simulink library "outp"  (R2021b)
(part 9 of 10)

  VAPM_PASDRML_cm/1 -> VAPM_PASDRML_cm_Inproc/1  "VAPM_PASDRML_cm"
  VAPM_PASDRML_cm_Inproc/1 -> UnitConverter22/1
  UnitConverter22/1 -> VOUTP_PASDRML_cm/1  "VOUTP_PASDRML_cm"
  VAPM_PASDRCR_cm/1 -> VAPM_PASDRCR_cm_Inproc/1  "VAPM_PASDRCR_cm"
  VAPM_PASDRCR_cm_Inproc/1 -> UnitConverter23/1
  UnitConverter23/1 -> VOUTP_PASDRCR_cm/1  "VOUTP_PASDRCR_cm"
  VAPM_PASDRCL_cm/1 -> VAPM_PASDRCL_cm_Inproc/1  "VAPM_PASDRCL_cm"
  VAPM_PASDRCL_cm_Inproc/1 -> UnitConverter24/1
  UnitConverter24/1 -> VOUTP_PASDRCL_cm/1  "VOUTP_PASDRCL_cm"
  VAPM_PASDFMR_cm/1 -> VAPM_PASDFMR_cm_Inproc/1  "VAPM_PASDFMR_cm"
  VAPM_PASDFMR_cm_Inproc/1 -> UnitConverter25/1
  UnitConverter25/1 -> VOUTP_PASDFMR_cm/1  "VOUTP_PASDFMR_cm"
  VAPM_PASDFML_cm/1 -> VAPM_PASDFML_cm_Inproc/1  "VAPM_PASDFML_cm"
  VAPM_PASDFML_cm_Inproc/1 -> UnitConverter26/1
  UnitConverter26/1 -> VOUTP_PASDFML_cm/1  "VOUTP_PASDFML_cm"
  VAPM_PASDFCR_cm/1 -> VAPM_PASDFCR_cm_Inproc/1  "VAPM_PASDFCR_cm"
  VAPM_PASDFCR_cm_Inproc/1 -> UnitConverter27/1
  UnitConverter27/1 -> VOUTP_PASDFCR_cm/1  "VOUTP_PASDFCR_cm"
  VAPM_PASDFCL_cm/1 -> VAPM_PASDFCL_cm_Inproc/1  "VAPM_PASDFCL_cm"
  VAPM_PASDFCL_cm_Inproc/1 -> UnitConverter28/1
  UnitConverter28/1 -> VOUTP_PASDFCL_cm/1  "VOUTP_PASDFCL_cm"
  VAPM_APSDRLR_cm/1 -> VAPM_APSDRLR_cm_Inproc/1  "VAPM_APSDRLR_cm"
  VAPM_APSDRLR_cm_Inproc/1 -> UnitConverter29/1
  UnitConverter29/1 -> VOUTP_APSDRLR_cm/1  "VOUTP_APSDRLR_cm"
  VAPM_APSDRLL_cm/1 -> VAPM_APSDRLL_cm_Inproc/1  "VAPM_APSDRLL_cm"
  VAPM_APSDRLL_cm_Inproc/1 -> UnitConverter30/1
  UnitConverter30/1 -> VOUTP_APSDRLL_cm/1  "VOUTP_APSDRLL_cm"
  VAPM_APSDFLR_cm/1 -> VAPM_APSDFLR_cm_Inproc/1  "VAPM_APSDFLR_cm"
  VAPM_APSDFLR_cm_Inproc/1 -> UnitConverter31/1
  UnitConverter31/1 -> VOUTP_APSDFLR_cm/1  "VOUTP_APSDFLR_cm"
  VAPM_APSDFLL_cm/1 -> VAPM_APSDFLL_cm_Inproc/1  "VAPM_APSDFLL_cm"
  VAPM_APSDFLL_cm_Inproc/1 -> UnitConverter32/1
  UnitConverter32/1 -> VOUTP_APSDFLL_cm/1  "VOUTP_APSDFLL_cm"
  VAPM_PASAFCL_enum/1 -> VAPM_PASAFCL_enum_Inproc/1  "VAPM_PASAFCL_enum"
  VAPM_PASAFCL_enum_Inproc/1 -> UnitConverter33/1
  UnitConverter33/1 -> VOUTP_PASAFCL_enum/1  "VOUTP_PASAFCL_enum"
  VAPM_PASARMR_enum/1 -> VAPM_PASARMR_enum_Inproc/1  "VAPM_PASARMR_enum"
  VAPM_PASARMR_enum_Inproc/1 -> UnitConverter34/1
  UnitConverter34/1 -> VOUTP_PASARMR_enum/1  "VOUTP_PASARMR_enum"
  VAPM_PASARML_enum/1 -> VAPM_PASARML_enum_Inproc/1  "VAPM_PASARML_enum"
  VAPM_PASARML_enum_Inproc/1 -> UnitConverter35/1
  UnitConverter35/1 -> VOUTP_PASARML_enum/1  "VOUTP_PASARML_enum"
  VAPM_PASARCR_enum/1 -> VAPM_PASARCR_enum_Inproc/1  "VAPM_PASARCR_enum"
  VAPM_PASARCR_enum_Inproc/1 -> UnitConverter36/1
  UnitConverter36/1 -> VOUTP_PASARCR_enum/1  "VOUTP_PASARCR_enum"
  VAPM_PASARCL_enum/1 -> VAPM_PASARCL_enum_Inproc/1  "VAPM_PASARCL_enum"
  VAPM_PASARCL_enum_Inproc/1 -> UnitConverter37/1
  UnitConverter37/1 -> VOUTP_PASARCL_enum/1  "VOUTP_PASARCL_enum"
  VAPM_PASAFMR_enum/1 -> VAPM_PASAFMR_enum_Inproc/1  "VAPM_PASAFMR_enum"
  VAPM_PASAFMR_enum_Inproc/1 -> UnitConverter38/1
  UnitConverter38/1 -> VOUTP_PASAFMR_enum/1  "VOUTP_PASAFMR_enum"
  VAPM_PASAFML_enum/1 -> VAPM_PASAFML_enum_Inproc/1  "VAPM_PASAFML_enum"
  VAPM_PASAFML_enum_Inproc/1 -> UnitConverter39/1
  UnitConverter39/1 -> VOUTP_PASAFML_enum/1  "VOUTP_PASAFML_enum"
  VAPM_PASAFCR_enum/1 -> VAPM_PASAFCR_enum_Inproc/1  "VAPM_PASAFCR_enum"
  VAPM_PASAFCR_enum_Inproc/1 -> UnitConverter40/1
  UnitConverter40/1 -> VOUTP_PASAFCR_enum/1  "VOUTP_PASAFCR_enum"
  VAPM_USSStaRMR_flg/1 -> VAPM_USSStaRMR_flg_Inproc/1  "VAPM_USSStaRMR_flg"
  VAPM_USSStaRMR_flg_Inproc/1 -> UnitConverter41/1
  UnitConverter41/1 -> VOUTP_USSStaRMR_flg/1  "VOUTP_USSStaRMR_flg"
  VAPM_USSStaRML_flg/1 -> VAPM_USSStaRML_flg_Inproc/1  "VAPM_USSStaRML_flg"
  VAPM_USSStaRML_flg_Inproc/1 -> UnitConverter42/1
  UnitConverter42/1 -> VOUTP_USSStaRML_flg/1  "VOUTP_USSStaRML_flg"
  VAPM_USSStaRLR_flg/1 -> VAPM_USSStaRLR_flg_Inproc/1  "VAPM_USSStaRLR_flg"
  VAPM_USSStaRLR_flg_Inproc/1 -> UnitConverter43/1
  UnitConverter43/1 -> VOUTP_USSStaRLR_flg/1  "VOUTP_USSStaRLR_flg"
  VAPM_USSStaRLL_flg/1 -> VAPM_USSStaRLL_flg_Inproc/1  "VAPM_USSStaRLL_flg"
  VAPM_USSStaRLL_flg_Inproc/1 -> UnitConverter44/1
  UnitConverter44/1 -> VOUTP_USSStaRLL_flg/1  "VOUTP_USSStaRLL_flg"
  VAPM_USSStaRCR_flg/1 -> VAPM_USSStaRCR_flg_Inproc/1  "VAPM_USSStaRCR_flg"
  VAPM_USSStaRCR_flg_Inproc/1 -> UnitConverter45/1
  UnitConverter45/1 -> VOUTP_USSStaRCR_flg/1  "VOUTP_USSStaRCR_flg"
  VAPM_USSStaRCL_flg/1 -> VAPM_USSStaRCL_flg_Inproc/1  "VAPM_USSStaRCL_flg"
  VAPM_USSStaRCL_flg_Inproc/1 -> UnitConverter46/1
  UnitConverter46/1 -> VOUTP_USSStaRCL_flg/1  "VOUTP_USSStaRCL_flg"
  VAPM_USSStaFMR_flg/1 -> VAPM_USSStaFMR_flg_Inproc/1  "VAPM_USSStaFMR_flg"
  VAPM_USSStaFMR_flg_Inproc/1 -> UnitConverter47/1
  UnitConverter47/1 -> VOUTP_USSStaFMR_flg/1  "VOUTP_USSStaFMR_flg"
  VAPM_USSStaFML_flg/1 -> VAPM_USSStaFML_flg_Inproc/1  "VAPM_USSStaFML_flg"
  VAPM_USSStaFML_flg_Inproc/1 -> UnitConverter48/1
  UnitConverter48/1 -> VOUTP_USSStaFML_flg/1  "VOUTP_USSStaFML_flg"
  VAPM_USSStaFLR_flg/1 -> VAPM_USSStaFLR_flg_Inproc/1  "VAPM_USSStaFLR_flg"
  VAPM_USSStaFLR_flg_Inproc/1 -> UnitConverter49/1
  UnitConverter49/1 -> VOUTP_USSStaFLR_flg/1  "VOUTP_USSStaFLR_flg"
  VAPM_USSStaFLL_flg/1 -> VAPM_USSStaFLL_flg_Inproc/1  "VAPM_USSStaFLL_flg"
  VAPM_USSStaFLL_flg_Inproc/1 -> UnitConverter50/1
  UnitConverter50/1 -> VOUTP_USSStaFLL_flg/1  "VOUTP_USSStaFLL_flg"
  VAPM_USSStaFCR_flg/1 -> VAPM_USSStaFCR_flg_Inproc/1  "VAPM_USSStaFCR_flg"
  VAPM_USSStaFCR_flg_Inproc/1 -> UnitConverter51/1
  UnitConverter51/1 -> VOUTP_USSStaFCR_flg/1  "VOUTP_USSStaFCR_flg"
  VAPM_USSStaFCL_flg/1 -> VAPM_USSStaFCL_flg_Inproc/1  "VAPM_USSStaFCL_flg"
  VAPM_USSStaFCL_flg_Inproc/1 -> UnitConverter52/1
  UnitConverter52/1 -> VOUTP_USSStaFCL_flg/1  "VOUTP_USSStaFCL_flg"
  VAPM_Chime_enum/1 -> VAPM_Chime_enum_Inproc/1  "VAPM_Chime_enum"
  VAPM_Chime_enum_Inproc/1 -> UnitConverter53/1
  UnitConverter53/1 -> VOUTP_Chime_enum/1  "VOUTP_Chime_enum"
  VAPM_SNSRLayout_enum/1 -> VAPM_SNSRLayout_enum_Inproc/1  "VAPM_SNSRLayout_enum"
  VAPM_SNSRLayout_enum_Inproc/1 -> UnitConverter54/1
  UnitConverter54/1 -> VOUTP_SNSRLayout_enum/1  "VOUTP_SNSRLayout_enum"
  VAPM_StaFSya_flg/1 -> VAPM_StaFSya_flg_Inproc/1  "VAPM_StaFSya_flg"
  VAPM_StaFSya_flg_Inproc/1 -> UnitConverter55/1
  UnitConverter55/1 -> VOUTP_StaFSya_flg/1  "VOUTP_StaFSya_flg"
  VAPM_ModOperation_enum/1 -> VAPM_ModOperation_enum_Inproc/1  "VAPM_ModOperation_enum"
  VAPM_ModOperation_enum_Inproc/1 -> UnitConverter56/1
  UnitConverter56/1 -> VOUTP_ModOperation_enum/1  "VOUTP_ModOperation_enum"
  VAPM_BrkPedalPos_pct/1 -> VAPM_BrkPedalPos_pct_Inproc/1  "VAPM_BrkPedalPos_pct"
  VAPM_BrkPedalPos_pct_Inproc/1 -> UnitConverter57/1
  UnitConverter57/1 -> VOUTP_BrkPedalPos_pct/1  "VOUTP_BrkPedalPos_pct"
  VAPM_BrkPedalPosTimeOut_flg/1 -> VAPM_BrkPedalPosTimeOut_flg_Inproc/1  "VAPM_BrkPedalPosTimeOut_flg"
  VAPM_BrkPedalPosTimeOut_flg_Inproc/1 -> UnitConverter58/1
  UnitConverter58/1 -> VOUTP_BrkPedalPosTimeOut_flg/1  "VOUTP_BrkPedalPosTimeOut_flg"
  VAPM_LFRawWhlSpeed_kph/1 -> VAPM_LFRawWhlSpeed_kph_Inproc/1  "VAPM_LFRawWhlSpeed_kph"
  VAPM_LFRawWhlSpeed_kph_Inproc/1 -> UnitConverter59/1
  UnitConverter59/1 -> VOUTP_LFRawWhlSpeed_kph/1  "VOUTP_LFRawWhlSpeed_kph"
  VAPM_LFRawWhlSpeedTimeOut_flg/1 -> VAPM_LFRawWhlSpeedTimeOut_flg_Inproc/1  "VAPM_LFRawWhlSpeedTimeOut_flg"
  VAPM_LFRawWhlSpeedTimeOut_flg_Inproc/1 -> UnitConverter60/1
  UnitConverter60/1 -> VOUTP_LFRawWhlSpeedTimeOut_flg/1  "VOUTP_LFRawWhlSpeedTimeOut_flg"
  VAPM_RFRawWhlSpeed_kph/1 -> VAPM_RFRawWhlSpeed_kph_Inproc/1  "VAPM_RFRawWhlSpeed_kph"
  VAPM_RFRawWhlSpeed_kph_Inproc/1 -> UnitConverter61/1
  UnitConverter61/1 -> VOUTP_RFRawWhlSpeed_kph/1  "VOUTP_RFRawWhlSpeed_kph"
  VAPM_RFRawWhlSpeedTimeOut_flg/1 -> VAPM_RFRawWhlSpeedTimeOut_flg_Inproc/1  "VAPM_RFRawWhlSpeedTimeOut_flg"
  VAPM_RFRawWhlSpeedTimeOut_flg_Inproc/1 -> UnitConverter62/1
  UnitConverter62/1 -> VOUTP_RFRawWhlSpeedTimeOut_flg/1  "VOUTP_RFRawWhlSpeedTimeOut_flg"
  VAPM_LRRawWhlSpeed_kph/1 -> VAPM_LRRawWhlSpeed_kph_Inproc/1  "VAPM_LRRawWhlSpeed_kph"
  VAPM_LRRawWhlSpeed_kph_Inproc/1 -> UnitConverter63/1
  UnitConverter63/1 -> VOUTP_LRRawWhlSpeed_kph/1  "VOUTP_LRRawWhlSpeed_kph"
  VAPM_LRRawWhlSpeedTimeOut_flg/1 -> VAPM_LRRawWhlSpeedTimeOut_flg_Inproc/1  "VAPM_LRRawWhlSpeedTimeOut_flg"
  VAPM_LRRawWhlSpeedTimeOut_flg_Inproc/1 -> UnitConverter64/1
  UnitConverter64/1 -> VOUTP_LRRawWhlSpeedTimeOut_flg/1  "VOUTP_LRRawWhlSpeedTimeOut_flg"
  VAPM_RRRawWhlSpeed_kph/1 -> VAPM_RRRawWhlSpeed_kph_Inproc/1  "VAPM_RRRawWhlSpeed_kph"
  VAPM_RRRawWhlSpeed_kph_Inproc/1 -> UnitConverter65/1
  UnitConverter65/1 -> VOUTP_RRRawWhlSpeed_kph/1  "VOUTP_RRRawWhlSpeed_kph"
  VAPM_RRRawWhlSpeedTimeOut_flg/1 -> VAPM_RRRawWhlSpeedTimeOut_flg_Inproc/1  "VAPM_RRRawWhlSpeedTimeOut_flg"
  VAPM_RRRawWhlSpeedTimeOut_flg_Inproc/1 -> UnitConverter66/1
  UnitConverter66/1 -> VOUTP_RRRawWhlSpeedTimeOut_flg/1  "VOUTP_RRRawWhlSpeedTimeOut_flg"
  VAPM_LFRawWhlSpeedV_flg/1 -> VAPM_LFRawWhlSpeedV_flg_Inproc/1  "VAPM_LFRawWhlSpeedV_flg"
  VAPM_LFRawWhlSpeedV_flg_Inproc/1 -> UnitConverter67/1
  UnitConverter67/1 -> VOUTP_LFRawWhlSpeedV_flg/1  "VOUTP_LFRawWhlSpeedV_flg"
  VAPM_LFRawWhlSpeedVTimeOut_flg/1 -> VAPM_LFRawWhlSpeedVTimeOut_flg_Inproc/1  "VAPM_LFRawWhlSpeedVTimeOut_flg"
  VAPM_LFRawWhlSpeedVTimeOut_flg_Inproc/1 -> UnitConverter68/1
  UnitConverter68/1 -> VOUTP_LFRawWhlSpeedVTimeOut_flg/1  "VOUTP_LFRawWhlSpeedVTimeOut_flg"
  VAPM_RFRawWhlSpeedV_flg/1 -> VAPM_RFRawWhlSpeedV_flg_Inproc/1  "VAPM_RFRawWhlSpeedV_flg"
  VAPM_RFRawWhlSpeedV_flg_Inproc/1 -> UnitConverter69/1
  UnitConverter69/1 -> VOUTP_RFRawWhlSpeedV_flg/1  "VOUTP_RFRawWhlSpeedV_flg"
  VAPM_RFRawWhlSpeedVTimeOut_flg/1 -> VAPM_RFRawWhlSpeedVTimeOut_flg_Inproc/1  "VAPM_RFRawWhlSpeedVTimeOut_flg"
  VAPM_RFRawWhlSpeedVTimeOut_flg_Inproc/1 -> UnitConverter70/1
  UnitConverter70/1 -> VOUTP_RFRawWhlSpeedVTimeOut_flg/1  "VOUTP_RFRawWhlSpeedVTimeOut_flg"
  VAPM_LRRawWhlSpeedV_flg/1 -> VAPM_LRRawWhlSpeedV_flg_Inproc/1  "VAPM_LRRawWhlSpeedV_flg"
  VAPM_LRRawWhlSpeedV_flg_Inproc/1 -> UnitConverter71/1
  UnitConverter71/1 -> VOUTP_LRRawWhlSpeedV_flg/1  "VOUTP_LRRawWhlSpeedV_flg"
  VAPM_LRRawWhlSpeedVTimeOut_flg/1 -> VAPM_LRRawWhlSpeedVTimeOut_flg_Inproc/1  "VAPM_LRRawWhlSpeedVTimeOut_flg"
  VAPM_LRRawWhlSpeedVTimeOut_flg_Inproc/1 -> UnitConverter72/1
  UnitConverter72/1 -> VOUTP_LRRawWhlSpeedVTimeOut_flg/1  "VOUTP_LRRawWhlSpeedVTimeOut_flg"
  VAPM_RRRawWhlSpeedV_flg/1 -> VAPM_RRRawWhlSpeedV_flg_Inproc/1  "VAPM_RRRawWhlSpeedV_flg"
  VAPM_RRRawWhlSpeedV_flg_Inproc/1 -> UnitConverter73/1
  UnitConverter73/1 -> VOUTP_RRRawWhlSpeedV_flg/1  "VOUTP_RRRawWhlSpeedV_flg"
  VAPM_RRRawWhlSpeedVTimeOut_flg/1 -> VAPM_RRRawWhlSpeedVTimeOut_flg_Inproc/1  "VAPM_RRRawWhlSpeedVTimeOut_flg"
  VAPM_RRRawWhlSpeedVTimeOut_flg_Inproc/1 -> UnitConverter74/1
  UnitConverter74/1 -> VOUTP_RRRawWhlSpeedVTimeOut_flg/1  "VOUTP_RRRawWhlSpeedVTimeOut_flg"
  VAPM_LFWhlRotDir_enum/1 -> VAPM_LFWhlRotDir_enum_Inproc/1  "VAPM_LFWhlRotDir_enum"
  VAPM_LFWhlRotDir_enum_Inproc/1 -> UnitConverter75/1
  UnitConverter75/1 -> VOUTP_LFWhlRotDir_enum/1  "VOUTP_LFWhlRotDir_enum"
  VAPM_LFWhlRotDirTimeOut_flg/1 -> VAPM_LFWhlRotDirTimeOut_flg_Inproc/1  "VAPM_LFWhlRotDirTimeOut_flg"
  VAPM_LFWhlRotDirTimeOut_flg_Inproc/1 -> UnitConverter76/1
  UnitConverter76/1 -> VOUTP_LFWhlRotDirTimeOut_flg/1  "VOUTP_LFWhlRotDirTimeOut_flg"
  VAPM_RFWhlRotDir_enum/1 -> VAPM_RFWhlRotDir_enum_Inproc/1  "VAPM_RFWhlRotDir_enum"
  VAPM_RFWhlRotDir_enum_Inproc/1 -> UnitConverter77/1
  UnitConverter77/1 -> VOUTP_RFWhlRotDir_enum/1  "VOUTP_RFWhlRotDir_enum"
  VAPM_RFWhlRotDirTimeOut_flg/1 -> VAPM_RFWhlRotDirTimeOut_flg_Inproc/1  "VAPM_RFWhlRotDirTimeOut_flg"
  VAPM_RFWhlRotDirTimeOut_flg_Inproc/1 -> UnitConverter78/1
  UnitConverter78/1 -> VOUTP_RFWhlRotDirTimeOut_flg/1  "VOUTP_RFWhlRotDirTimeOut_flg"
  VAPM_LRWhlRotDir_enum/1 -> VAPM_LRWhlRotDir_enum_Inproc/1  "VAPM_LRWhlRotDir_enum"
  VAPM_LRWhlRotDir_enum_Inproc/1 -> UnitConverter79/1
  UnitConverter79/1 -> VOUTP_LRWhlRotDir_enum/1  "VOUTP_LRWhlRotDir_enum"
  VAPM_LRWhlRotDirTimeOut_flg/1 -> VAPM_LRWhlRotDirTimeOut_flg_Inproc/1  "VAPM_LRWhlRotDirTimeOut_flg"
  VAPM_LRWhlRotDirTimeOut_flg_Inproc/1 -> UnitConverter80/1
  UnitConverter80/1 -> VOUTP_LRWhlRotDirTimeOut_flg/1  "VOUTP_LRWhlRotDirTimeOut_flg"
  VAPM_RRWhlRotDir_enum/1 -> VAPM_RRWhlRotDir_enum_Inproc/1  "VAPM_RRWhlRotDir_enum"
  VAPM_RRWhlRotDir_enum_Inproc/1 -> UnitConverter81/1
  UnitConverter81/1 -> VOUTP_RRWhlRotDir_enum/1  "VOUTP_RRWhlRotDir_enum"
  VAPM_RRWhlRotDirTimeOut_flg/1 -> VAPM_RRWhlRotDirTimeOut_flg_Inproc/1  "VAPM_RRWhlRotDirTimeOut_flg"
  VAPM_RRWhlRotDirTimeOut_flg_Inproc/1 -> UnitConverter82/1
  UnitConverter82/1 -> VOUTP_RRWhlRotDirTimeOut_flg/1  "VOUTP_RRWhlRotDirTimeOut_flg"
  VAPM_LFPulseCountV_flg/1 -> VAPM_LFPulseCountV_flg_Inproc/1  "VAPM_LFPulseCountV_flg"
  VAPM_LFPulseCountV_flg_Inproc/1 -> UnitConverter83/1
  UnitConverter83/1 -> VOUTP_LFPulseCountV_flg/1  "VOUTP_LFPulseCountV_flg"
  VAPM_LFPulseCountVTimeOut_flg/1 -> VAPM_LFPulseCountVTimeOut_flg_Inproc/1  "VAPM_LFPulseCountVTimeOut_flg"
  VAPM_LFPulseCountVTimeOut_flg_Inproc/1 -> UnitConverter84/1
  UnitConverter84/1 -> VOUTP_LFPulseCountVTimeOut_flg/1  "VOUTP_LFPulseCountVTimeOut_flg"
  VAPM_RFPulseCountV_flg/1 -> VAPM_RFPulseCountV_flg_Inproc/1  "VAPM_RFPulseCountV_flg"
  VAPM_RFPulseCountV_flg_Inproc/1 -> UnitConverter85/1
  UnitConverter85/1 -> VOUTP_RFPulseCountV_flg/1  "VOUTP_RFPulseCountV_flg"
  VAPM_RFPulseCountVTimeOut_flg/1 -> VAPM_RFPulseCountVTimeOut_flg_Inproc/1  "VAPM_RFPulseCountVTimeOut_flg"
  VAPM_RFPulseCountVTimeOut_flg_Inproc/1 -> UnitConverter86/1
  UnitConverter86/1 -> VOUTP_RFPulseCountVTimeOut_flg/1  "VOUTP_RFPulseCountVTimeOut_flg"
  VAPM_LRPulseCountV_flg/1 -> VAPM_LRPulseCountV_flg_Inproc/1  "VAPM_LRPulseCountV_flg"
  VAPM_LRPulseCountV_flg_Inproc/1 -> UnitConverter87/1
  UnitConverter87/1 -> VOUTP_LRPulseCountV_flg/1  "VOUTP_LRPulseCountV_flg"
  VAPM_LRPulseCountVTimeOut_flg/1 -> VAPM_LRPulseCountVTimeOut_flg_Inproc/1  "VAPM_LRPulseCountVTimeOut_flg"
  VAPM_LRPulseCountVTimeOut_flg_Inproc/1 -> UnitConverter88/1
  UnitConverter88/1 -> VOUTP_LRPulseCountVTimeOut_flg/1  "VOUTP_LRPulseCountVTimeOut_flg"
  VAPM_RRPulseCountV_flg/1 -> VAPM_RRPulseCountV_flg_Inproc/1  "VAPM_RRPulseCountV_flg"
  VAPM_RRPulseCountV_flg_Inproc/1 -> UnitConverter89/1
  UnitConverter89/1 -> VOUTP_RRPulseCountV_flg/1  "VOUTP_RRPulseCountV_flg"
  VAPM_RRPulseCountVTimeOut_flg/1 -> VAPM_RRPulseCountVTimeOut_flg_Inproc/1  "VAPM_RRPulseCountVTimeOut_flg"
  VAPM_RRPulseCountVTimeOut_flg_Inproc/1 -> UnitConverter90/1
  UnitConverter90/1 -> VOUTP_RRPulseCountVTimeOut_flg/1  "VOUTP_RRPulseCountVTimeOut_flg"
  VAPM_LFPulseCount_enum/1 -> VAPM_LFPulseCount_enum_Inproc/1  "VAPM_LFPulseCount_enum"
  VAPM_LFPulseCount_enum_Inproc/1 -> UnitConverter91/1
  UnitConverter91/1 -> VOUTP_LFPulseCount_enum/1  "VOUTP_LFPulseCount_enum"
  VAPM_LFPulseCountTimeOut_flg/1 -> VAPM_LFPulseCountTimeOut_flg_Inproc/1  "VAPM_LFPulseCountTimeOut_flg"
  VAPM_LFPulseCountTimeOut_flg_Inproc/1 -> UnitConverter92/1
  UnitConverter92/1 -> VOUTP_LFPulseCountTimeOut_flg/1  "VOUTP_LFPulseCountTimeOut_flg"
  VAPM_RFPulseCount_enum/1 -> VAPM_RFPulseCount_enum_Inproc/1  "VAPM_RFPulseCount_enum"
  VAPM_RFPulseCount_enum_Inproc/1 -> UnitConverter93/1
  UnitConverter93/1 -> VOUTP_RFPulseCount_enum/1  "VOUTP_RFPulseCount_enum"
  VAPM_RFPulseCountTimeOut_flg/1 -> VAPM_RFPulseCountTimeOut_flg_Inproc/1  "VAPM_RFPulseCountTimeOut_flg"
  VAPM_RFPulseCountTimeOut_flg_Inproc/1 -> UnitConverter94/1
  UnitConverter94/1 -> VOUTP_RFPulseCountTimeOut_flg/1  "VOUTP_RFPulseCountTimeOut_flg"
  VAPM_LRPulseCount_enum/1 -> VAPM_LRPulseCount_enum_Inproc/1  "VAPM_LRPulseCount_enum"
  VAPM_LRPulseCount_enum_Inproc/1 -> UnitConverter95/1
  UnitConverter95/1 -> VOUTP_LRPulseCount_enum/1  "VOUTP_LRPulseCount_enum"
  VAPM_LRPulseCountTimeOut_flg/1 -> VAPM_LRPulseCountTimeOut_flg_Inproc/1  "VAPM_LRPulseCountTimeOut_flg"
  VAPM_LRPulseCountTimeOut_flg_Inproc/1 -> UnitConverter96/1
  UnitConverter96/1 -> VOUTP_LRPulseCountTimeOut_flg/1  "VOUTP_LRPulseCountTimeOut_flg"
  VAPM_RRPulseCount_enum/1 -> VAPM_RRPulseCount_enum_Inproc/1  "VAPM_RRPulseCount_enum"
  VAPM_RRPulseCount_enum_Inproc/1 -> UnitConverter97/1
  UnitConverter97/1 -> VOUTP_RRPulseCount_enum/1  "VOUTP_RRPulseCount_enum"
  VAPM_RRPulseCountTimeOut_flg/1 -> VAPM_RRPulseCountTimeOut_flg_Inproc/1  "VAPM_RRPulseCountTimeOut_flg"
  VAPM_RRPulseCountTimeOut_flg_Inproc/1 -> UnitConverter98/1
  UnitConverter98/1 -> VOUTP_RRPulseCountTimeOut_flg/1  "VOUTP_RRPulseCountTimeOut_flg"
  VAPM_ShifterHandleCmd_enum/1 -> VAPM_ShifterHandleCmd_enum_Inproc/1  "VAPM_ShifterHandleCmd_enum"
  VAPM_ShifterHandleCmd_enum_Inproc/1 -> UnitConverter99/1
  UnitConverter99/1 -> VOUTP_ShifterHandleCmd_enum/1  "VOUTP_ShifterHandleCmd_enum"
  VAPM_ShifterHandleCmdTimeOut_flg/1 -> VAPM_ShifterHandleCmdTimeOut_flg_Inproc/1  "VAPM_ShifterHandleCmdTimeOut_flg"
  VAPM_ShifterHandleCmdTimeOut_flg_Inproc/1 -> UnitConverter100/1
  UnitConverter100/1 -> VOUTP_ShifterHandleCmdTimeOut_flg/1  "VOUTP_ShifterHandleCmdTimeOut_flg"
  VAPM_DriIntend_enum/1 -> VAPM_DriIntend_enum_Inproc/1  "VAPM_DriIntend_enum"
  VAPM_DriIntend_enum_Inproc/1 -> UnitConverter101/1
  UnitConverter101/1 -> VOUTP_DriIntend_enum/1  "VOUTP_DriIntend_enum"
  VAPM_DriIntendTimeOut_flg/1 -> VAPM_DriIntendTimeOut_flg_Inproc/1  "VAPM_DriIntendTimeOut_flg"
  VAPM_DriIntendTimeOut_flg_Inproc/1 -> UnitConverter102/1
  UnitConverter102/1 -> VOUTP_DriIntendTimeOut_flg/1  "VOUTP_DriIntendTimeOut_flg"
  VAPM_EPSAOIControl_enum/1 -> VAPM_EPSAOIControl_enum_Inproc/1  "VAPM_EPSAOIControl_enum"
  VAPM_EPSAOIControl_enum_Inproc/1 -> UnitConverter103/1
  UnitConverter103/1 -> VOUTP_EPSAOIControl_enum/1  "VOUTP_EPSAOIControl_enum"
  VAPM_EPSAOIControlTimeOut_flg/1 -> VAPM_EPSAOIControlTimeOut_flg_Inproc/1  "VAPM_EPSAOIControlTimeOut_flg"
  VAPM_EPSAOIControlTimeOut_flg_Inproc/1 -> UnitConverter104/1
  UnitConverter104/1 -> VOUTP_EPSAOIControlTimeOut_flg/1  "VOUTP_EPSAOIControlTimeOut_flg"
  VAPM_SASAngle_Deg/1 -> VAPM_SASAngle_Deg_Inproc/1  "VAPM_SASAngle_Deg"
  VAPM_SASAngle_Deg_Inproc/1 -> UnitConverter105/1
  UnitConverter105/1 -> VOUTP_SASAngle_Deg/1  "VOUTP_SASAngle_Deg"
  VAPM_SASAngleTimeOut_flg/1 -> VAPM_SASAngleTimeOut_flg_Inproc/1  "VAPM_SASAngleTimeOut_flg"
  VAPM_SASAngleTimeOut_flg_Inproc/1 -> UnitConverter106/1
  UnitConverter106/1 -> VOUTP_SASAngleTimeOut_flg/1  "VOUTP_SASAngleTimeOut_flg"
  VAPM_SASSpeed_degps/1 -> VAPM_SASSpeed_degps_Inproc/1  "VAPM_SASSpeed_degps"
  VAPM_SASSpeed_degps_Inproc/1 -> UnitConverter107/1
  UnitConverter107/1 -> VOUTP_SASSpeed_degps/1  "VOUTP_SASSpeed_degps"
  VAPM_SASSpeedTimeOut_flg/1 -> VAPM_SASSpeedTimeOut_flg_Inproc/1  "VAPM_SASSpeedTimeOut_flg"
  VAPM_SASSpeedTimeOut_flg_Inproc/1 -> UnitConverter108/1
  UnitConverter108/1 -> VOUTP_SASSpeedTimeOut_flg/1  "VOUTP_SASSpeedTimeOut_flg"
  VAPM_SASSpeedValid_flg/1 -> VAPM_SASSpeedValid_flg_Inproc/1  "VAPM_SASSpeedValid_flg"
  VAPM_SASSpeedValid_flg_Inproc/1 -> UnitConverter109/1
  UnitConverter109/1 -> VOUTP_SASSpeedValid_flg/1  "VOUTP_SASSpeedValid_flg"
  VAPM_SASSpeedValidTimeOut_flg/1 -> VAPM_SASSpeedValidTimeOut_flg_Inproc/1  "VAPM_SASSpeedValidTimeOut_flg"
  VAPM_SASSpeedValidTimeOut_flg_Inproc/1 -> UnitConverter110/1
  UnitConverter110/1 -> VOUTP_SASSpeedValidTimeOut_flg/1  "VOUTP_SASSpeedValidTimeOut_flg"
  VAPM_SASCAL_flg/1 -> VAPM_SASCAL_flg_Inproc/1  "VAPM_SASCAL_flg"
  VAPM_SASCAL_flg_Inproc/1 -> UnitConverter111/1
  UnitConverter111/1 -> VOUTP_SASCAL_flg/1  "VOUTP_SASCAL_flg"
  VAPM_SASCALTimeOut_flg/1 -> VAPM_SASCALTimeOut_flg_Inproc/1  "VAPM_SASCALTimeOut_flg"
  VAPM_SASCALTimeOut_flg_Inproc/1 -> UnitConverter112/1
  UnitConverter112/1 -> VOUTP_SASCALTimeOut_flg/1  "VOUTP_SASCALTimeOut_flg"
  VAPM_SASV_flg/1 -> VAPM_SASV_flg_Inproc/1  "VAPM_SASV_flg"
  VAPM_SASV_flg_Inproc/1 -> UnitConverter113/1
  UnitConverter113/1 -> VOUTP_SASV_flg/1  "VOUTP_SASV_flg"
  VAPM_SASVTimeOut_flg/1 -> VAPM_SASVTimeOut_flg_Inproc/1  "VAPM_SASVTimeOut_flg"
  VAPM_SASVTimeOut_flg_Inproc/1 -> UnitConverter114/1
  UnitConverter114/1 -> VOUTP_SASVTimeOut_flg/1  "VOUTP_SASVTimeOut_flg"
  VAPM_GRADE_Deg/1 -> VAPM_GRADE_Deg_Inproc/1  "VAPM_GRADE_Deg"
  VAPM_GRADE_Deg_Inproc/1 -> UnitConverter115/1
  UnitConverter115/1 -> VOUTP_GRADE_Deg/1  "VOUTP_GRADE_Deg"
  VAPM_GRADETimeOut_flg/1 -> VAPM_GRADETimeOut_flg_Inproc/1  "VAPM_GRADETimeOut_flg"
  VAPM_GRADETimeOut_flg_Inproc/1 -> UnitConverter116/1
  UnitConverter116/1 -> VOUTP_GRADETimeOut_flg/1  "VOUTP_GRADETimeOut_flg"
  VAPM_YawRate_degps/1 -> VAPM_YawRate_degps_Inproc/1  "VAPM_YawRate_degps"
  VAPM_YawRate_degps_Inproc/1 -> UnitConverter117/1
  UnitConverter117/1 -> VOUTP_YawRate_degps/1  "VOUTP_YawRate_degps"
  VAPM_YawRateTimeOut_flg/1 -> VAPM_YawRateTimeOut_flg_Inproc/1  "VAPM_YawRateTimeOut_flg"
  VAPM_YawRateTimeOut_flg_Inproc/1 -> UnitConverter118/1
  UnitConverter118/1 -> VOUTP_YawRateTimeOut_flg/1  "VOUTP_YawRateTimeOut_flg"
  VAPM_LatAccel_Gps/1 -> VAPM_LatAccel_Gps_Inproc/1  "VAPM_LatAccel_Gps"
  VAPM_LatAccel_Gps_Inproc/1 -> UnitConverter119/1
  UnitConverter119/1 -> VOUTP_LatAccel_Gps/1  "VOUTP_LatAccel_Gps"
  VAPM_LatAccelTimeOut_flg/1 -> VAPM_LatAccelTimeOut_flg_Inproc/1  "VAPM_LatAccelTimeOut_flg"
  VAPM_LatAccelTimeOut_flg_Inproc/1 -> UnitConverter120/1
  UnitConverter120/1 -> VOUTP_LatAccelTimeOut_flg/1  "VOUTP_LatAccelTimeOut_flg"
  VAPM_LongAccel_Gps/1 -> VAPM_LongAccel_Gps_Inproc/1  "VAPM_LongAccel_Gps"
  VAPM_LongAccel_Gps_Inproc/1 -> UnitConverter121/1
  UnitConverter121/1 -> VOUTP_LongAccel_Gps/1  "VOUTP_LongAccel_Gps"
  VAPM_LongAccelTimeOut_flg/1 -> VAPM_LongAccelTimeOut_flg_Inproc/1  "VAPM_LongAccelTimeOut_flg"
  VAPM_LongAccelTimeOut_flg_Inproc/1 -> UnitConverter122/1
  UnitConverter122/1 -> VOUTP_LongAccelTimeOut_flg/1  "VOUTP_LongAccelTimeOut_flg"
  VAPM_MCPressure_bar/1 -> VAPM_MCPressure_bar_Inproc/1  "VAPM_MCPressure_bar"
  VAPM_MCPressure_bar_Inproc/1 -> UnitConverter123/1
  UnitConverter123/1 -> VOUTP_MCPressure_bar/1  "VOUTP_MCPressure_bar"
  VAPM_MCPressureTimeOut_flg/1 -> VAPM_MCPressureTimeOut_flg_Inproc/1  "VAPM_MCPressureTimeOut_flg"
  VAPM_MCPressureTimeOut_flg_Inproc/1 -> UnitConverter124/1
  UnitConverter124/1 -> VOUTP_MCPressureTimeOut_flg/1  "VOUTP_MCPressureTimeOut_flg"
  VAPM_YawRateV_flg/1 -> VAPM_YawRateV_flg_Inproc/1  "VAPM_YawRateV_flg"
  VAPM_YawRateV_flg_Inproc/1 -> UnitConverter125/1
  UnitConverter125/1 -> VOUTP_YawRateV_flg/1  "VOUTP_YawRateV_flg"
  VAPM_YawRateVTimeOut_flg/1 -> VAPM_YawRateVTimeOut_flg_Inproc/1  "VAPM_YawRateVTimeOut_flg"
  VAPM_YawRateVTimeOut_flg_Inproc/1 -> UnitConverter126/1
  UnitConverter126/1 -> VOUTP_YawRateVTimeOut_flg/1  "VOUTP_YawRateVTimeOut_flg"
  VAPM_LatAccelV_flg/1 -> VAPM_LatAccelV_flg_Inproc/1  "VAPM_LatAccelV_flg"
  VAPM_LatAccelV_flg_Inproc/1 -> UnitConverter127/1
  UnitConverter127/1 -> VOUTP_LatAccelV_flg/1  "VOUTP_LatAccelV_flg"
  VAPM_LatAccelVTimeOut_flg/1 -> VAPM_LatAccelVTimeOut_flg_Inproc/1  "VAPM_LatAccelVTimeOut_flg"
  VAPM_LatAccelVTimeOut_flg_Inproc/1 -> UnitConverter128/1
  UnitConverter128/1 -> VOUTP_LatAccelVTimeOut_flg/1  "VOUTP_LatAccelVTimeOut_flg"
  VAPM_LongAccelV_flg/1 -> VAPM_LongAccelV_flg_Inproc/1  "VAPM_LongAccelV_flg"
  VAPM_LongAccelV_flg_Inproc/1 -> UnitConverter129/1
  UnitConverter129/1 -> VOUTP_LongAccelV_flg/1  "VOUTP_LongAccelV_flg"
  VAPM_LongAccelVTimeOut_flg/1 -> VAPM_LongAccelVTimeOut_flg_Inproc/1  "VAPM_LongAccelVTimeOut_flg"
  VAPM_LongAccelVTimeOut_flg_Inproc/1 -> UnitConverter130/1
  UnitConverter130/1 -> VOUTP_LongAccelVTimeOut_flg/1  "VOUTP_LongAccelVTimeOut_flg"
  VAPM_MCPressureV_bar/1 -> VAPM_MCPressureV_bar_Inproc/1  "VAPM_MCPressureV_bar"
  VAPM_MCPressureV_bar_Inproc/1 -> UnitConverter131/1
  UnitConverter131/1 -> VOUTP_MCPressureV_bar/1  "VOUTP_MCPressureV_bar"
  VAPM_MCPressureVTimeOut_flg/1 -> VAPM_MCPressureVTimeOut_flg_Inproc/1  "VAPM_MCPressureVTimeOut_flg"
  VAPM_MCPressureVTimeOut_flg_Inproc/1 -> UnitConverter132/1
  UnitConverter132/1 -> VOUTP_MCPressureVTimeOut_flg/1  "VOUTP_MCPressureVTimeOut_flg"
  VAPM_BrkSwSta_flg/1 -> VAPM_BrkSwSta_flg_Inproc/1  "VAPM_BrkSwSta_flg"
  VAPM_BrkSwSta_flg_Inproc/1 -> UnitConverter133/1
  UnitConverter133/1 -> VOUTP_BrkSwSta_flg/1  "VOUTP_BrkSwSta_flg"
  VAPM_BrkSwStaTimeOut_flg/1 -> VAPM_BrkSwStaTimeOut_flg_Inproc/1  "VAPM_BrkSwStaTimeOut_flg"
  VAPM_BrkSwStaTimeOut_flg_Inproc/1 -> UnitConverter134/1
  UnitConverter134/1 -> VOUTP_BrkSwStaTimeOut_flg/1  "VOUTP_BrkSwStaTimeOut_flg"
  VAPM_BrkSwV_flg/1 -> VAPM_BrkSwV_flg_Inproc/1  "VAPM_BrkSwV_flg"
  VAPM_BrkSwV_flg_Inproc/1 -> UnitConverter135/1
  UnitConverter135/1 -> VOUTP_BrkSwV_flg/1  "VOUTP_BrkSwV_flg"
  VAPM_BrkSwVTimeOut_flg/1 -> VAPM_BrkSwVTimeOut_flg_Inproc/1  "VAPM_BrkSwVTimeOut_flg"
  VAPM_BrkSwVTimeOut_flg_Inproc/1 -> UnitConverter136/1
  UnitConverter136/1 -> VOUTP_BrkSwVTimeOut_flg/1  "VOUTP_BrkSwVTimeOut_flg"
  VAPM_ESCStandstill_flg/1 -> VAPM_ESCStandstill_flg_Inproc/1  "VAPM_ESCStandstill_flg"
  VAPM_ESCStandstill_flg_Inproc/1 -> UnitConverter137/1
  UnitConverter137/1 -> VOUTP_ESCStandstill_flg/1  "VOUTP_ESCStandstill_flg"
  VAPM_ESCStandstillTimeOut_flg/1 -> VAPM_ESCStandstillTimeOut_flg_Inproc/1  "VAPM_ESCStandstillTimeOut_flg"
  VAPM_ESCStandstillTimeOut_flg_Inproc/1 -> UnitConverter138/1
  UnitConverter138/1 -> VOUTP_ESCStandstillTimeOut_flg/1  "VOUTP_ESCStandstillTimeOut_flg"
  VAPM_ESCAPSSta_enum/1 -> VAPM_ESCAPSSta_enum_Inproc/1  "VAPM_ESCAPSSta_enum"
  VAPM_ESCAPSSta_enum_Inproc/1 -> UnitConverter139/1
  UnitConverter139/1 -> VOUTP_ESCAPSSta_enum/1  "VOUTP_ESCAPSSta_enum"
  VAPM_ESCAPSStaTimeOut_flg/1 -> VAPM_ESCAPSStaTimeOut_flg_Inproc/1  "VAPM_ESCAPSStaTimeOut_flg"
  VAPM_ESCAPSStaTimeOut_flg_Inproc/1 -> UnitConverter140/1
  UnitConverter140/1 -> VOUTP_ESCAPSStaTimeOut_flg/1  "VOUTP_ESCAPSStaTimeOut_flg"
  VAPM_EPBExtReleaseAvail_flg/1 -> VAPM_EPBExtReleaseAvail_flg_Inproc/1  "VAPM_EPBExtReleaseAvail_flg"
  VAPM_EPBExtReleaseAvail_flg_Inproc/1 -> UnitConverter141/1
  UnitConverter141/1 -> VOUTP_EPBExtReleaseAvail_flg/1  "VOUTP_EPBExtReleaseAvail_flg"
  VAPM_EPBExtReleaseAvailTimeOut_flg/1 -> VAPM_EPBExtReleaseAvailTimeOut_flg_Inproc/1  "VAPM_EPBExtReleaseAvailTimeOut_flg"
  VAPM_EPBExtReleaseAvailTimeOut_flg_Inproc/1 -> UnitConverter142/1
  UnitConverter142/1 -> VOUTP_EPBExtReleaseAvailTimeOut_flg/1  "VOUTP_EPBExtReleaseAvailTimeOut_flg"
  VAPM_EPBExtApplyAvail_flg/1 -> VAPM_EPBExtApplyAvail_flg_Inproc/1  "VAPM_EPBExtApplyAvail_flg"
  VAPM_EPBExtApplyAvail_flg_Inproc/1 -> UnitConverter143/1
  UnitConverter143/1 -> VOUTP_EPBExtApplyAvail_flg/1  "VOUTP_EPBExtApplyAvail_flg"
  VAPM_EPBExtApplyAvailTimeOut_flg/1 -> VAPM_EPBExtApplyAvailTimeOut_flg_Inproc/1  "VAPM_EPBExtApplyAvailTimeOut_flg"
  VAPM_EPBExtApplyAvailTimeOut_flg_Inproc/1 -> UnitConverter144/1
  UnitConverter144/1 -> VOUTP_EPBExtApplyAvailTimeOut_flg/1  "VOUTP_EPBExtApplyAvailTimeOut_flg"
  VAPM_EPBErrSta_enum/1 -> VAPM_EPBErrSta_enum_Inproc/1  "VAPM_EPBErrSta_enum"
  VAPM_EPBErrSta_enum_Inproc/1 -> UnitConverter145/1
  UnitConverter145/1 -> VOUTP_EPBErrSta_enum/1  "VOUTP_EPBErrSta_enum"
  VAPM_EPBErrStaTimeOut_flg/1 -> VAPM_EPBErrStaTimeOut_flg_Inproc/1  "VAPM_EPBErrStaTimeOut_flg"
  VAPM_EPBErrStaTimeOut_flg_Inproc/1 -> UnitConverter146/1
  UnitConverter146/1 -> VOUTP_EPBErrStaTimeOut_flg/1  "VOUTP_EPBErrStaTimeOut_flg"
  VAPM_EPBSta_enum/1 -> VAPM_EPBSta_enum_Inproc/1  "VAPM_EPBSta_enum"
  VAPM_EPBSta_enum_Inproc/1 -> UnitConverter147/1
  UnitConverter147/1 -> VOUTP_EPBSta_enum/1  "VOUTP_EPBSta_enum"
  VAPM_EPBStaTimeOut_flg/1 -> VAPM_EPBStaTimeOut_flg_Inproc/1  "VAPM_EPBStaTimeOut_flg"
  VAPM_EPBStaTimeOut_flg_Inproc/1 -> UnitConverter148/1
  UnitConverter148/1 -> VOUTP_EPBStaTimeOut_flg/1  "VOUTP_EPBStaTimeOut_flg"
  VAPM_AVMparkingcancel_enum/1 -> VAPM_AVMparkingcancel_enum_Inproc/1  "VAPM_AVMparkingcancel_enum"
  VAPM_AVMparkingcancel_enum_Inproc/1 -> UnitConverter149/1
  UnitConverter149/1 -> VOUTP_AVMparkingcancel_enum/1  "VOUTP_AVMparkingcancel_enum"
  VAPM_AVMparkingcancelTimeOut_flg/1 -> VAPM_AVMparkingcancelTimeOut_flg_Inproc/1  "VAPM_AVMparkingcancelTimeOut_flg"
  VAPM_AVMparkingcancelTimeOut_flg_Inproc/1 -> UnitConverter150/1
  UnitConverter150/1 -> VOUTP_AVMparkingcancelTimeOut_flg/1  "VOUTP_AVMparkingcancelTimeOut_flg"
  VAPM_AVMparkingexcute_enum/1 -> VAPM_AVMparkingexcute_enum_Inproc/1  "VAPM_AVMparkingexcute_enum"
  VAPM_AVMparkingexcute_enum_Inproc/1 -> UnitConverter151/1
  UnitConverter151/1 -> VOUTP_AVMparkingexcute_enum/1  "VOUTP_AVMparkingexcute_enum"
  VAPM_AVMparkingexcuteTimeOut_flg/1 -> VAPM_AVMparkingexcuteTimeOut_flg_Inproc/1  "VAPM_AVMparkingexcuteTimeOut_flg"
  VAPM_AVMparkingexcuteTimeOut_flg_Inproc/1 -> UnitConverter152/1
  UnitConverter152/1 -> VOUTP_AVMparkingexcuteTimeOut_flg/1  "VOUTP_AVMparkingexcuteTimeOut_flg"
  VAPM_AVMParkingmode_enum/1 -> VAPM_AVMParkingmode_enum_Inproc/1  "VAPM_AVMParkingmode_enum"
  VAPM_AVMParkingmode_enum_Inproc/1 -> UnitConverter153/1
  UnitConverter153/1 -> VOUTP_AVMParkingmode_enum/1  "VOUTP_AVMParkingmode_enum"
  VAPM_AVMParkingmodeTimeOut_flg/1 -> VAPM_AVMParkingmodeTimeOut_flg_Inproc/1  "VAPM_AVMParkingmodeTimeOut_flg"
  VAPM_AVMParkingmodeTimeOut_flg_Inproc/1 -> UnitConverter154/1
  UnitConverter154/1 -> VOUTP_AVMParkingmodeTimeOut_flg/1  "VOUTP_AVMParkingmodeTimeOut_flg"
  VAPM_AVMErrSTA_flg/1 -> VAPM_AVMErrSTA_flg_Inproc/1  "VAPM_AVMErrSTA_flg"
  VAPM_AVMErrSTA_flg_Inproc/1 -> UnitConverter155/1
  UnitConverter155/1 -> VOUTP_AVMErrSTA_flg/1  "VOUTP_AVMErrSTA_flg"
  VAPM_AVMErrSTATimeOut_flg/1 -> VAPM_AVMErrSTATimeOut_flg_Inproc/1  "VAPM_AVMErrSTATimeOut_flg"
  VAPM_AVMErrSTATimeOut_flg_Inproc/1 -> UnitConverter156/1
  UnitConverter156/1 -> VOUTP_AVMErrSTATimeOut_flg/1  "VOUTP_AVMErrSTATimeOut_flg"
  VAPM_IVIStatus_flg/1 -> VAPM_IVIStatus_flg_Inproc/1  "VAPM_IVIStatus_flg"
  VAPM_IVIStatus_flg_Inproc/1 -> UnitConverter157/1
  UnitConverter157/1 -> VOUTP_IVIStatus_flg/1  "VOUTP_IVIStatus_flg"
  VAPM_IVIStatusTimeOut_flg/1 -> VAPM_IVIStatusTimeOut_flg_Inproc/1  "VAPM_IVIStatusTimeOut_flg"
  VAPM_IVIStatusTimeOut_flg_Inproc/1 -> UnitConverter158/1
  UnitConverter158/1 -> VOUTP_IVIStatusTimeOut_flg/1  "VOUTP_IVIStatusTimeOut_flg"
  VAPM_CAASSw_enum/1 -> VAPM_CAASSw_enum_Inproc/1  "VAPM_CAASSw_enum"
  VAPM_CAASSw_enum_Inproc/1 -> UnitConverter159/1
  UnitConverter159/1 -> VOUTP_CAASSw_enum/1  "VOUTP_CAASSw_enum"
  VAPM_CAASSwTimeOut_flg/1 -> VAPM_CAASSwTimeOut_flg_Inproc/1  "VAPM_CAASSwTimeOut_flg"
  VAPM_CAASSwTimeOut_flg_Inproc/1 -> UnitConverter160/1
  UnitConverter160/1 -> VOUTP_CAASSwTimeOut_flg/1  "VOUTP_CAASSwTimeOut_flg"
  VAPM_IVIScreen_enum/1 -> VAPM_IVIScreen_enum_Inproc/1  "VAPM_IVIScreen_enum"
  VAPM_IVIScreen_enum_Inproc/1 -> UnitConverter161/1
  UnitConverter161/1 -> VOUTP_IVIScreen_enum/1  "VOUTP_IVIScreen_enum"
  VAPM_IVIScreenTimeOut_flg/1 -> VAPM_IVIScreenTimeOut_flg_Inproc/1  "VAPM_IVIScreenTimeOut_flg"
  VAPM_IVIScreenTimeOut_flg_Inproc/1 -> UnitConverter162/1
  UnitConverter162/1 -> VOUTP_IVIScreenTimeOut_flg/1  "VOUTP_IVIScreenTimeOut_flg"
  VAPM_ABSActive_flg/1 -> VAPM_ABSActive_flg_Inproc/1  "VAPM_ABSActive_flg"
  VAPM_ABSActive_flg_Inproc/1 -> UnitConverter163/1
  UnitConverter163/1 -> VOUTP_ABSActive_flg/1  "VOUTP_ABSActive_flg"
  VAPM_ABSActiveTimeOut_flg/1 -> VAPM_ABSActiveTimeOut_flg_Inproc/1  "VAPM_ABSActiveTimeOut_flg"
  VAPM_ABSActiveTimeOut_flg_Inproc/1 -> UnitConverter164/1
  UnitConverter164/1 -> VOUTP_ABSActiveTimeOut_flg/1  "VOUTP_ABSActiveTimeOut_flg"
  VAPM_TCSActive_flg/1 -> VAPM_TCSActive_flg_Inproc/1  "VAPM_TCSActive_flg"
  VAPM_TCSActive_flg_Inproc/1 -> UnitConverter165/1
  UnitConverter165/1 -> VOUTP_TCSActive_flg/1  "VOUTP_TCSActive_flg"
  VAPM_TCSActiveTimeOut_flg/1 -> VAPM_TCSActiveTimeOut_flg_Inproc/1  "VAPM_TCSActiveTimeOut_flg"
  VAPM_TCSActiveTimeOut_flg_Inproc/1 -> UnitConverter166/1
  UnitConverter166/1 -> VOUTP_TCSActiveTimeOut_flg/1  "VOUTP_TCSActiveTimeOut_flg"
  VAPM_DriverSeatBeltCmd_flg/1 -> VAPM_DriverSeatBeltCmd_flg_Inproc/1  "VAPM_DriverSeatBeltCmd_flg"
  VAPM_DriverSeatBeltCmd_flg_Inproc/1 -> UnitConverter167/1
  UnitConverter167/1 -> VOUTP_DriverSeatBeltCmd_flg/1  "VOUTP_DriverSeatBeltCmd_flg"
  VAPM_DriverSeatBeltCmdTimeOut_flg/1 -> VAPM_DriverSeatBeltCmdTimeOut_flg_Inproc/1  "VAPM_DriverSeatBeltCmdTimeOut_flg"
  VAPM_DriverSeatBeltCmdTimeOut_flg_Inproc/1 -> UnitConverter168/1
  UnitConverter168/1 -> VOUTP_DriverSeatBeltCmdTimeOut_flg/1  "VOUTP_DriverSeatBeltCmdTimeOut_flg"
  VAPM_APSProgressPCT_pct/1 -> VAPM_APSProgressPCT_pct_Inproc/1  "VAPM_APSProgressPCT_pct"
  VAPM_APSProgressPCT_pct_Inproc/1 -> UnitConverter169/1
  UnitConverter169/1 -> VOUTP_APSProgressPCT_pct/1  "VOUTP_APSProgressPCT_pct"
  VAPM_APSRQDisplay_enum/1 -> VAPM_APSRQDisplay_enum_Inproc/1  "VAPM_APSRQDisplay_enum"
  VAPM_APSRQDisplay_enum_Inproc/1 -> UnitConverter170/1
  UnitConverter170/1 -> VOUTP_APSRQDisplay_enum/1  "VOUTP_APSRQDisplay_enum"
  VAPM_APSSWVer_enum/1 -> VAPM_APSSWVer_enum_Inproc/1  "VAPM_APSSWVer_enum"
  VAPM_APSSWVer_enum_Inproc/1 -> UnitConverter171/1
  UnitConverter171/1 -> VOUTP_APSSWVer_enum/1  "VOUTP_APSSWVer_enum"
  VAPM_APSHWVer_enum/1 -> VAPM_APSHWVer_enum_Inproc/1  "VAPM_APSHWVer_enum"
  VAPM_APSHWVer_enum_Inproc/1 -> UnitConverter172/1
  UnitConverter172/1 -> VOUTP_APSHWVer_enum/1  "VOUTP_APSHWVer_enum"
  VAPM_APSExitCondition_enum/1 -> VAPM_APSExitCondition_enum_Inproc/1  "VAPM_APSExitCondition_enum"
  VAPM_APSExitCondition_enum_Inproc/1 -> UnitConverter173/1
  UnitConverter173/1 -> VOUTP_APSExitCondition_enum/1  "VOUTP_APSExitCondition_enum"
  VAPM_APSAngleTarget_Deg/1 -> VAPM_APSAngleTarget_Deg_Inproc/1  "VAPM_APSAngleTarget_Deg"
  VAPM_APSAngleTarget_Deg_Inproc/1 -> UnitConverter174/1
  UnitConverter174/1 -> VOUTP_APSAngleTarget_Deg/1  "VOUTP_APSAngleTarget_Deg"
  VAPM_APSVRqEPASCtrl_flg/1 -> VAPM_APSVRqEPASCtrl_flg_Inproc/1  "VAPM_APSVRqEPASCtrl_flg"
  VAPM_APSVRqEPASCtrl_flg_Inproc/1 -> UnitConverter175/1
  UnitConverter175/1 -> VOUTP_APSVRqEPASCtrl_flg/1  "VOUTP_APSVRqEPASCtrl_flg"
  VAPM_APSRqEPASCtrl_flg/1 -> VAPM_APSRqEPASCtrl_flg_Inproc/1  "VAPM_APSRqEPASCtrl_flg"
  VAPM_APSRqEPASCtrl_flg_Inproc/1 -> UnitConverter176/1
  UnitConverter176/1 -> VOUTP_APSRqEPASCtrl_flg/1  "VOUTP_APSRqEPASCtrl_flg"
  VAPM_CAASSta_enum/1 -> VAPM_CAASSta_enum_Inproc/1  "VAPM_CAASSta_enum"
  VAPM_CAASSta_enum_Inproc/1 -> UnitConverter177/1
  UnitConverter177/1 -> VOUTP_CAASSta_enum/1  "VOUTP_CAASSta_enum"
  VAPM_DKCPDkeyAreaRAPSSta_enum/1 -> VAPM_DKCPDkeyAreaRAPSSta_enum_Inproc/1  "VAPM_DKCPDkeyAreaRAPSSta_enum"
  VAPM_DKCPDkeyAreaRAPSSta_enum_Inproc/1 -> UnitConverter178/1
  UnitConverter178/1 -> VOUTP_DKCPDkeyAreaRAPSSta_enum/1  "VOUTP_DKCPDkeyAreaRAPSSta_enum"
  VAPM_DKCParkingModeCmd_enum/1 -> VAPM_DKCParkingModeCmd_enum_Inproc/1  "VAPM_DKCParkingModeCmd_enum"
  VAPM_DKCParkingModeCmd_enum_Inproc/1 -> UnitConverter179/1
  UnitConverter179/1 -> VOUTP_DKCParkingModeCmd_enum/1  "VOUTP_DKCParkingModeCmd_enum"
  VAPM_PUIDLowPower_flg/1 -> VAPM_PUIDLowPower_flg_Inproc/1  "VAPM_PUIDLowPower_flg"
  VAPM_PUIDLowPower_flg_Inproc/1 -> UnitConverter180/1
  UnitConverter180/1 -> VOUTP_PUIDLowPower_flg/1  "VOUTP_PUIDLowPower_flg"
  VAPM_CAASVMCReqA_flg/1 -> VAPM_CAASVMCReqA_flg_Inproc/1  "VAPM_CAASVMCReqA_flg"
  VAPM_CAASVMCReqA_flg_Inproc/1 -> UnitConverter181/1
  UnitConverter181/1 -> VOUTP_CAASVMCReqA_flg/1  "VOUTP_CAASVMCReqA_flg"
  VAPM_APSShiftPosnReq_enum/1 -> VAPM_APSShiftPosnReq_enum_Inproc/1  "VAPM_APSShiftPosnReq_enum"
  VAPM_APSShiftPosnReq_enum_Inproc/1 -> UnitConverter182/1
  UnitConverter182/1 -> VOUTP_APSShiftPosnReq_enum/1  "VOUTP_APSShiftPosnReq_enum"
  VAPM_APSSpeedCMD_kph/1 -> VAPM_APSSpeedCMD_kph_Inproc/1  "VAPM_APSSpeedCMD_kph"
  VAPM_APSSpeedCMD_kph_Inproc/1 -> UnitConverter183/1
  UnitConverter183/1 -> VOUTP_APSSpeedCMD_kph/1  "VOUTP_APSSpeedCMD_kph"
  VAPM_APSVMCReqA_flg/1 -> VAPM_APSVMCReqA_flg_Inproc/1  "VAPM_APSVMCReqA_flg"
  VAPM_APSVMCReqA_flg_Inproc/1 -> UnitConverter184/1
  UnitConverter184/1 -> VOUTP_APSVMCReqA_flg/1  "VOUTP_APSVMCReqA_flg"
  VAPM_RAPSBCMLamp_enum/1 -> VAPM_RAPSBCMLamp_enum_Inproc/1  "VAPM_RAPSBCMLamp_enum"
  VAPM_RAPSBCMLamp_enum_Inproc/1 -> UnitConverter185/1
  UnitConverter185/1 -> VOUTP_RAPSBCMLamp_enum/1  "VOUTP_RAPSBCMLamp_enum"
  VAPM_RAPSBCMLockReq_flg/1 -> VAPM_RAPSBCMLockReq_flg_Inproc/1  "VAPM_RAPSBCMLockReq_flg"
  VAPM_RAPSBCMLockReq_flg_Inproc/1 -> UnitConverter186/1
  UnitConverter186/1 -> VOUTP_RAPSBCMLockReq_flg/1  "VOUTP_RAPSBCMLockReq_flg"
  VAPM_APSPwrReq_enum/1 -> VAPM_APSPwrReq_enum_Inproc/1  "VAPM_APSPwrReq_enum"
  VAPM_APSPwrReq_enum_Inproc/1 -> UnitConverter187/1
  UnitConverter187/1 -> VOUTP_APSPwrReq_enum/1  "VOUTP_APSPwrReq_enum"
  VAPM_RAPSErrWarnSta_enum/1 -> VAPM_RAPSErrWarnSta_enum_Inproc/1  "VAPM_RAPSErrWarnSta_enum"
  VAPM_RAPSErrWarnSta_enum_Inproc/1 -> UnitConverter188/1
  UnitConverter188/1 -> VOUTP_RAPSErrWarnSta_enum/1  "VOUTP_RAPSErrWarnSta_enum"
  VAPM_RAPSErrLv1_flg/1 -> VAPM_RAPSErrLv1_flg_Inproc/1  "VAPM_RAPSErrLv1_flg"
  VAPM_RAPSErrLv1_flg_Inproc/1 -> UnitConverter189/1
  UnitConverter189/1 -> VOUTP_RAPSErrLv1_flg/1  "VOUTP_RAPSErrLv1_flg"
  VAPM_IVIUserTakeOverAPSSta_flg/1 -> VAPM_IVIUserTakeOverAPSSta_flg_Inproc/1  "VAPM_IVIUserTakeOverAPSSta_flg"
  VAPM_IVIUserTakeOverAPSSta_flg_Inproc/1 -> UnitConverter190/1
  UnitConverter190/1 -> VOUTP_IVIUserTakeOverAPSSta_flg/1  "VOUTP_IVIUserTakeOverAPSSta_flg"
  VBCM_FDCBCMLBeamCmd_flg/1 -> VBCM_FDCBCMLBeamCmd_flg_Inproc/1  "VBCM_FDCBCMLBeamCmd_flg"
  VBCM_FDCBCMLBeamCmd_flg_Inproc/1 -> UnitConverter191/1
  UnitConverter191/1 -> VOUTP_FDCBCMLBeamCmd_flg/1  "VOUTP_FDCBCMLBeamCmd_flg"
  VBCM_FDCBCMPLampCmd_flg/1 -> VBCM_FDCBCMPLampCmd_flg_Inproc/1  "VBCM_FDCBCMPLampCmd_flg"
  VBCM_FDCBCMPLampCmd_flg_Inproc/1 -> UnitConverter192/1
  UnitConverter192/1 -> VOUTP_FDCBCMPLampCmd_flg/1  "VOUTP_FDCBCMPLampCmd_flg"
  VBCM_FDCBCMHBeamCmd_flg/1 -> VBCM_FDCBCMHBeamCmd_flg_Inproc/1  "VBCM_FDCBCMHBeamCmd_flg"
  VBCM_FDCBCMHBeamCmd_flg_Inproc/1 -> UnitConverter193/1
  UnitConverter193/1 -> VOUTP_FDCBCMHBeamCmd_flg/1  "VOUTP_FDCBCMHBeamCmd_flg"
  VBCM_FDCBCMSMKLCmd_flg/1 -> VBCM_FDCBCMSMKLCmd_flg_Inproc/1  "VBCM_FDCBCMSMKLCmd_flg"
  VBCM_FDCBCMSMKLCmd_flg_Inproc/1 -> UnitConverter194/1
  UnitConverter194/1 -> VOUTP_FDCBCMSMKLCmd_flg/1  "VOUTP_FDCBCMSMKLCmd_flg"
  VBCM_FDCBCMSMKRCmd_flg/1 -> VBCM_FDCBCMSMKRCmd_flg_Inproc/1  "VBCM_FDCBCMSMKRCmd_flg"
  VBCM_FDCBCMSMKRCmd_flg_Inproc/1 -> UnitConverter195/1
  UnitConverter195/1 -> VOUTP_FDCBCMSMKRCmd_flg/1  "VOUTP_FDCBCMSMKRCmd_flg"
  VBCM_FDCBCMDVRSignalLCmd_flg/1 -> VBCM_FDCBCMDVRSignalLCmd_flg_Inproc/1  "VBCM_FDCBCMDVRSignalLCmd_flg"
  VBCM_FDCBCMDVRSignalLCmd_flg_Inproc/1 -> UnitConverter196/1
  UnitConverter196/1 -> VOUTP_FDCBCMDVRSignalLCmd_flg/1  "VOUTP_FDCBCMDVRSignalLCmd_flg"
  VBCM_FDCBCMDVRSignalRCmd_flg/1 -> VBCM_FDCBCMDVRSignalRCmd_flg_Inproc/1  "VBCM_FDCBCMDVRSignalRCmd_flg"
  VBCM_FDCBCMDVRSignalRCmd_flg_Inproc/1 -> UnitConverter197/1
  UnitConverter197/1 -> VOUTP_FDCBCMDVRSignalRCmd_flg/1  "VOUTP_FDCBCMDVRSignalRCmd_flg"
  VBCM_FDCBCMBSDBuzzerCmd_flg/1 -> VBCM_FDCBCMBSDBuzzerCmd_flg_Inproc/1  "VBCM_FDCBCMBSDBuzzerCmd_flg"
  VBCM_FDCBCMBSDBuzzerCmd_flg_Inproc/1 -> UnitConverter198/1
  UnitConverter198/1 -> VOUTP_FDCBCMBSDBuzzerCmd_flg/1  "VOUTP_FDCBCMBSDBuzzerCmd_flg"
  VBCM_FDCBCMSLTLpCmd_flg/1 -> VBCM_FDCBCMSLTLpCmd_flg_Inproc/1  "VBCM_FDCBCMSLTLpCmd_flg"
  VBCM_FDCBCMSLTLpCmd_flg_Inproc/1 -> UnitConverter199/1
  UnitConverter199/1 -> VOUTP_FDCBCMSLTLpCmd_flg/1  "VOUTP_FDCBCMSLTLpCmd_flg"
  VBCM_FDCBCMSRTLpCmd_flg/1 -> VBCM_FDCBCMSRTLpCmd_flg_Inproc/1  "VBCM_FDCBCMSRTLpCmd_flg"
  VBCM_FDCBCMSRTLpCmd_flg_Inproc/1 -> UnitConverter200/1
  UnitConverter200/1 -> VOUTP_FDCBCMSRTLpCmd_flg/1  "VOUTP_FDCBCMSRTLpCmd_flg"
  VBCM_FDCBCMLTurnLpCmd_flg/1 -> VBCM_FDCBCMLTurnLpCmd_flg_Inproc/1  "VBCM_FDCBCMLTurnLpCmd_flg"
  VBCM_FDCBCMLTurnLpCmd_flg_Inproc/1 -> UnitConverter201/1
  UnitConverter201/1 -> VOUTP_FDCBCMLTurnLpCmd_flg/1  "VOUTP_FDCBCMLTurnLpCmd_flg"
  VBCM_FDCBCMRTurnLpCmd_flg/1 -> VBCM_FDCBCMRTurnLpCmd_flg_Inproc/1  "VBCM_FDCBCMRTurnLpCmd_flg"
  VBCM_FDCBCMRTurnLpCmd_flg_Inproc/1 -> UnitConverter202/1
  UnitConverter202/1 -> VOUTP_FDCBCMRTurnLpCmd_flg/1  "VOUTP_FDCBCMRTurnLpCmd_flg"
  VBCM_FDCBCMStopINDCmd_flg/1 -> VBCM_FDCBCMStopINDCmd_flg_Inproc/1  "VBCM_FDCBCMStopINDCmd_flg"
  VBCM_FDCBCMStopINDCmd_flg_Inproc/1 -> UnitConverter203/1
  UnitConverter203/1 -> VOUTP_FDCBCMStopINDCmd_flg/1  "VOUTP_FDCBCMStopINDCmd_flg"
  VBCM_FDCBCMSTOPBALLCmd_flg/1 -> VBCM_FDCBCMSTOPBALLCmd_flg_Inproc/1  "VBCM_FDCBCMSTOPBALLCmd_flg"
  VBCM_FDCBCMSTOPBALLCmd_flg_Inproc/1 -> UnitConverter204/1
  UnitConverter204/1 -> VOUTP_FDCBCMSTOPBALLCmd_flg/1  "VOUTP_FDCBCMSTOPBALLCmd_flg"
  VBCM_FDCBCMInnerCallBellCmd_flg/1 -> VBCM_FDCBCMInnerCallBellCmd_flg_Inproc/1  "VBCM_FDCBCMInnerCallBellCmd_flg"
  VBCM_FDCBCMInnerCallBellCmd_flg_Inproc/1 -> UnitConverter205/1
  UnitConverter205/1 -> VOUTP_FDCBCMInnerCallBellCmd_flg/1  "VOUTP_FDCBCMInnerCallBellCmd_flg"
  VBCM_FDCBCMCallBellCmd_flg/1 -> VBCM_FDCBCMCallBellCmd_flg_Inproc/1  "VBCM_FDCBCMCallBellCmd_flg"
  VBCM_FDCBCMCallBellCmd_flg_Inproc/1 -> UnitConverter206/1
  UnitConverter206/1 -> VOUTP_FDCBCMCallBellCmd_flg/1  "VOUTP_FDCBCMCallBellCmd_flg"
  VBCM_FDCBCMWiperHCmd_flg/1 -> VBCM_FDCBCMWiperHCmd_flg_Inproc/1  "VBCM_FDCBCMWiperHCmd_flg"
  VBCM_FDCBCMWiperHCmd_flg_Inproc/1 -> UnitConverter207/1
  UnitConverter207/1 -> VOUTP_FDCBCMWiperHCmd_flg/1  "VOUTP_FDCBCMWiperHCmd_flg"
  VBCM_FDCBCMWasherCmd_flg/1 -> VBCM_FDCBCMWasherCmd_flg_Inproc/1  "VBCM_FDCBCMWasherCmd_flg"
  VBCM_FDCBCMWasherCmd_flg_Inproc/1 -> UnitConverter208/1
  UnitConverter208/1 -> VOUTP_FDCBCMWasherCmd_flg/1  "VOUTP_FDCBCMWasherCmd_flg"
  VBCM_FDCBCMWiperLCmd_flg/1 -> VBCM_FDCBCMWiperLCmd_flg_Inproc/1  "VBCM_FDCBCMWiperLCmd_flg"
  VBCM_FDCBCMWiperLCmd_flg_Inproc/1 -> UnitConverter209/1
  UnitConverter209/1 -> VOUTP_FDCBCMWiperLCmd_flg/1  "VOUTP_FDCBCMWiperLCmd_flg"
  VBCM_FDCBCMLDRLCmd_flg/1 -> VBCM_FDCBCMLDRLCmd_flg_Inproc/1  "VBCM_FDCBCMLDRLCmd_flg"
  VBCM_FDCBCMLDRLCmd_flg_Inproc/1 -> UnitConverter210/1
  UnitConverter210/1 -> VOUTP_FDCBCMLDRLCmd_flg/1  "VOUTP_FDCBCMLDRLCmd_flg"
  VBCM_FDCBCMRDRLCmd_flg/1 -> VBCM_FDCBCMRDRLCmd_flg_Inproc/1  "VBCM_FDCBCMRDRLCmd_flg"
  VBCM_FDCBCMRDRLCmd_flg_Inproc/1 -> UnitConverter211/1
  UnitConverter211/1 -> VOUTP_FDCBCMRDRLCmd_flg/1  "VOUTP_FDCBCMRDRLCmd_flg"
  VBCM_FDCBCMRFLampCmd_flg/1 -> VBCM_FDCBCMRFLampCmd_flg_Inproc/1  "VBCM_FDCBCMRFLampCmd_flg"
  VBCM_FDCBCMRFLampCmd_flg_Inproc/1 -> UnitConverter212/1
  UnitConverter212/1 -> VOUTP_FDCBCMRFLampCmd_flg/1  "VOUTP_FDCBCMRFLampCmd_flg"
  VBCM_TurnLpPatternSta_enum/1 -> VBCM_TurnLpPatternSta_enum_Inproc/1  "VBCM_TurnLpPatternSta_enum"
  VBCM_TurnLpPatternSta_enum_Inproc/1 -> UnitConverter213/1
  UnitConverter213/1 -> VOUTP_TurnLpPatternSta_enum/1  "VOUTP_TurnLpPatternSta_enum"
  VBCM_FDCBCMFDoorSta_flg/1 -> VBCM_FDCBCMFDoorSta_flg_Inproc/1  "VBCM_FDCBCMFDoorSta_flg"
  VBCM_FDCBCMFDoorSta_flg_Inproc/1 -> UnitConverter214/1
  UnitConverter214/1 -> VOUTP_FDCBCMFDoorSta_flg/1  "VOUTP_FDCBCMFDoorSta_flg"
  VBCM_FDCBCMMDoorSta_flg/1 -> VBCM_FDCBCMMDoorSta_flg_Inproc/1  "VBCM_FDCBCMMDoorSta_flg"
  VBCM_FDCBCMMDoorSta_flg_Inproc/1 -> UnitConverter215/1
  UnitConverter215/1 -> VOUTP_FDCBCMMDoorSta_flg/1  "VOUTP_FDCBCMMDoorSta_flg"
  VBCM_FDCBCMRDoorSta_flg/1 -> VBCM_FDCBCMRDoorSta_flg_Inproc/1  "VBCM_FDCBCMRDoorSta_flg"
  VBCM_FDCBCMRDoorSta_flg_Inproc/1 -> UnitConverter216/1
  UnitConverter216/1 -> VOUTP_FDCBCMRDoorSta_flg/1  "VOUTP_FDCBCMRDoorSta_flg"
  VBCM_FDCBCMRoomLpAmbCmd_flg/1 -> VBCM_FDCBCMRoomLpAmbCmd_flg_Inproc/1  "VBCM_FDCBCMRoomLpAmbCmd_flg"
  VBCM_FDCBCMRoomLpAmbCmd_flg_Inproc/1 -> UnitConverter217/1
  UnitConverter217/1 -> VOUTP_FDCBCMRoomLpAmbCmd_flg/1  "VOUTP_FDCBCMRoomLpAmbCmd_flg"
  VBCM_FDCBCMLBSDRCmd_flg/1 -> VBCM_FDCBCMLBSDRCmd_flg_Inproc/1  "VBCM_FDCBCMLBSDRCmd_flg"
  VBCM_FDCBCMLBSDRCmd_flg_Inproc/1 -> UnitConverter218/1
  UnitConverter218/1 -> VOUTP_FDCBCMLBSDRCmd_flg/1  "VOUTP_FDCBCMLBSDRCmd_flg"
  VBCM_FDCBCMLBSDYCmd_flg/1 -> VBCM_FDCBCMLBSDYCmd_flg_Inproc/1  "VBCM_FDCBCMLBSDYCmd_flg"
  VBCM_FDCBCMLBSDYCmd_flg_Inproc/1 -> UnitConverter219/1
  UnitConverter219/1 -> VOUTP_FDCBCMLBSDYCmd_flg/1  "VOUTP_FDCBCMLBSDYCmd_flg"
  VBCM_FDCBCMRBSDRCmd_flg/1 -> VBCM_FDCBCMRBSDRCmd_flg_Inproc/1  "VBCM_FDCBCMRBSDRCmd_flg"
  VBCM_FDCBCMRBSDRCmd_flg_Inproc/1 -> UnitConverter220/1
  UnitConverter220/1 -> VOUTP_FDCBCMRBSDRCmd_flg/1  "VOUTP_FDCBCMRBSDRCmd_flg"
  VBCM_FDCBCMRBSDYCmd_flg/1 -> VBCM_FDCBCMRBSDYCmd_flg_Inproc/1  "VBCM_FDCBCMRBSDYCmd_flg"
  VBCM_FDCBCMRBSDYCmd_flg_Inproc/1 -> UnitConverter221/1
  UnitConverter221/1 -> VOUTP_FDCBCMRBSDYCmd_flg/1  "VOUTP_FDCBCMRBSDYCmd_flg"
  VBCM_FDCBCMEmExitSWSta_flg/1 -> VBCM_FDCBCMEmExitSWSta_flg_Inproc/1  "VBCM_FDCBCMEmExitSWSta_flg"
  VBCM_FDCBCMEmExitSWSta_flg_Inproc/1 -> UnitConverter222/1
  UnitConverter222/1 -> VOUTP_FDCBCMEmExitSWSta_flg/1  "VOUTP_FDCBCMEmExitSWSta_flg"
  VBCM_InnerBuzzerModeSta_enum/1 -> VBCM_InnerBuzzerModeSta_enum_Inproc/1  "VBCM_InnerBuzzerModeSta_enum"
  VBCM_InnerBuzzerModeSta_enum_Inproc/1 -> UnitConverter223/1
  UnitConverter223/1 -> VOUTP_InnerBuzzerModeSta_enum/1  "VOUTP_InnerBuzzerModeSta_enum"
  VBCM_FDCBCMInnerBuzzerCmd_flg/1 -> VBCM_FDCBCMInnerBuzzerCmd_flg_Inproc/1  "VBCM_FDCBCMInnerBuzzerCmd_flg"
  VBCM_FDCBCMInnerBuzzerCmd_flg_Inproc/1 -> UnitConverter224/1
  UnitConverter224/1 -> VOUTP_FDCBCMInnerBuzzerCmd_flg/1  "VOUTP_FDCBCMInnerBuzzerCmd_flg"
  VBCM_FDCBCMRoomLpAmbSetSta_flg/1 -> VBCM_FDCBCMRoomLpAmbSetSta_flg_Inproc/1  "VBCM_FDCBCMRoomLpAmbSetSta_flg"
  VBCM_FDCBCMRoomLpAmbSetSta_flg_Inproc/1 -> UnitConverter225/1
  UnitConverter225/1 -> VOUTP_FDCBCMRoomLpAmbSetSta_flg/1  "VOUTP_FDCBCMRoomLpAmbSetSta_flg"
  VBCM_FDCBCMRoomLpSetSta_flg/1 -> VBCM_FDCBCMRoomLpSetSta_flg_Inproc/1  "VBCM_FDCBCMRoomLpSetSta_flg"
  VBCM_FDCBCMRoomLpSetSta_flg_Inproc/1 -> UnitConverter226/1
  UnitConverter226/1 -> VOUTP_FDCBCMRoomLpSetSta_flg/1  "VOUTP_FDCBCMRoomLpSetSta_flg"
  VBCM_FDCBCMFRoomLpSetSta_pct/1 -> VBCM_FDCBCMFRoomLpSetSta_pct_Inproc/1  "VBCM_FDCBCMFRoomLpSetSta_pct"
  VBCM_FDCBCMFRoomLpSetSta_pct_Inproc/1 -> UnitConverter227/1
  UnitConverter227/1 -> VOUTP_FDCBCMFRoomLpSetSta_pct/1  "VOUTP_FDCBCMFRoomLpSetSta_pct"
  VBCM_FDCBCMFRoomLpCmd_pct/1 -> VBCM_FDCBCMFRoomLpCmd_pct_Inproc/1  "VBCM_FDCBCMFRoomLpCmd_pct"
  VBCM_FDCBCMFRoomLpCmd_pct_Inproc/1 -> UnitConverter228/1
  UnitConverter228/1 -> VOUTP_FDCBCMFRoomLpCmd_pct/1  "VOUTP_FDCBCMFRoomLpCmd_pct"
  VBCM_FDCBCMMRoomLpSetSta_pct/1 -> VBCM_FDCBCMMRoomLpSetSta_pct_Inproc/1  "VBCM_FDCBCMMRoomLpSetSta_pct"
  VBCM_FDCBCMMRoomLpSetSta_pct_Inproc/1 -> UnitConverter229/1
  UnitConverter229/1 -> VOUTP_FDCBCMMRoomLpSetSta_pct/1  "VOUTP_FDCBCMMRoomLpSetSta_pct"
  VBCM_FDCBCMMRoomLpCmd_pct/1 -> VBCM_FDCBCMMRoomLpCmd_pct_Inproc/1  "VBCM_FDCBCMMRoomLpCmd_pct"
  VBCM_FDCBCMMRoomLpCmd_pct_Inproc/1 -> UnitConverter230/1
  UnitConverter230/1 -> VOUTP_FDCBCMMRoomLpCmd_pct/1  "VOUTP_FDCBCMMRoomLpCmd_pct"
  VBCM_FDCBCMRRoomLpSetSta_pct/1 -> VBCM_FDCBCMRRoomLpSetSta_pct_Inproc/1  "VBCM_FDCBCMRRoomLpSetSta_pct"
  VBCM_FDCBCMRRoomLpSetSta_pct_Inproc/1 -> UnitConverter231/1
  UnitConverter231/1 -> VOUTP_FDCBCMRRoomLpSetSta_pct/1  "VOUTP_FDCBCMRRoomLpSetSta_pct"
  VBCM_FDCBCMRRoomLpCmd_pct/1 -> VBCM_FDCBCMRRoomLpCmd_pct_Inproc/1  "VBCM_FDCBCMRRoomLpCmd_pct"
  VBCM_FDCBCMRRoomLpCmd_pct_Inproc/1 -> UnitConverter232/1
  UnitConverter232/1 -> VOUTP_FDCBCMRRoomLpCmd_pct/1  "VOUTP_FDCBCMRRoomLpCmd_pct"
  VBCM_FDCBCMHelpINDCmd_flg/1 -> VBCM_FDCBCMHelpINDCmd_flg_Inproc/1  "VBCM_FDCBCMHelpINDCmd_flg"
  VBCM_FDCBCMHelpINDCmd_flg_Inproc/1 -> UnitConverter233/1
  UnitConverter233/1 -> VOUTP_FDCBCMHelpINDCmd_flg/1  "VOUTP_FDCBCMHelpINDCmd_flg"
  VBCM_FDCBCMOSDrOpenSWSta_enum/1 -> VBCM_FDCBCMOSDrOpenSWSta_enum_Inproc/1  "VBCM_FDCBCMOSDrOpenSWSta_enum"
  VBCM_FDCBCMOSDrOpenSWSta_enum_Inproc/1 -> UnitConverter234/1
  UnitConverter234/1 -> VOUTP_FDCBCMOSDrOpenSWSta_enum/1  "VOUTP_FDCBCMOSDrOpenSWSta_enum"
  VBCM_FDCBCMEmSVCmd_flg/1 -> VBCM_FDCBCMEmSVCmd_flg_Inproc/1  "VBCM_FDCBCMEmSVCmd_flg"
  VBCM_FDCBCMEmSVCmd_flg_Inproc/1 -> UnitConverter235/1
  UnitConverter235/1 -> VOUTP_FDCBCMEmSVCmd_flg/1  "VOUTP_FDCBCMEmSVCmd_flg"
  VBCM_FDCBCMFDOpenSVCmd_flg/1 -> VBCM_FDCBCMFDOpenSVCmd_flg_Inproc/1  "VBCM_FDCBCMFDOpenSVCmd_flg"
  VBCM_FDCBCMFDOpenSVCmd_flg_Inproc/1 -> UnitConverter236/1
  UnitConverter236/1 -> VOUTP_FDCBCMFDOpenSVCmd_flg/1  "VOUTP_FDCBCMFDOpenSVCmd_flg"
  VBCM_FDCBCMFDCloseSVCmd_flg/1 -> VBCM_FDCBCMFDCloseSVCmd_flg_Inproc/1  "VBCM_FDCBCMFDCloseSVCmd_flg"
  VBCM_FDCBCMFDCloseSVCmd_flg_Inproc/1 -> UnitConverter237/1
  UnitConverter237/1 -> VOUTP_FDCBCMFDCloseSVCmd_flg/1  "VOUTP_FDCBCMFDCloseSVCmd_flg"
  VBCM_FDCBCMMDOpenSVCmd_flg/1 -> VBCM_FDCBCMMDOpenSVCmd_flg_Inproc/1  "VBCM_FDCBCMMDOpenSVCmd_flg"
  VBCM_FDCBCMMDOpenSVCmd_flg_Inproc/1 -> UnitConverter238/1
  UnitConverter238/1 -> VOUTP_FDCBCMMDOpenSVCmd_flg/1  "VOUTP_FDCBCMMDOpenSVCmd_flg"
  VBCM_FDCBCMMDCloseSVCmd_flg/1 -> VBCM_FDCBCMMDCloseSVCmd_flg_Inproc/1  "VBCM_FDCBCMMDCloseSVCmd_flg"
  VBCM_FDCBCMMDCloseSVCmd_flg_Inproc/1 -> UnitConverter239/1
  UnitConverter239/1 -> VOUTP_FDCBCMMDCloseSVCmd_flg/1  "VOUTP_FDCBCMMDCloseSVCmd_flg"
  VBCM_FDCBCMLTurnSWSta_flg/1 -> VBCM_FDCBCMLTurnSWSta_flg_Inproc/1  "VBCM_FDCBCMLTurnSWSta_flg"
  VBCM_FDCBCMLTurnSWSta_flg_Inproc/1 -> UnitConverter240/1
  UnitConverter240/1 -> VOUTP_FDCBCMLTurnSWSta_flg/1  "VOUTP_FDCBCMLTurnSWSta_flg"
  VBCM_FDCBCMRTurnSWSta_flg/1 -> VBCM_FDCBCMRTurnSWSta_flg_Inproc/1  "VBCM_FDCBCMRTurnSWSta_flg"
  VBCM_FDCBCMRTurnSWSta_flg_Inproc/1 -> UnitConverter241/1
  UnitConverter241/1 -> VOUTP_FDCBCMRTurnSWSta_flg/1  "VOUTP_FDCBCMRTurnSWSta_flg"
  VBCM_FDCBCMRGearSta_flg/1 -> VBCM_FDCBCMRGearSta_flg_Inproc/1  "VBCM_FDCBCMRGearSta_flg"
  VBCM_FDCBCMRGearSta_flg_Inproc/1 -> UnitConverter242/1
  UnitConverter242/1 -> VOUTP_FDCBCMRGearSta_flg/1  "VOUTP_FDCBCMRGearSta_flg"
  VBCM_FDCBCMBrakeCmd_flg/1 -> VBCM_FDCBCMBrakeCmd_flg_Inproc/1  "VBCM_FDCBCMBrakeCmd_flg"
  VBCM_FDCBCMBrakeCmd_flg_Inproc/1 -> UnitConverter243/1
  UnitConverter243/1 -> VOUTP_FDCBCMBrakeCmd_flg/1  "VOUTP_FDCBCMBrakeCmd_flg"
  VBCM_FDCBCMTurnBuzzerENSta_flg/1 -> VBCM_FDCBCMTurnBuzzerENSta_flg_Inproc/1  "VBCM_FDCBCMTurnBuzzerENSta_flg"
  VBCM_FDCBCMTurnBuzzerENSta_flg_Inproc/1 -> UnitConverter244/1
  UnitConverter244/1 -> VOUTP_FDCBCMTurnBuzzerENSta_flg/1  "VOUTP_FDCBCMTurnBuzzerENSta_flg"
  VBCM_WakeUp_flg/1 -> VBCM_WakeUp_flg_Inproc/1  "VBCM_WakeUp_flg"
  VBCM_WakeUp_flg_Inproc/1 -> UnitConverter245/1
  UnitConverter245/1 -> VOUTP_WakeUp_flg/1  "VOUTP_WakeUp_flg"
  VBCM_KeepWakeUp_flg/1 -> VBCM_KeepWakeUp_flg_Inproc/1  "VBCM_KeepWakeUp_flg"
  VBCM_KeepWakeUp_flg_Inproc/1 -> UnitConverter246/1
  UnitConverter246/1 -> VOUTP_KeepWakeUp_flg/1  "VOUTP_KeepWakeUp_flg"
  VDDM_C3BMS6RCDTC_raw32/1 -> VDDM_C3BMS6RCDTC_raw32_Inproc/1  "VDDM_C3BMS6RCDTC_raw32"
  VDDM_C3BMS6RCDTC_raw32_Inproc/1 -> UnitConverter247/1
  UnitConverter247/1 -> VOUTP_C3BMS6RCDTC_raw32/1  "VOUTP_C3BMS6RCDTC_raw32"
  VDDM_C3BMS6CSDTC_raw32/1 -> VDDM_C3BMS6CSDTC_raw32_Inproc/1  "VDDM_C3BMS6CSDTC_raw32"
  VDDM_C3BMS6CSDTC_raw32_Inproc/1 -> UnitConverter248/1
  UnitConverter248/1 -> VOUTP_C3BMS6CSDTC_raw32/1  "VOUTP_C3BMS6CSDTC_raw32"
  VDDM_C3BMS6LCDTC_raw32/1 -> VDDM_C3BMS6LCDTC_raw32_Inproc/1  "VDDM_C3BMS6LCDTC_raw32"
  VDDM_C3BMS6LCDTC_raw32_Inproc/1 -> UnitConverter249/1
  UnitConverter249/1 -> VOUTP_C3BMS6LCDTC_raw32/1  "VOUTP_C3BMS6LCDTC_raw32"
  VDDM_C3BMS1RCDTC_raw32/1 -> VDDM_C3BMS1RCDTC_raw32_Inproc/1  "VDDM_C3BMS1RCDTC_raw32"
  VDDM_C3BMS1RCDTC_raw32_Inproc/1 -> UnitConverter250/1
  UnitConverter250/1 -> VOUTP_C3BMS1RCDTC_raw32/1  "VOUTP_C3BMS1RCDTC_raw32"
  VDDM_C3BMS1CSDTC_raw32/1 -> VDDM_C3BMS1CSDTC_raw32_Inproc/1  "VDDM_C3BMS1CSDTC_raw32"
  VDDM_C3BMS1CSDTC_raw32_Inproc/1 -> UnitConverter251/1
  UnitConverter251/1 -> VOUTP_C3BMS1CSDTC_raw32/1  "VOUTP_C3BMS1CSDTC_raw32"
  VDDM_C3BMS1LCDTC_raw32/1 -> VDDM_C3BMS1LCDTC_raw32_Inproc/1  "VDDM_C3BMS1LCDTC_raw32"
  VDDM_C3BMS1LCDTC_raw32_Inproc/1 -> UnitConverter252/1
  UnitConverter252/1 -> VOUTP_C3BMS1LCDTC_raw32/1  "VOUTP_C3BMS1LCDTC_raw32"
  VDDM_C3CCU1RCDTC_raw32/1 -> VDDM_C3CCU1RCDTC_raw32_Inproc/1  "VDDM_C3CCU1RCDTC_raw32"
  VDDM_C3CCU1RCDTC_raw32_Inproc/1 -> UnitConverter253/1
  UnitConverter253/1 -> VOUTP_C3CCU1RCDTC_raw32/1  "VOUTP_C3CCU1RCDTC_raw32"
  VDDM_C3CCU1CSDTC_raw32/1 -> VDDM_C3CCU1CSDTC_raw32_Inproc/1  "VDDM_C3CCU1CSDTC_raw32"
  VDDM_C3CCU1CSDTC_raw32_Inproc/1 -> UnitConverter254/1
  UnitConverter254/1 -> VOUTP_C3CCU1CSDTC_raw32/1  "VOUTP_C3CCU1CSDTC_raw32"
  VDDM_C3CCU1LCDTC_raw32/1 -> VDDM_C3CCU1LCDTC_raw32_Inproc/1  "VDDM_C3CCU1LCDTC_raw32"
  VDDM_C3CCU1LCDTC_raw32_Inproc/1 -> UnitConverter255/1
  UnitConverter255/1 -> VOUTP_C3CCU1LCDTC_raw32/1  "VOUTP_C3CCU1LCDTC_raw32"
  VDDM_C3CCU2RCDTC_raw32/1 -> VDDM_C3CCU2RCDTC_raw32_Inproc/1  "VDDM_C3CCU2RCDTC_raw32"
  VDDM_C3CCU2RCDTC_raw32_Inproc/1 -> UnitConverter256/1
  UnitConverter256/1 -> VOUTP_C3CCU2RCDTC_raw32/1  "VOUTP_C3CCU2RCDTC_raw32"
  VDDM_C3CCU2CSDTC_raw32/1 -> VDDM_C3CCU2CSDTC_raw32_Inproc/1  "VDDM_C3CCU2CSDTC_raw32"
  VDDM_C3CCU2CSDTC_raw32_Inproc/1 -> UnitConverter257/1
  UnitConverter257/1 -> VOUTP_C3CCU2CSDTC_raw32/1  "VOUTP_C3CCU2CSDTC_raw32"
  VDDM_C3CCU2LCDTC_raw32/1 -> VDDM_C3CCU2LCDTC_raw32_Inproc/1  "VDDM_C3CCU2LCDTC_raw32"
  VDDM_C3CCU2LCDTC_raw32_Inproc/1 -> UnitConverter258/1
  UnitConverter258/1 -> VOUTP_C3CCU2LCDTC_raw32/1  "VOUTP_C3CCU2LCDTC_raw32"
  VDDM_C1ABM1RCDTC_raw32/1 -> VDDM_C1ABM1RCDTC_raw32_Inproc/1  "VDDM_C1ABM1RCDTC_raw32"
  VDDM_C1ABM1RCDTC_raw32_Inproc/1 -> UnitConverter259/1
  UnitConverter259/1 -> VOUTP_C1ABM1RCDTC_raw32/1  "VOUTP_C1ABM1RCDTC_raw32"
  VDDM_C1ABM1CSDTC_raw32/1 -> VDDM_C1ABM1CSDTC_raw32_Inproc/1  "VDDM_C1ABM1CSDTC_raw32"
  VDDM_C1ABM1CSDTC_raw32_Inproc/1 -> UnitConverter260/1
  UnitConverter260/1 -> VOUTP_C1ABM1CSDTC_raw32/1  "VOUTP_C1ABM1CSDTC_raw32"
  VDDM_C1ABM1LCDTC_raw32/1 -> VDDM_C1ABM1LCDTC_raw32_Inproc/1  "VDDM_C1ABM1LCDTC_raw32"
  VDDM_C1ABM1LCDTC_raw32_Inproc/1 -> UnitConverter261/1
  UnitConverter261/1 -> VOUTP_C1ABM1LCDTC_raw32/1  "VOUTP_C1ABM1LCDTC_raw32"
  VDDM_Lv1ErrDTC_raw32/1 -> VDDM_Lv1ErrDTC_raw32_Inproc/1  "VDDM_Lv1ErrDTC_raw32"
  VDDM_Lv1ErrDTC_raw32_Inproc/1 -> UnitConverter262/1
  UnitConverter262/1 -> VOUTP_Lv1ErrDTC_raw32/1  "VOUTP_Lv1ErrDTC_raw32"
  VDDM_Lv2ErrDTC_raw32/1 -> VDDM_Lv2ErrDTC_raw32_Inproc/1  "VDDM_Lv2ErrDTC_raw32"
  VDDM_Lv2ErrDTC_raw32_Inproc/1 -> UnitConverter263/1
  UnitConverter263/1 -> VOUTP_Lv2ErrDTC_raw32/1  "VOUTP_Lv2ErrDTC_raw32"
  VDDM_Lv3ErrDTC_raw32/1 -> VDDM_Lv3ErrDTC_raw32_Inproc/1  "VDDM_Lv3ErrDTC_raw32"
  VDDM_Lv3ErrDTC_raw32_Inproc/1 -> UnitConverter264/1
  UnitConverter264/1 -> VOUTP_Lv3ErrDTC_raw32/1  "VOUTP_Lv3ErrDTC_raw32"
  VDDM_Lv4ErrDTC_raw32/1 -> VDDM_Lv4ErrDTC_raw32_Inproc/1  "VDDM_Lv4ErrDTC_raw32"
  VDDM_Lv4ErrDTC_raw32_Inproc/1 -> UnitConverter265/1
  UnitConverter265/1 -> VOUTP_Lv4ErrDTC_raw32/1  "VOUTP_Lv4ErrDTC_raw32"
  VDDM_BrkSWErrDTC_raw32/1 -> VDDM_BrkSWErrDTC_raw32_Inproc/1  "VDDM_BrkSWErrDTC_raw32"
  VDDM_BrkSWErrDTC_raw32_Inproc/1 -> UnitConverter266/1
  UnitConverter266/1 -> VOUTP_BrkSWErrDTC_raw32/1  "VOUTP_BrkSWErrDTC_raw32"
  VDDM_BrkSWNoBacDTC_raw32/1 -> VDDM_BrkSWNoBacDTC_raw32_Inproc/1  "VDDM_BrkSWNoBacDTC_raw32"
  VDDM_BrkSWNoBacDTC_raw32_Inproc/1 -> UnitConverter267/1
  UnitConverter267/1 -> VOUTP_BrkSWNoBacDTC_raw32/1  "VOUTP_BrkSWNoBacDTC_raw32"
  VDDM_KeyAuthDTC_raw32/1 -> VDDM_KeyAuthDTC_raw32_Inproc/1  "VDDM_KeyAuthDTC_raw32"
  VDDM_KeyAuthDTC_raw32_Inproc/1 -> UnitConverter268/1
  UnitConverter268/1 -> VOUTP_KeyAuthDTC_raw32/1  "VOUTP_KeyAuthDTC_raw32"
  VDDM_ONtoRdyDTC_raw32/1 -> VDDM_ONtoRdyDTC_raw32_Inproc/1  "VDDM_ONtoRdyDTC_raw32"
  VDDM_ONtoRdyDTC_raw32_Inproc/1 -> UnitConverter269/1
  UnitConverter269/1 -> VOUTP_ONtoRdyDTC_raw32/1  "VOUTP_ONtoRdyDTC_raw32"
  VDDM_HVB4PreDTC_raw32/1 -> VDDM_HVB4PreDTC_raw32_Inproc/1  "VDDM_HVB4PreDTC_raw32"
  VDDM_HVB4PreDTC_raw32_Inproc/1 -> UnitConverter270/1
  UnitConverter270/1 -> VOUTP_HVB4PreDTC_raw32/1  "VOUTP_HVB4PreDTC_raw32"
  VDDM_MCU4PreDTC_raw32/1 -> VDDM_MCU4PreDTC_raw32_Inproc/1  "VDDM_MCU4PreDTC_raw32"
  VDDM_MCU4PreDTC_raw32_Inproc/1 -> UnitConverter271/1
  UnitConverter271/1 -> VOUTP_MCU4PreDTC_raw32/1  "VOUTP_MCU4PreDTC_raw32"
  VDDM_DCDC4PreDTC_raw32/1 -> VDDM_DCDC4PreDTC_raw32_Inproc/1  "VDDM_DCDC4PreDTC_raw32"
  VDDM_DCDC4PreDTC_raw32_Inproc/1 -> UnitConverter272/1
  UnitConverter272/1 -> VOUTP_DCDC4PreDTC_raw32/1  "VOUTP_DCDC4PreDTC_raw32"
  VDDM_HVRlyCloDTC_raw32/1 -> VDDM_HVRlyCloDTC_raw32_Inproc/1  "VDDM_HVRlyCloDTC_raw32"
  VDDM_HVRlyCloDTC_raw32_Inproc/1 -> UnitConverter273/1
  UnitConverter273/1 -> VOUTP_HVRlyCloDTC_raw32/1  "VOUTP_HVRlyCloDTC_raw32"
  VDDM_BMSRdyDTC_raw32/1 -> VDDM_BMSRdyDTC_raw32_Inproc/1  "VDDM_BMSRdyDTC_raw32"
  VDDM_BMSRdyDTC_raw32_Inproc/1 -> UnitConverter274/1
  UnitConverter274/1 -> VOUTP_BMSRdyDTC_raw32/1  "VOUTP_BMSRdyDTC_raw32"
  VDDM_DCDCEnaDTC_raw32/1 -> VDDM_DCDCEnaDTC_raw32_Inproc/1  "VDDM_DCDCEnaDTC_raw32"
  VDDM_DCDCEnaDTC_raw32_Inproc/1 -> UnitConverter275/1
  UnitConverter275/1 -> VOUTP_DCDCEnaDTC_raw32/1  "VOUTP_DCDCEnaDTC_raw32"
  VDDM_HiLvSaChkDTC_raw32/1 -> VDDM_HiLvSaChkDTC_raw32_Inproc/1  "VDDM_HiLvSaChkDTC_raw32"
  VDDM_HiLvSaChkDTC_raw32_Inproc/1 -> UnitConverter276/1
  UnitConverter276/1 -> VOUTP_HiLvSaChkDTC_raw32/1  "VOUTP_HiLvSaChkDTC_raw32"
  VDDM_MidLvSaChkDTC_raw32/1 -> VDDM_MidLvSaChkDTC_raw32_Inproc/1  "VDDM_MidLvSaChkDTC_raw32"
  VDDM_MidLvSaChkDTC_raw32_Inproc/1 -> UnitConverter277/1
  UnitConverter277/1 -> VOUTP_MidLvSaChkDTC_raw32/1  "VOUTP_MidLvSaChkDTC_raw32"
  VDDM_MCUDisDTC_raw32/1 -> VDDM_MCUDisDTC_raw32_Inproc/1  "VDDM_MCUDisDTC_raw32"
  VDDM_MCUDisDTC_raw32_Inproc/1 -> UnitConverter278/1
  UnitConverter278/1 -> VOUTP_MCUDisDTC_raw32/1  "VOUTP_MCUDisDTC_raw32"
  VDDM_DCDCDisDTC_raw32/1 -> VDDM_DCDCDisDTC_raw32_Inproc/1  "VDDM_DCDCDisDTC_raw32"
  VDDM_DCDCDisDTC_raw32_Inproc/1 -> UnitConverter279/1
  UnitConverter279/1 -> VOUTP_DCDCDisDTC_raw32/1  "VOUTP_DCDCDisDTC_raw32"
  VDDM_HVRlyOpDTC_raw32/1 -> VDDM_HVRlyOpDTC_raw32_Inproc/1  "VDDM_HVRlyOpDTC_raw32"
  VDDM_HVRlyOpDTC_raw32_Inproc/1 -> UnitConverter280/1
  UnitConverter280/1 -> VOUTP_HVRlyOpDTC_raw32/1  "VOUTP_HVRlyOpDTC_raw32"
  VDDM_MCUActDTC_raw32/1 -> VDDM_MCUActDTC_raw32_Inproc/1  "VDDM_MCUActDTC_raw32"
  VDDM_MCUActDTC_raw32_Inproc/1 -> UnitConverter281/1
  UnitConverter281/1 -> VOUTP_MCUActDTC_raw32/1  "VOUTP_MCUActDTC_raw32"
  VDDM_OBC4PreDTC_raw32/1 -> VDDM_OBC4PreDTC_raw32_Inproc/1  "VDDM_OBC4PreDTC_raw32"
  VDDM_OBC4PreDTC_raw32_Inproc/1 -> UnitConverter282/1
  UnitConverter282/1 -> VOUTP_OBC4PreDTC_raw32/1  "VOUTP_OBC4PreDTC_raw32"
  VDDM_IniLVLoDTC_raw32/1 -> VDDM_IniLVLoDTC_raw32_Inproc/1  "VDDM_IniLVLoDTC_raw32"
  VDDM_IniLVLoDTC_raw32_Inproc/1 -> UnitConverter283/1
  UnitConverter283/1 -> VOUTP_IniLVLoDTC_raw32/1  "VOUTP_IniLVLoDTC_raw32"
  VDDM_LVSupLoDTC_raw32/1 -> VDDM_LVSupLoDTC_raw32_Inproc/1  "VDDM_LVSupLoDTC_raw32"
  VDDM_LVSupLoDTC_raw32_Inproc/1 -> UnitConverter284/1
  UnitConverter284/1 -> VOUTP_LVSupLoDTC_raw32/1  "VOUTP_LVSupLoDTC_raw32"
  VDDM_LVSupHiDTC_raw32/1 -> VDDM_LVSupHiDTC_raw32_Inproc/1  "VDDM_LVSupHiDTC_raw32"
  VDDM_LVSupHiDTC_raw32_Inproc/1 -> UnitConverter285/1
  UnitConverter285/1 -> VOUTP_LVSupHiDTC_raw32/1  "VOUTP_LVSupHiDTC_raw32"
  VDDM_DrStSWDTC_raw32/1 -> VDDM_DrStSWDTC_raw32_Inproc/1  "VDDM_DrStSWDTC_raw32"
  VDDM_DrStSWDTC_raw32_Inproc/1 -> UnitConverter286/1
  UnitConverter286/1 -> VOUTP_DrStSWDTC_raw32/1  "VOUTP_DrStSWDTC_raw32"
  VDDM_FLDoorSWDTC_raw32/1 -> VDDM_FLDoorSWDTC_raw32_Inproc/1  "VDDM_FLDoorSWDTC_raw32"
  VDDM_FLDoorSWDTC_raw32_Inproc/1 -> UnitConverter287/1
  UnitConverter287/1 -> VOUTP_FLDoorSWDTC_raw32/1  "VOUTP_FLDoorSWDTC_raw32"
  VDDM_RLDoorSWDTC_raw32/1 -> VDDM_RLDoorSWDTC_raw32_Inproc/1  "VDDM_RLDoorSWDTC_raw32"
  VDDM_RLDoorSWDTC_raw32_Inproc/1 -> UnitConverter288/1
  UnitConverter288/1 -> VOUTP_RLDoorSWDTC_raw32/1  "VOUTP_RLDoorSWDTC_raw32"
  VDDM_FRDoorSWDTC_raw32/1 -> VDDM_FRDoorSWDTC_raw32_Inproc/1  "VDDM_FRDoorSWDTC_raw32"
  VDDM_FRDoorSWDTC_raw32_Inproc/1 -> UnitConverter289/1
  UnitConverter289/1 -> VOUTP_FRDoorSWDTC_raw32/1  "VOUTP_FRDoorSWDTC_raw32"
  VDDM_RRDoorSWDTC_raw32/1 -> VDDM_RRDoorSWDTC_raw32_Inproc/1  "VDDM_RRDoorSWDTC_raw32"
  VDDM_RRDoorSWDTC_raw32_Inproc/1 -> UnitConverter290/1
  UnitConverter290/1 -> VOUTP_RRDoorSWDTC_raw32/1  "VOUTP_RRDoorSWDTC_raw32"
  VDDM_HoodSWDTC_raw32/1 -> VDDM_HoodSWDTC_raw32_Inproc/1  "VDDM_HoodSWDTC_raw32"
  VDDM_HoodSWDTC_raw32_Inproc/1 -> UnitConverter291/1
  UnitConverter291/1 -> VOUTP_HoodSWDTC_raw32/1  "VOUTP_HoodSWDTC_raw32"
  VDDM_TailgaSWDTC_raw32/1 -> VDDM_TailgaSWDTC_raw32_Inproc/1  "VDDM_TailgaSWDTC_raw32"
  VDDM_TailgaSWDTC_raw32_Inproc/1 -> UnitConverter292/1
  UnitConverter292/1 -> VOUTP_TailgaSWDTC_raw32/1  "VOUTP_TailgaSWDTC_raw32"
  VDDM_EDriveSysErrVCUErr_flg/1 -> VDDM_EDriveSysErrVCUErr_flg_Inproc/1  "VDDM_EDriveSysErrVCUErr_flg"
  VDDM_EDriveSysErrVCUErr_flg_Inproc/1 -> UnitConverter293/1
  UnitConverter293/1 -> VOUTP_EDriveSysErrVCUErr_flg/1  "VOUTP_EDriveSysErrVCUErr_flg"
  VDDM_VehMalfunLevel_enum/1 -> VDDM_VehMalfunLevel_enum_Inproc/1  "VDDM_VehMalfunLevel_enum"
  VDDM_VehMalfunLevel_enum_Inproc/1 -> UnitConverter294/1
  UnitConverter294/1 -> VOUTP_VehMalfunLevel_enum/1  "VOUTP_VehMalfunLevel_enum"
  VDDM_APS1SigOoRDTC_raw32/1 -> VDDM_APS1SigOoRDTC_raw32_Inproc/1  "VDDM_APS1SigOoRDTC_raw32"
  VDDM_APS1SigOoRDTC_raw32_Inproc/1 -> UnitConverter295/1
  UnitConverter295/1 -> VOUTP_APS1SigOoRDTC_raw32/1  "VOUTP_APS1SigOoRDTC_raw32"
  VDDM_APS2SigOoRDTC_raw32/1 -> VDDM_APS2SigOoRDTC_raw32_Inproc/1  "VDDM_APS2SigOoRDTC_raw32"
  VDDM_APS2SigOoRDTC_raw32_Inproc/1 -> UnitConverter296/1
  UnitConverter296/1 -> VOUTP_APS2SigOoRDTC_raw32/1  "VOUTP_APS2SigOoRDTC_raw32"
  VDDM_APSCorrErrDTC_raw32/1 -> VDDM_APSCorrErrDTC_raw32_Inproc/1  "VDDM_APSCorrErrDTC_raw32"
  VDDM_APSCorrErrDTC_raw32_Inproc/1 -> UnitConverter297/1
  UnitConverter297/1 -> VOUTP_APSCorrErrDTC_raw32/1  "VOUTP_APSCorrErrDTC_raw32"
  VDDM_MCUF1NoComDTC_raw32/1 -> VDDM_MCUF1NoComDTC_raw32_Inproc/1  "VDDM_MCUF1NoComDTC_raw32"
  VDDM_MCUF1NoComDTC_raw32_Inproc/1 -> UnitConverter298/1
  UnitConverter298/1 -> VOUTP_MCUF1NoComDTC_raw32/1  "VOUTP_MCUF1NoComDTC_raw32"
  VDDM_MCUR1NoComDTC_raw32/1 -> VDDM_MCUR1NoComDTC_raw32_Inproc/1  "VDDM_MCUR1NoComDTC_raw32"
  VDDM_MCUR1NoComDTC_raw32_Inproc/1 -> UnitConverter299/1
  UnitConverter299/1 -> VOUTP_MCUR1NoComDTC_raw32/1  "VOUTP_MCUR1NoComDTC_raw32"
  VDDM_Shifter1NoComDTC_raw32/1 -> VDDM_Shifter1NoComDTC_raw32_Inproc/1  "VDDM_Shifter1NoComDTC_raw32"
  VDDM_Shifter1NoComDTC_raw32_Inproc/1 -> UnitConverter300/1
  UnitConverter300/1 -> VOUTP_Shifter1NoComDTC_raw32/1  "VOUTP_Shifter1NoComDTC_raw32"
  VDDM_ESC7NoComDTC_raw32/1 -> VDDM_ESC7NoComDTC_raw32_Inproc/1  "VDDM_ESC7NoComDTC_raw32"
  VDDM_ESC7NoComDTC_raw32_Inproc/1 -> UnitConverter301/1
  UnitConverter301/1 -> VOUTP_ESC7NoComDTC_raw32/1  "VOUTP_ESC7NoComDTC_raw32"
  VDDM_ESC1NoComDTC_raw32/1 -> VDDM_ESC1NoComDTC_raw32_Inproc/1  "VDDM_ESC1NoComDTC_raw32"
  VDDM_ESC1NoComDTC_raw32_Inproc/1 -> UnitConverter302/1
  UnitConverter302/1 -> VOUTP_ESC1NoComDTC_raw32/1  "VOUTP_ESC1NoComDTC_raw32"
  VDDM_ESC5NoComDTC_raw32/1 -> VDDM_ESC5NoComDTC_raw32_Inproc/1  "VDDM_ESC5NoComDTC_raw32"
  VDDM_ESC5NoComDTC_raw32_Inproc/1 -> UnitConverter303/1
  UnitConverter303/1 -> VOUTP_ESC5NoComDTC_raw32/1  "VOUTP_ESC5NoComDTC_raw32"
  VDDM_EnterNewOperCyc_flg/1 -> VDDM_EnterNewOperCyc_flg_Inproc/1  "VDDM_EnterNewOperCyc_flg"
  VDDM_EnterNewOperCyc_flg_Inproc/1 -> UnitConverter304/1
  UnitConverter304/1 -> VOUTP_EnterNewOperCyc_flg/1  "VOUTP_EnterNewOperCyc_flg"
  VDDM_DiagHCrashDTC_raw32/1 -> VDDM_DiagHCrashDTC_raw32_Inproc/1  "VDDM_DiagHCrashDTC_raw32"
  VDDM_DiagHCrashDTC_raw32_Inproc/1 -> UnitConverter305/1
  UnitConverter305/1 -> VOUTP_DiagHCrashDTC_raw32/1  "VOUTP_DiagHCrashDTC_raw32"
  VDDM_DiagFLTSDTC_raw32/1 -> VDDM_DiagFLTSDTC_raw32_Inproc/1  "VDDM_DiagFLTSDTC_raw32"
  VDDM_DiagFLTSDTC_raw32_Inproc/1 -> UnitConverter306/1
  UnitConverter306/1 -> VOUTP_DiagFLTSDTC_raw32/1  "VOUTP_DiagFLTSDTC_raw32"
  VDDM_DiagFRTSDTC_raw32/1 -> VDDM_DiagFRTSDTC_raw32_Inproc/1  "VDDM_DiagFRTSDTC_raw32"
  VDDM_DiagFRTSDTC_raw32_Inproc/1 -> UnitConverter307/1
  UnitConverter307/1 -> VOUTP_DiagFRTSDTC_raw32/1  "VOUTP_DiagFRTSDTC_raw32"
  VDDM_DiagRLTSDTC_raw32/1 -> VDDM_DiagRLTSDTC_raw32_Inproc/1  "VDDM_DiagRLTSDTC_raw32"
  VDDM_DiagRLTSDTC_raw32_Inproc/1 -> UnitConverter308/1
  UnitConverter308/1 -> VOUTP_DiagRLTSDTC_raw32/1  "VOUTP_DiagRLTSDTC_raw32"
  VDDM_DiagRRTSDTC_raw32/1 -> VDDM_DiagRRTSDTC_raw32_Inproc/1  "VDDM_DiagRRTSDTC_raw32"
  VDDM_DiagRRTSDTC_raw32_Inproc/1 -> UnitConverter309/1
  UnitConverter309/1 -> VOUTP_DiagRRTSDTC_raw32/1  "VOUTP_DiagRRTSDTC_raw32"
  VDDM_FCLUSSDTC_raw32/1 -> VDDM_FCLUSSDTC_raw32_Inproc/1  "VDDM_FCLUSSDTC_raw32"
  VDDM_FCLUSSDTC_raw32_Inproc/1 -> UnitConverter310/1
  UnitConverter310/1 -> VOUTP_FCLUSSDTC_raw32/1  "VOUTP_FCLUSSDTC_raw32"
  VDDM_FMLUSSDTC_raw32/1 -> VDDM_FMLUSSDTC_raw32_Inproc/1  "VDDM_FMLUSSDTC_raw32"
  VDDM_FMLUSSDTC_raw32_Inproc/1 -> UnitConverter311/1
  UnitConverter311/1 -> VOUTP_FMLUSSDTC_raw32/1  "VOUTP_FMLUSSDTC_raw32"
  VDDM_FMRUSSDTC_raw32/1 -> VDDM_FMRUSSDTC_raw32_Inproc/1  "VDDM_FMRUSSDTC_raw32"
  VDDM_FMRUSSDTC_raw32_Inproc/1 -> UnitConverter312/1
  UnitConverter312/1 -> VOUTP_FMRUSSDTC_raw32/1  "VOUTP_FMRUSSDTC_raw32"
  VDDM_FCRUSSDTC_raw32/1 -> VDDM_FCRUSSDTC_raw32_Inproc/1  "VDDM_FCRUSSDTC_raw32"
  VDDM_FCRUSSDTC_raw32_Inproc/1 -> UnitConverter313/1
  UnitConverter313/1 -> VOUTP_FCRUSSDTC_raw32/1  "VOUTP_FCRUSSDTC_raw32"
  VDDM_RCLUSSDTC_raw32/1 -> VDDM_RCLUSSDTC_raw32_Inproc/1  "VDDM_RCLUSSDTC_raw32"
  VDDM_RCLUSSDTC_raw32_Inproc/1 -> UnitConverter314/1
  UnitConverter314/1 -> VOUTP_RCLUSSDTC_raw32/1  "VOUTP_RCLUSSDTC_raw32"
  VDDM_RMLUSSDTC_raw32/1 -> VDDM_RMLUSSDTC_raw32_Inproc/1  "VDDM_RMLUSSDTC_raw32"
  VDDM_RMLUSSDTC_raw32_Inproc/1 -> UnitConverter315/1
  UnitConverter315/1 -> VOUTP_RMLUSSDTC_raw32/1  "VOUTP_RMLUSSDTC_raw32"
  VDDM_RMRUSSDTC_raw32/1 -> VDDM_RMRUSSDTC_raw32_Inproc/1  "VDDM_RMRUSSDTC_raw32"
  VDDM_RMRUSSDTC_raw32_Inproc/1 -> UnitConverter316/1
  UnitConverter316/1 -> VOUTP_RMRUSSDTC_raw32/1  "VOUTP_RMRUSSDTC_raw32"
  VDDM_RCRUSSDTC_raw32/1 -> VDDM_RCRUSSDTC_raw32_Inproc/1  "VDDM_RCRUSSDTC_raw32"
  VDDM_RCRUSSDTC_raw32_Inproc/1 -> UnitConverter317/1
  UnitConverter317/1 -> VOUTP_RCRUSSDTC_raw32/1  "VOUTP_RCRUSSDTC_raw32"
  VDDM_FLLUSSDTC_raw32/1 -> VDDM_FLLUSSDTC_raw32_Inproc/1  "VDDM_FLLUSSDTC_raw32"
  VDDM_FLLUSSDTC_raw32_Inproc/1 -> UnitConverter318/1
  UnitConverter318/1 -> VOUTP_FLLUSSDTC_raw32/1  "VOUTP_FLLUSSDTC_raw32"
  VDDM_FLRUSSDTC_raw32/1 -> VDDM_FLRUSSDTC_raw32_Inproc/1  "VDDM_FLRUSSDTC_raw32"
  VDDM_FLRUSSDTC_raw32_Inproc/1 -> UnitConverter319/1
  UnitConverter319/1 -> VOUTP_FLRUSSDTC_raw32/1  "VOUTP_FLRUSSDTC_raw32"
  VDDM_RLLUSSDTC_raw32/1 -> VDDM_RLLUSSDTC_raw32_Inproc/1  "VDDM_RLLUSSDTC_raw32"
  VDDM_RLLUSSDTC_raw32_Inproc/1 -> UnitConverter320/1
  UnitConverter320/1 -> VOUTP_RLLUSSDTC_raw32/1  "VOUTP_RLLUSSDTC_raw32"
  VDDM_RLRUSSDTC_raw32/1 -> VDDM_RLRUSSDTC_raw32_Inproc/1  "VDDM_RLRUSSDTC_raw32"
  VDDM_RLRUSSDTC_raw32_Inproc/1 -> UnitConverter321/1
  UnitConverter321/1 -> VOUTP_RLRUSSDTC_raw32/1  "VOUTP_RLRUSSDTC_raw32"
  VDDM_FCM2NoComDTC_raw32/1 -> VDDM_FCM2NoComDTC_raw32_Inproc/1  "VDDM_FCM2NoComDTC_raw32"
  VDDM_FCM2NoComDTC_raw32_Inproc/1 -> UnitConverter322/1
  UnitConverter322/1 -> VOUTP_FCM2NoComDTC_raw32/1  "VOUTP_FCM2NoComDTC_raw32"
  VDDM_FCM2RCErrDTC_raw32/1 -> VDDM_FCM2RCErrDTC_raw32_Inproc/1  "VDDM_FCM2RCErrDTC_raw32"
  VDDM_FCM2RCErrDTC_raw32_Inproc/1 -> UnitConverter323/1
  UnitConverter323/1 -> VOUTP_FCM2RCErrDTC_raw32/1  "VOUTP_FCM2RCErrDTC_raw32"
  VDDM_FCM2CSErrDTC_raw32/1 -> VDDM_FCM2CSErrDTC_raw32_Inproc/1  "VDDM_FCM2CSErrDTC_raw32"
  VDDM_FCM2CSErrDTC_raw32_Inproc/1 -> UnitConverter324/1
  UnitConverter324/1 -> VOUTP_FCM2CSErrDTC_raw32/1  "VOUTP_FCM2CSErrDTC_raw32"
  VDDM_FCM3NoComDTC_raw32/1 -> VDDM_FCM3NoComDTC_raw32_Inproc/1  "VDDM_FCM3NoComDTC_raw32"
  VDDM_FCM3NoComDTC_raw32_Inproc/1 -> UnitConverter325/1
  UnitConverter325/1 -> VOUTP_FCM3NoComDTC_raw32/1  "VOUTP_FCM3NoComDTC_raw32"
  VDDM_FCM3RCErrDTC_raw32/1 -> VDDM_FCM3RCErrDTC_raw32_Inproc/1  "VDDM_FCM3RCErrDTC_raw32"
  VDDM_FCM3RCErrDTC_raw32_Inproc/1 -> UnitConverter326/1
  UnitConverter326/1 -> VOUTP_FCM3RCErrDTC_raw32/1  "VOUTP_FCM3RCErrDTC_raw32"
  VDDM_FCM3CSErrDTC_raw32/1 -> VDDM_FCM3CSErrDTC_raw32_Inproc/1  "VDDM_FCM3CSErrDTC_raw32"
  VDDM_FCM3CSErrDTC_raw32_Inproc/1 -> UnitConverter327/1
  UnitConverter327/1 -> VOUTP_FCM3CSErrDTC_raw32/1  "VOUTP_FCM3CSErrDTC_raw32"
  VDDM_FCM4NoComDTC_raw32/1 -> VDDM_FCM4NoComDTC_raw32_Inproc/1  "VDDM_FCM4NoComDTC_raw32"
  VDDM_FCM4NoComDTC_raw32_Inproc/1 -> UnitConverter328/1
  UnitConverter328/1 -> VOUTP_FCM4NoComDTC_raw32/1  "VOUTP_FCM4NoComDTC_raw32"
  VDDM_FCM4CSErrDTC_raw32/1 -> VDDM_FCM4CSErrDTC_raw32_Inproc/1  "VDDM_FCM4CSErrDTC_raw32"
  VDDM_FCM4CSErrDTC_raw32_Inproc/1 -> UnitConverter329/1
  UnitConverter329/1 -> VOUTP_FCM4CSErrDTC_raw32/1  "VOUTP_FCM4CSErrDTC_raw32"
  VDDM_FCM5NoComDTC_raw32/1 -> VDDM_FCM5NoComDTC_raw32_Inproc/1  "VDDM_FCM5NoComDTC_raw32"
  VDDM_FCM5NoComDTC_raw32_Inproc/1 -> UnitConverter330/1
  UnitConverter330/1 -> VOUTP_FCM5NoComDTC_raw32/1  "VOUTP_FCM5NoComDTC_raw32"
  VDDM_FCM5CSErrDTC_raw32/1 -> VDDM_FCM5CSErrDTC_raw32_Inproc/1  "VDDM_FCM5CSErrDTC_raw32"
  VDDM_FCM5CSErrDTC_raw32_Inproc/1 -> UnitConverter331/1
  UnitConverter331/1 -> VOUTP_FCM5CSErrDTC_raw32/1  "VOUTP_FCM5CSErrDTC_raw32"
  VDDM_ZoneSCPNoComDTC_raw32/1 -> VDDM_ZoneSCPNoComDTC_raw32_Inproc/1  "VDDM_ZoneSCPNoComDTC_raw32"
  VDDM_ZoneSCPNoComDTC_raw32_Inproc/1 -> UnitConverter332/1
  UnitConverter332/1 -> VOUTP_ZoneSCPNoComDTC_raw32/1  "VOUTP_ZoneSCPNoComDTC_raw32"
  VDDM_BMSSigErrDetDTC_raw32/1 -> VDDM_BMSSigErrDetDTC_raw32_Inproc/1  "VDDM_BMSSigErrDetDTC_raw32"
  VDDM_BMSSigErrDetDTC_raw32_Inproc/1 -> UnitConverter333/1
  UnitConverter333/1 -> VOUTP_BMSSigErrDetDTC_raw32/1  "VOUTP_BMSSigErrDetDTC_raw32"
  VDDM_FCMACCSigErrDetDTC_raw32/1 -> VDDM_FCMACCSigErrDetDTC_raw32_Inproc/1  "VDDM_FCMACCSigErrDetDTC_raw32"
  VDDM_FCMACCSigErrDetDTC_raw32_Inproc/1 -> UnitConverter334/1
  UnitConverter334/1 -> VOUTP_FCMACCSigErrDetDTC_raw32/1  "VOUTP_FCMACCSigErrDetDTC_raw32"
  VDDM_FrMCUSigErrDetDTC_raw32/1 -> VDDM_FrMCUSigErrDetDTC_raw32_Inproc/1  "VDDM_FrMCUSigErrDetDTC_raw32"
  VDDM_FrMCUSigErrDetDTC_raw32_Inproc/1 -> UnitConverter335/1
  UnitConverter335/1 -> VOUTP_FrMCUSigErrDetDTC_raw32/1  "VOUTP_FrMCUSigErrDetDTC_raw32"
  VDDM_RrMCUSigErrDetDTC_raw32/1 -> VDDM_RrMCUSigErrDetDTC_raw32_Inproc/1  "VDDM_RrMCUSigErrDetDTC_raw32"
  VDDM_RrMCUSigErrDetDTC_raw32_Inproc/1 -> UnitConverter336/1
  UnitConverter336/1 -> VOUTP_RrMCUSigErrDetDTC_raw32/1  "VOUTP_RrMCUSigErrDetDTC_raw32"
  VDDM_CCUSigErrDetDTC_raw32/1 -> VDDM_CCUSigErrDetDTC_raw32_Inproc/1  "VDDM_CCUSigErrDetDTC_raw32"
  VDDM_CCUSigErrDetDTC_raw32_Inproc/1 -> UnitConverter337/1
  UnitConverter337/1 -> VOUTP_CCUSigErrDetDTC_raw32/1  "VOUTP_CCUSigErrDetDTC_raw32"
  VDDM_ACCAccelCmdErrDetDTC_raw32/1 -> VDDM_ACCAccelCmdErrDetDTC_raw32_Inproc/1  "VDDM_ACCAccelCmdErrDetDTC_raw32"
  VDDM_ACCAccelCmdErrDetDTC_raw32_Inproc/1 -> UnitConverter338/1
  UnitConverter338/1 -> VOUTP_ACCAccelCmdErrDetDTC_raw32/1  "VOUTP_ACCAccelCmdErrDetDTC_raw32"
  VDDM_ACCMalfuncDetDTC_raw32/1 -> VDDM_ACCMalfuncDetDTC_raw32_Inproc/1  "VDDM_ACCMalfuncDetDTC_raw32"
  VDDM_ACCMalfuncDetDTC_raw32_Inproc/1 -> UnitConverter339/1
  UnitConverter339/1 -> VOUTP_ACCMalfuncDetDTC_raw32/1  "VOUTP_ACCMalfuncDetDTC_raw32"
  VDDM_CCMalfuncDetDTC_raw32/1 -> VDDM_CCMalfuncDetDTC_raw32_Inproc/1  "VDDM_CCMalfuncDetDTC_raw32"
  VDDM_CCMalfuncDetDTC_raw32_Inproc/1 -> UnitConverter340/1
  UnitConverter340/1 -> VOUTP_CCMalfuncDetDTC_raw32/1  "VOUTP_CCMalfuncDetDTC_raw32"
  VDDM_MSAMalfuncDetDTC_raw32/1 -> VDDM_MSAMalfuncDetDTC_raw32_Inproc/1  "VDDM_MSAMalfuncDetDTC_raw32"
  VDDM_MSAMalfuncDetDTC_raw32_Inproc/1 -> UnitConverter341/1
  UnitConverter341/1 -> VOUTP_MSAMalfuncDetDTC_raw32/1  "VOUTP_MSAMalfuncDetDTC_raw32"
  VDDM_ISAMalfuncDetDTC_raw32/1 -> VDDM_ISAMalfuncDetDTC_raw32_Inproc/1  "VDDM_ISAMalfuncDetDTC_raw32"
  VDDM_ISAMalfuncDetDTC_raw32_Inproc/1 -> UnitConverter342/1
  UnitConverter342/1 -> VOUTP_ISAMalfuncDetDTC_raw32/1  "VOUTP_ISAMalfuncDetDTC_raw32"
  VDDM_MCUF1RCErrDTC_raw32/1 -> VDDM_MCUF1RCErrDTC_raw32_Inproc/1  "VDDM_MCUF1RCErrDTC_raw32"
  VDDM_MCUF1RCErrDTC_raw32_Inproc/1 -> UnitConverter343/1
  UnitConverter343/1 -> VOUTP_MCUF1RCErrDTC_raw32/1  "VOUTP_MCUF1RCErrDTC_raw32"
  VDDM_MCUR1RCErrDTC_raw32/1 -> VDDM_MCUR1RCErrDTC_raw32_Inproc/1  "VDDM_MCUR1RCErrDTC_raw32"
  VDDM_MCUR1RCErrDTC_raw32_Inproc/1 -> UnitConverter344/1
  UnitConverter344/1 -> VOUTP_MCUR1RCErrDTC_raw32/1  "VOUTP_MCUR1RCErrDTC_raw32"
  VDDM_MCUF1CSErrDTC_raw32/1 -> VDDM_MCUF1CSErrDTC_raw32_Inproc/1  "VDDM_MCUF1CSErrDTC_raw32"
  VDDM_MCUF1CSErrDTC_raw32_Inproc/1 -> UnitConverter345/1
  UnitConverter345/1 -> VOUTP_MCUF1CSErrDTC_raw32/1  "VOUTP_MCUF1CSErrDTC_raw32"
  VDDM_MCUR1CSErrDTC_raw32/1 -> VDDM_MCUR1CSErrDTC_raw32_Inproc/1  "VDDM_MCUR1CSErrDTC_raw32"
  VDDM_MCUR1CSErrDTC_raw32_Inproc/1 -> UnitConverter346/1
  UnitConverter346/1 -> VOUTP_MCUR1CSErrDTC_raw32/1  "VOUTP_MCUR1CSErrDTC_raw32"
  VDDM_Shifter1RCErrDTC_raw32/1 -> VDDM_Shifter1RCErrDTC_raw32_Inproc/1  "VDDM_Shifter1RCErrDTC_raw32"
  VDDM_Shifter1RCErrDTC_raw32_Inproc/1 -> UnitConverter347/1
  UnitConverter347/1 -> VOUTP_Shifter1RCErrDTC_raw32/1  "VOUTP_Shifter1RCErrDTC_raw32"
  VDDM_Shifter1CSErrDTC_raw32/1 -> VDDM_Shifter1CSErrDTC_raw32_Inproc/1  "VDDM_Shifter1CSErrDTC_raw32"
  VDDM_Shifter1CSErrDTC_raw32_Inproc/1 -> UnitConverter348/1
  UnitConverter348/1 -> VOUTP_Shifter1CSErrDTC_raw32/1  "VOUTP_Shifter1CSErrDTC_raw32"
  VDDM_ESC7RCErrDTC_raw32/1 -> VDDM_ESC7RCErrDTC_raw32_Inproc/1  "VDDM_ESC7RCErrDTC_raw32"
  VDDM_ESC7RCErrDTC_raw32_Inproc/1 -> UnitConverter349/1
  UnitConverter349/1 -> VOUTP_ESC7RCErrDTC_raw32/1  "VOUTP_ESC7RCErrDTC_raw32"
  VDDM_ESC7CSErrDTC_raw32/1 -> VDDM_ESC7CSErrDTC_raw32_Inproc/1  "VDDM_ESC7CSErrDTC_raw32"
  VDDM_ESC7CSErrDTC_raw32_Inproc/1 -> UnitConverter350/1
  UnitConverter350/1 -> VOUTP_ESC7CSErrDTC_raw32/1  "VOUTP_ESC7CSErrDTC_raw32"
  VDDM_ESC1RCErrDTC_raw32/1 -> VDDM_ESC1RCErrDTC_raw32_Inproc/1  "VDDM_ESC1RCErrDTC_raw32"
  VDDM_ESC1RCErrDTC_raw32_Inproc/1 -> UnitConverter351/1
  UnitConverter351/1 -> VOUTP_ESC1RCErrDTC_raw32/1  "VOUTP_ESC1RCErrDTC_raw32"
  VDDM_ESC1CSErrDTC_raw32/1 -> VDDM_ESC1CSErrDTC_raw32_Inproc/1  "VDDM_ESC1CSErrDTC_raw32"
  VDDM_ESC1CSErrDTC_raw32_Inproc/1 -> UnitConverter352/1
  UnitConverter352/1 -> VOUTP_ESC1CSErrDTC_raw32/1  "VOUTP_ESC1CSErrDTC_raw32"
  VDDM_ESC5RCErrDTC_raw32/1 -> VDDM_ESC5RCErrDTC_raw32_Inproc/1  "VDDM_ESC5RCErrDTC_raw32"
  VDDM_ESC5RCErrDTC_raw32_Inproc/1 -> UnitConverter353/1
  UnitConverter353/1 -> VOUTP_ESC5RCErrDTC_raw32/1  "VOUTP_ESC5RCErrDTC_raw32"
  VDDM_ESC5CSErrDTC_raw32/1 -> VDDM_ESC5CSErrDTC_raw32_Inproc/1  "VDDM_ESC5CSErrDTC_raw32"
  VDDM_ESC5CSErrDTC_raw32_Inproc/1 -> UnitConverter354/1
  UnitConverter354/1 -> VOUTP_ESC5CSErrDTC_raw32/1  "VOUTP_ESC5CSErrDTC_raw32"
  VDDM_FrMCUTqErrDTC_raw32/1 -> VDDM_FrMCUTqErrDTC_raw32_Inproc/1  "VDDM_FrMCUTqErrDTC_raw32"
  VDDM_FrMCUTqErrDTC_raw32_Inproc/1 -> UnitConverter355/1
  UnitConverter355/1 -> VOUTP_FrMCUTqErrDTC_raw32/1  "VOUTP_FrMCUTqErrDTC_raw32"
  VDDM_RrMCUTqErrDTC_raw32/1 -> VDDM_RrMCUTqErrDTC_raw32_Inproc/1  "VDDM_RrMCUTqErrDTC_raw32"
  VDDM_RrMCUTqErrDTC_raw32_Inproc/1 -> UnitConverter356/1
  UnitConverter356/1 -> VOUTP_RrMCUTqErrDTC_raw32/1  "VOUTP_RrMCUTqErrDTC_raw32"
  VDDM_LFBatwarnDTC_raw32/1 -> VDDM_LFBatwarnDTC_raw32_Inproc/1  "VDDM_LFBatwarnDTC_raw32"
  VDDM_LFBatwarnDTC_raw32_Inproc/1 -> UnitConverter357/1
  UnitConverter357/1 -> VOUTP_LFBatwarnDTC_raw32/1  "VOUTP_LFBatwarnDTC_raw32"
  VDDM_RFBatwarnDTC_raw32/1 -> VDDM_RFBatwarnDTC_raw32_Inproc/1  "VDDM_RFBatwarnDTC_raw32"
  VDDM_RFBatwarnDTC_raw32_Inproc/1 -> UnitConverter358/1
  UnitConverter358/1 -> VOUTP_RFBatwarnDTC_raw32/1  "VOUTP_RFBatwarnDTC_raw32"
  VDDM_LRBatwarnDTC_raw32/1 -> VDDM_LRBatwarnDTC_raw32_Inproc/1  "VDDM_LRBatwarnDTC_raw32"
  VDDM_LRBatwarnDTC_raw32_Inproc/1 -> UnitConverter359/1
  UnitConverter359/1 -> VOUTP_LRBatwarnDTC_raw32/1  "VOUTP_LRBatwarnDTC_raw32"
  VDDM_RRBatwarnDTC_raw32/1 -> VDDM_RRBatwarnDTC_raw32_Inproc/1  "VDDM_RRBatwarnDTC_raw32"
  VDDM_RRBatwarnDTC_raw32_Inproc/1 -> UnitConverter360/1
  UnitConverter360/1 -> VOUTP_RRBatwarnDTC_raw32/1  "VOUTP_RRBatwarnDTC_raw32"
  VDDM_LFPressIndiDTC_raw32/1 -> VDDM_LFPressIndiDTC_raw32_Inproc/1  "VDDM_LFPressIndiDTC_raw32"
  VDDM_LFPressIndiDTC_raw32_Inproc/1 -> UnitConverter361/1
  UnitConverter361/1 -> VOUTP_LFPressIndiDTC_raw32/1  "VOUTP_LFPressIndiDTC_raw32"
  VDDM_RFPressIndiDTC_raw32/1 -> VDDM_RFPressIndiDTC_raw32_Inproc/1  "VDDM_RFPressIndiDTC_raw32"
  VDDM_RFPressIndiDTC_raw32_Inproc/1 -> UnitConverter362/1
  UnitConverter362/1 -> VOUTP_RFPressIndiDTC_raw32/1  "VOUTP_RFPressIndiDTC_raw32"
  VDDM_LRPressIndiDTC_raw32/1 -> VDDM_LRPressIndiDTC_raw32_Inproc/1  "VDDM_LRPressIndiDTC_raw32"
  VDDM_LRPressIndiDTC_raw32_Inproc/1 -> UnitConverter363/1
  UnitConverter363/1 -> VOUTP_LRPressIndiDTC_raw32/1  "VOUTP_LRPressIndiDTC_raw32"
  VDDM_RRPressIndiDTC_raw32/1 -> VDDM_RRPressIndiDTC_raw32_Inproc/1  "VDDM_RRPressIndiDTC_raw32"
  VDDM_RRPressIndiDTC_raw32_Inproc/1 -> UnitConverter364/1
  UnitConverter364/1 -> VOUTP_RRPressIndiDTC_raw32/1  "VOUTP_RRPressIndiDTC_raw32"
  VDDM_LFWheelTmpHighDTC_raw32/1 -> VDDM_LFWheelTmpHighDTC_raw32_Inproc/1  "VDDM_LFWheelTmpHighDTC_raw32"
  VDDM_LFWheelTmpHighDTC_raw32_Inproc/1 -> UnitConverter365/1
  UnitConverter365/1 -> VOUTP_LFWheelTmpHighDTC_raw32/1  "VOUTP_LFWheelTmpHighDTC_raw32"
  VDDM_RFWheelTmpHighDTC_raw32/1 -> VDDM_RFWheelTmpHighDTC_raw32_Inproc/1  "VDDM_RFWheelTmpHighDTC_raw32"
  VDDM_RFWheelTmpHighDTC_raw32_Inproc/1 -> UnitConverter366/1
  UnitConverter366/1 -> VOUTP_RFWheelTmpHighDTC_raw32/1  "VOUTP_RFWheelTmpHighDTC_raw32"
  VDDM_LRWheelTmpHighDTC_raw32/1 -> VDDM_LRWheelTmpHighDTC_raw32_Inproc/1  "VDDM_LRWheelTmpHighDTC_raw32"
  VDDM_LRWheelTmpHighDTC_raw32_Inproc/1 -> UnitConverter367/1
  UnitConverter367/1 -> VOUTP_LRWheelTmpHighDTC_raw32/1  "VOUTP_LRWheelTmpHighDTC_raw32"
  VDDM_RRWheelTmpHighDTC_raw32/1 -> VDDM_RRWheelTmpHighDTC_raw32_Inproc/1  "VDDM_RRWheelTmpHighDTC_raw32"
  VDDM_RRWheelTmpHighDTC_raw32_Inproc/1 -> UnitConverter368/1
  UnitConverter368/1 -> VOUTP_RRWheelTmpHighDTC_raw32/1  "VOUTP_RRWheelTmpHighDTC_raw32"
  VDDM_LFSensorFailDTC_raw32/1 -> VDDM_LFSensorFailDTC_raw32_Inproc/1  "VDDM_LFSensorFailDTC_raw32"
  VDDM_LFSensorFailDTC_raw32_Inproc/1 -> UnitConverter369/1
  UnitConverter369/1 -> VOUTP_LFSensorFailDTC_raw32/1  "VOUTP_LFSensorFailDTC_raw32"
  VDDM_RFSensorFailDTC_raw32/1 -> VDDM_RFSensorFailDTC_raw32_Inproc/1  "VDDM_RFSensorFailDTC_raw32"
  VDDM_RFSensorFailDTC_raw32_Inproc/1 -> UnitConverter370/1
  UnitConverter370/1 -> VOUTP_RFSensorFailDTC_raw32/1  "VOUTP_RFSensorFailDTC_raw32"
  VDDM_LRSensorFailDTC_raw32/1 -> VDDM_LRSensorFailDTC_raw32_Inproc/1  "VDDM_LRSensorFailDTC_raw32"
  VDDM_LRSensorFailDTC_raw32_Inproc/1 -> UnitConverter371/1
  UnitConverter371/1 -> VOUTP_LRSensorFailDTC_raw32/1  "VOUTP_LRSensorFailDTC_raw32"
  VDDM_RRSensorFailDTC_raw32/1 -> VDDM_RRSensorFailDTC_raw32_Inproc/1  "VDDM_RRSensorFailDTC_raw32"
  VDDM_RRSensorFailDTC_raw32_Inproc/1 -> UnitConverter372/1
  UnitConverter372/1 -> VOUTP_RRSensorFailDTC_raw32/1  "VOUTP_RRSensorFailDTC_raw32"
  VDDM_C1EPAS2LCDTC_raw32/1 -> VDDM_C1EPAS2LCDTC_raw32_Inproc/1  "VDDM_C1EPAS2LCDTC_raw32"
  VDDM_C1EPAS2LCDTC_raw32_Inproc/1 -> UnitConverter373/1
  UnitConverter373/1 -> VOUTP_C1EPAS2LCDTC_raw32/1  "VOUTP_C1EPAS2LCDTC_raw32"
  VDDM_5vAPS1PwrErrDTC_raw32/1 -> VDDM_5vAPS1PwrErrDTC_raw32_Inproc/1  "VDDM_5vAPS1PwrErrDTC_raw32"
  VDDM_5vAPS1PwrErrDTC_raw32_Inproc/1 -> UnitConverter374/1
  UnitConverter374/1 -> VOUTP_5vAPS1PwrErrDTC_raw32/1  "VOUTP_5vAPS1PwrErrDTC_raw32"
  VDDM_5vAPS2PwrErrDTC_raw32/1 -> VDDM_5vAPS2PwrErrDTC_raw32_Inproc/1  "VDDM_5vAPS2PwrErrDTC_raw32"
  VDDM_5vAPS2PwrErrDTC_raw32_Inproc/1 -> UnitConverter375/1
  UnitConverter375/1 -> VOUTP_5vAPS2PwrErrDTC_raw32/1  "VOUTP_5vAPS2PwrErrDTC_raw32"
  VDDM_EPBLockTODTC_raw32/1 -> VDDM_EPBLockTODTC_raw32_Inproc/1  "VDDM_EPBLockTODTC_raw32"
  VDDM_EPBLockTODTC_raw32_Inproc/1 -> UnitConverter376/1
  UnitConverter376/1 -> VOUTP_EPBLockTODTC_raw32/1  "VOUTP_EPBLockTODTC_raw32"
  VDDM_EPBUnlockTODTC_raw32/1 -> VDDM_EPBUnlockTODTC_raw32_Inproc/1  "VDDM_EPBUnlockTODTC_raw32"
  VDDM_EPBUnlockTODTC_raw32_Inproc/1 -> UnitConverter377/1
  UnitConverter377/1 -> VOUTP_EPBUnlockTODTC_raw32/1  "VOUTP_EPBUnlockTODTC_raw32"
  VDDM_LimpHomeActTmp_flg/1 -> VDDM_LimpHomeActTmp_flg_Inproc/1  "VDDM_LimpHomeActTmp_flg"
  VDDM_LimpHomeActTmp_flg_Inproc/1 -> UnitConverter378/1
  UnitConverter378/1 -> VOUTP_LimpHomeActTmp_flg/1  "VOUTP_LimpHomeActTmp_flg"
  VDDM_DTCDetect_enum/1 -> VDDM_DTCDetect_enum_Inproc/1  "VDDM_DTCDetect_enum"
  VDDM_DTCDetect_enum_Inproc/1 -> UnitConverter379/1
  UnitConverter379/1 -> VOUTP_DTCDetect_enum/1  "VOUTP_DTCDetect_enum"
  VDDM_EngagePFail_flg/1 -> VDDM_EngagePFail_flg_Inproc/1  "VDDM_EngagePFail_flg"
  VDDM_EngagePFail_flg_Inproc/1 -> UnitConverter380/1
  UnitConverter380/1 -> VOUTP_EngagePFail_flg/1  "VOUTP_EngagePFail_flg"
  VDDM_DisengagePFail_flg/1 -> VDDM_DisengagePFail_flg_Inproc/1  "VDDM_DisengagePFail_flg"
  VDDM_DisengagePFail_flg_Inproc/1 -> UnitConverter381/1
  UnitConverter381/1 -> VOUTP_DisengagePFail_flg/1  "VOUTP_DisengagePFail_flg"
  VDDM_VCURAPSErrLv2_flg/1 -> VDDM_VCURAPSErrLv2_flg_Inproc/1  "VDDM_VCURAPSErrLv2_flg"
  VDDM_VCURAPSErrLv2_flg_Inproc/1 -> UnitConverter382/1
  UnitConverter382/1 -> VOUTP_VCURAPSErrLv2_flg/1  "VOUTP_VCURAPSErrLv2_flg"
  VDDM_VCURAPSErrLv3_flg/1 -> VDDM_VCURAPSErrLv3_flg_Inproc/1  "VDDM_VCURAPSErrLv3_flg"
  VDDM_VCURAPSErrLv3_flg_Inproc/1 -> UnitConverter383/1
  UnitConverter383/1 -> VOUTP_VCURAPSErrLv3_flg/1  "VOUTP_VCURAPSErrLv3_flg"
  VDDM_EDriveSysErrShifterErr_flg/1 -> VDDM_EDriveSysErrShifterErr_flg_Inproc/1  "VDDM_EDriveSysErrShifterErr_flg"
  VDDM_EDriveSysErrShifterErr_flg_Inproc/1 -> UnitConverter384/1
  UnitConverter384/1 -> VOUTP_EDriveSysErrShifterErr_flg/1  "VOUTP_EDriveSysErrShifterErr_flg"
  VDDM_LVSysErrPwrOutErr_flg/1 -> VDDM_LVSysErrPwrOutErr_flg_Inproc/1  "VDDM_LVSysErrPwrOutErr_flg"
  VDDM_LVSysErrPwrOutErr_flg_Inproc/1 -> UnitConverter385/1
  UnitConverter385/1 -> VOUTP_LVSysErrPwrOutErr_flg/1  "VOUTP_LVSysErrPwrOutErr_flg"
  VDDM_HVRlyOpFail_flg/1 -> VDDM_HVRlyOpFail_flg_Inproc/1  "VDDM_HVRlyOpFail_flg"
  VDDM_HVRlyOpFail_flg_Inproc/1 -> UnitConverter386/1
  UnitConverter386/1 -> VOUTP_HVRlyOpFail_flg/1  "VOUTP_HVRlyOpFail_flg"
  VDDM_MCUActDisFail_flg/1 -> VDDM_MCUActDisFail_flg_Inproc/1  "VDDM_MCUActDisFail_flg"
  VDDM_MCUActDisFail_flg_Inproc/1 -> UnitConverter387/1
  UnitConverter387/1 -> VOUTP_MCUActDisFail_flg/1  "VOUTP_MCUActDisFail_flg"
  VDDM_VCUBrkSWSta_enum/1 -> VDDM_VCUBrkSWSta_enum_Inproc/1  "VDDM_VCUBrkSWSta_enum"
  VDDM_VCUBrkSWSta_enum_Inproc/1 -> UnitConverter388/1
  UnitConverter388/1 -> VOUTP_VCUBrkSWSta_enum/1  "VOUTP_VCUBrkSWSta_enum"
  VDDM_VCUFLDoorSta_flg/1 -> VDDM_VCUFLDoorSta_flg_Inproc/1  "VDDM_VCUFLDoorSta_flg"
  VDDM_VCUFLDoorSta_flg_Inproc/1 -> UnitConverter389/1
  UnitConverter389/1 -> VOUTP_VCUFLDoorSta_flg/1  "VOUTP_VCUFLDoorSta_flg"
  VDDM_VCUFRDoorSta_flg/1 -> VDDM_VCUFRDoorSta_flg_Inproc/1  "VDDM_VCUFRDoorSta_flg"
  VDDM_VCUFRDoorSta_flg_Inproc/1 -> UnitConverter390/1
  UnitConverter390/1 -> VOUTP_VCUFRDoorSta_flg/1  "VOUTP_VCUFRDoorSta_flg"
  VDDM_VCURLDoorSta_flg/1 -> VDDM_VCURLDoorSta_flg_Inproc/1  "VDDM_VCURLDoorSta_flg"
  VDDM_VCURLDoorSta_flg_Inproc/1 -> UnitConverter391/1
  UnitConverter391/1 -> VOUTP_VCURLDoorSta_flg/1  "VOUTP_VCURLDoorSta_flg"
  VDDM_VCURRDoorSta_flg/1 -> VDDM_VCURRDoorSta_flg_Inproc/1  "VDDM_VCURRDoorSta_flg"
  VDDM_VCURRDoorSta_flg_Inproc/1 -> UnitConverter392/1
  UnitConverter392/1 -> VOUTP_VCURRDoorSta_flg/1  "VOUTP_VCURRDoorSta_flg"
  VDDM_SysAllowReadySta_flg/1 -> VDDM_SysAllowReadySta_flg_Inproc/1  "VDDM_SysAllowReadySta_flg"
  VDDM_SysAllowReadySta_flg_Inproc/1 -> UnitConverter393/1
  UnitConverter393/1 -> VOUTP_SysAllowReadySta_flg/1  "VOUTP_SysAllowReadySta_flg"
  VDDM_VCUHoodSWSta_flg/1 -> VDDM_VCUHoodSWSta_flg_Inproc/1  "VDDM_VCUHoodSWSta_flg"
  VDDM_VCUHoodSWSta_flg_Inproc/1 -> UnitConverter394/1
  UnitConverter394/1 -> VOUTP_VCUHoodSWSta_flg/1  "VOUTP_VCUHoodSWSta_flg"
  VDDM_VCUTailgateSWSta_flg/1 -> VDDM_VCUTailgateSWSta_flg_Inproc/1  "VDDM_VCUTailgateSWSta_flg"
  VDDM_VCUTailgateSWSta_flg_Inproc/1 -> UnitConverter395/1
  UnitConverter395/1 -> VOUTP_VCUTailgateSWSta_flg/1  "VOUTP_VCUTailgateSWSta_flg"
  VDHP_ActAPSPosn_pct/1 -> VDHP_ActAPSPosn_pct_Inproc/1  "VDHP_ActAPSPosn_pct"
  VDHP_ActAPSPosn_pct_Inproc/1 -> UnitConverter396/1
  UnitConverter396/1 -> VOUTP_ActAPSPosn_pct/1  "VOUTP_ActAPSPosn_pct"
  VDHP_EAPS1MIN_pct/1 -> VDHP_EAPS1MIN_pct_Inproc/1  "VDHP_EAPS1MIN_pct"
  VDHP_EAPS1MIN_pct_Inproc/1 -> UnitConverter397/1
  UnitConverter397/1 -> VOUTP_EAPS1MIN_pct/1  "VOUTP_EAPS1MIN_pct"
  VDHP_EAPS2MIN_pct/1 -> VDHP_EAPS2MIN_pct_Inproc/1  "VDHP_EAPS2MIN_pct"
  VDHP_EAPS2MIN_pct_Inproc/1 -> UnitConverter398/1
  UnitConverter398/1 -> VOUTP_EAPS2MIN_pct/1  "VOUTP_EAPS2MIN_pct"
  VDHP_ResetPedalZeroPosStart_flg/1 -> VDHP_ResetPedalZeroPosStart_flg_Inproc/1  "VDHP_ResetPedalZeroPosStart_flg"
  VDHP_ResetPedalZeroPosStart_flg_Inproc/1 -> UnitConverter399/1
  UnitConverter399/1 -> VOUTP_ResetPedalZeroPosStart_flg/1  "VOUTP_ResetPedalZeroPosStart_flg"
  VDHP_EAPS1NRM_pct/1 -> VDHP_EAPS1NRM_pct_Inproc/1  "VDHP_EAPS1NRM_pct"
  VDHP_EAPS1NRM_pct_Inproc/1 -> UnitConverter400/1
  UnitConverter400/1 -> VOUTP_EAPS1NRM_pct/1  "VOUTP_EAPS1NRM_pct"
  VDHP_EAPS2NRM_pct/1 -> VDHP_EAPS2NRM_pct_Inproc/1  "VDHP_EAPS2NRM_pct"
  VDHP_EAPS2NRM_pct_Inproc/1 -> UnitConverter401/1
  UnitConverter401/1 -> VOUTP_EAPS2NRM_pct/1  "VOUTP_EAPS2NRM_pct"
  VDID_VSS_kph/1 -> VDID_VSS_kph_Inproc/1  "VDID_VSS_kph"
  VDID_VSS_kph_Inproc/1 -> UnitConverter402/1
  UnitConverter402/1 -> VOUTP_VSS_kph/1  "VOUTP_VSS_kph"
  VDID_RUNTM_s/1 -> VDID_RUNTM_s_Inproc/1  "VDID_RUNTM_s"
  VDID_RUNTM_s_Inproc/1 -> UnitConverter403/1
  UnitConverter403/1 -> VOUTP_RUNTM_s/1  "VOUTP_RUNTM_s"
  VDID_MILDIST_km/1 -> VDID_MILDIST_km_Inproc/1  "VDID_MILDIST_km"
  VDID_MILDIST_km_Inproc/1 -> UnitConverter404/1
  UnitConverter404/1 -> VOUTP_MILDIST_km/1  "VOUTP_MILDIST_km"
  VDID_WARMUPS_cnt/1 -> VDID_WARMUPS_cnt_Inproc/1  "VDID_WARMUPS_cnt"
  VDID_WARMUPS_cnt_Inproc/1 -> UnitConverter405/1
  UnitConverter405/1 -> VOUTP_WARMUPS_cnt/1  "VOUTP_WARMUPS_cnt"
  VDID_CLRDIST_km/1 -> VDID_CLRDIST_km_Inproc/1  "VDID_CLRDIST_km"
  VDID_CLRDIST_km_Inproc/1 -> UnitConverter406/1
  UnitConverter406/1 -> VOUTP_CLRDIST_km/1  "VOUTP_CLRDIST_km"
  VDID_APPD_pct/1 -> VDID_APPD_pct_Inproc/1  "VDID_APPD_pct"
  VDID_APPD_pct_Inproc/1 -> UnitConverter407/1
  UnitConverter407/1 -> VOUTP_APPD_pct/1  "VOUTP_APPD_pct"
  VDID_APPE_pct/1 -> VDID_APPE_pct_Inproc/1  "VDID_APPE_pct"
  VDID_APPE_pct_Inproc/1 -> UnitConverter408/1
  UnitConverter408/1 -> VOUTP_APPE_pct/1  "VOUTP_APPE_pct"
  VDID_MILTIME_min/1 -> VDID_MILTIME_min_Inproc/1  "VDID_MILTIME_min"
  VDID_MILTIME_min_Inproc/1 -> UnitConverter409/1
  UnitConverter409/1 -> VOUTP_MILTIME_min/1  "VOUTP_MILTIME_min"
  VDID_CLRTIME_min/1 -> VDID_CLRTIME_min_Inproc/1  "VDID_CLRTIME_min"
  VDID_CLRTIME_min_Inproc/1 -> UnitConverter410/1
  UnitConverter410/1 -> VOUTP_CLRTIME_min/1  "VOUTP_CLRTIME_min"
  VDID_BATSOC_pct/1 -> VDID_BATSOC_pct_Inproc/1  "VDID_BATSOC_pct"
  VDID_BATSOC_pct_Inproc/1 -> UnitConverter411/1
  UnitConverter411/1 -> VOUTP_BATSOC_pct/1  "VOUTP_BATSOC_pct"
  VDID_HEVBATT_V/1 -> VDID_HEVBATT_V_Inproc/1  "VDID_HEVBATT_V"
  VDID_HEVBATT_V_Inproc/1 -> UnitConverter412/1
  UnitConverter412/1 -> VOUTP_HEVBATT_V/1  "VOUTP_HEVBATT_V"
  VDID_ODOMETER_km/1 -> VDID_ODOMETER_km_Inproc/1  "VDID_ODOMETER_km"
  VDID_ODOMETER_km_Inproc/1 -> UnitConverter413/1
  UnitConverter413/1 -> VOUTP_ODOMETER_km/1  "VOUTP_ODOMETER_km"
  VDID_BATSOH_pct/1 -> VDID_BATSOH_pct_Inproc/1  "VDID_BATSOH_pct"
  VDID_BATSOH_pct_Inproc/1 -> UnitConverter414/1
  UnitConverter414/1 -> VOUTP_BATSOH_pct/1  "VOUTP_BATSOH_pct"
  VDID_HVBCellVoltMin_V/1 -> VDID_HVBCellVoltMin_V_Inproc/1  "VDID_HVBCellVoltMin_V"
  VDID_HVBCellVoltMin_V_Inproc/1 -> UnitConverter415/1
  UnitConverter415/1 -> VOUTP_HVBCellVoltMin_V/1  "VOUTP_HVBCellVoltMin_V"
  VDID_HVBCellVoltMax_V/1 -> VDID_HVBCellVoltMax_V_Inproc/1  "VDID_HVBCellVoltMax_V"
  VDID_HVBCellVoltMax_V_Inproc/1 -> UnitConverter416/1
  UnitConverter416/1 -> VOUTP_HVBCellVoltMax_V/1  "VOUTP_HVBCellVoltMax_V"
  VDID_HVESSCHARGELIM_kW/1 -> VDID_HVESSCHARGELIM_kW_Inproc/1  "VDID_HVESSCHARGELIM_kW"
  VDID_HVESSCHARGELIM_kW_Inproc/1 -> UnitConverter417/1
  UnitConverter417/1 -> VOUTP_HVESSCHARGELIM_kW/1  "VOUTP_HVESSCHARGELIM_kW"
  VDID_HVESSCHARGEACT_kW/1 -> VDID_HVESSCHARGEACT_kW_Inproc/1  "VDID_HVESSCHARGEACT_kW"
  VDID_HVESSCHARGEACT_kW_Inproc/1 -> UnitConverter418/1
  UnitConverter418/1 -> VOUTP_HVESSCHARGEACT_kW/1  "VOUTP_HVESSCHARGEACT_kW"
  VDID_HVESSENER_Whps/1 -> VDID_HVESSENER_Whps_Inproc/1  "VDID_HVESSENER_Whps"
  VDID_HVESSENER_Whps_Inproc/1 -> UnitConverter419/1
  UnitConverter419/1 -> VOUTP_HVESSENER_Whps/1  "VOUTP_HVESSENER_Whps"
  VDID_NUMPSATRIPSFLTMEMCLR_cnt/1 -> VDID_NUMPSATRIPSFLTMEMCLR_cnt_Inproc/1  "VDID_NUMPSATRIPSFLTMEMCLR_cnt"
  VDID_NUMPSATRIPSFLTMEMCLR_cnt_Inproc/1 -> UnitConverter420/1
  UnitConverter420/1 -> VOUTP_NUMPSATRIPSFLTMEMCLR_cnt/1  "VOUTP_NUMPSATRIPSFLTMEMCLR_cnt"
  VDID_HVBattCurr_Ahps/1 -> VDID_HVBattCurr_Ahps_Inproc/1  "VDID_HVBattCurr_Ahps"
  VDID_HVBattCurr_Ahps_Inproc/1 -> UnitConverter421/1
  UnitConverter421/1 -> VOUTP_HVBattCurr_Ahps/1  "VOUTP_HVBattCurr_Ahps"
  VDID_PSAR_sec/1 -> VDID_PSAR_sec_Inproc/1  "VDID_PSAR_sec"
  VDID_PSAR_sec_Inproc/1 -> UnitConverter422/1
  UnitConverter422/1 -> VOUTP_PSAR_sec/1  "VOUTP_PSAR_sec"
  VDID_PSAL_sec/1 -> VDID_PSAL_sec_Inproc/1  "VDID_PSAL_sec"
  VDID_PSAL_sec_Inproc/1 -> UnitConverter423/1
  UnitConverter423/1 -> VOUTP_PSAL_sec/1  "VOUTP_PSAL_sec"
  VDID_IPSAR_sec/1 -> VDID_IPSAR_sec_Inproc/1  "VDID_IPSAR_sec"
  VDID_IPSAR_sec_Inproc/1 -> UnitConverter424/1
  UnitConverter424/1 -> VOUTP_IPSAR_sec/1  "VOUTP_IPSAR_sec"
  VDID_IPSAL_sec/1 -> VDID_IPSAL_sec_Inproc/1  "VDID_IPSAL_sec"
  VDID_IPSAL_sec_Inproc/1 -> UnitConverter425/1
  UnitConverter425/1 -> VOUTP_IPSAL_sec/1  "VOUTP_IPSAL_sec"
  VDID_CPSAR_sec/1 -> VDID_CPSAR_sec_Inproc/1  "VDID_CPSAR_sec"
  VDID_CPSAR_sec_Inproc/1 -> UnitConverter426/1
  UnitConverter426/1 -> VOUTP_CPSAR_sec/1  "VOUTP_CPSAR_sec"
  VDID_CPSAL_sec/1 -> VDID_CPSAL_sec_Inproc/1  "VDID_CPSAL_sec"
  VDID_CPSAL_sec_Inproc/1 -> UnitConverter427/1
  UnitConverter427/1 -> VOUTP_CPSAL_sec/1  "VOUTP_CPSAL_sec"
  VDID_HVBNAH_Ahr/1 -> VDID_HVBNAH_Ahr_Inproc/1  "VDID_HVBNAH_Ahr"
  VDID_HVBNAH_Ahr_Inproc/1 -> UnitConverter428/1
  UnitConverter428/1 -> VOUTP_HVBNAH_Ahr/1  "VOUTP_HVBNAH_Ahr"
  VDID_HVBNE_kWh/1 -> VDID_HVBNE_kWh_Inproc/1  "VDID_HVBNE_kWh"
  VDID_HVBNE_kWh_Inproc/1 -> UnitConverter429/1
  UnitConverter429/1 -> VOUTP_HVBNE_kWh/1  "VOUTP_HVBNE_kWh"
  VDID_IGNCNTR_cnt/1 -> VDID_IGNCNTR_cnt_Inproc/1  "VDID_IGNCNTR_cnt"
  VDID_IGNCNTR_cnt_Inproc/1 -> UnitConverter430/1
  UnitConverter430/1 -> VOUTP_IGNCNTR_cnt/1  "VOUTP_IGNCNTR_cnt"
  VDID_TNBCPSAR_Ahr/1 -> VDID_TNBCPSAR_Ahr_Inproc/1  "VDID_TNBCPSAR_Ahr"
  VDID_TNBCPSAR_Ahr_Inproc/1 -> UnitConverter431/1
  UnitConverter431/1 -> VOUTP_TNBCPSAR_Ahr/1  "VOUTP_TNBCPSAR_Ahr"
  VDID_TNBCPSAL_Ahr/1 -> VDID_TNBCPSAL_Ahr_Inproc/1  "VDID_TNBCPSAL_Ahr"
  VDID_TNBCPSAL_Ahr_Inproc/1 -> UnitConverter432/1
  UnitConverter432/1 -> VOUTP_TNBCPSAL_Ahr/1  "VOUTP_TNBCPSAL_Ahr"
  VDID_TNECPSAR_kWh/1 -> VDID_TNECPSAR_kWh_Inproc/1  "VDID_TNECPSAR_kWh"
  VDID_TNECPSAR_kWh_Inproc/1 -> UnitConverter433/1
  UnitConverter433/1 -> VOUTP_TNECPSAR_kWh/1  "VOUTP_TNECPSAR_kWh"
  VDID_TNECPSAL_kWh/1 -> VDID_TNECPSAL_kWh_Inproc/1  "VDID_TNECPSAL_kWh"
  VDID_TNECPSAL_kWh_Inproc/1 -> UnitConverter434/1
  UnitConverter434/1 -> VOUTP_TNECPSAL_kWh/1  "VOUTP_TNECPSAL_kWh"
  VDID_TEBPSAR_kWh/1 -> VDID_TEBPSAR_kWh_Inproc/1  "VDID_TEBPSAR_kWh"
  VDID_TEBPSAR_kWh_Inproc/1 -> UnitConverter435/1
  UnitConverter435/1 -> VOUTP_TEBPSAR_kWh/1  "VOUTP_TEBPSAR_kWh"
  VDID_TEBPSAL_kWh/1 -> VDID_TEBPSAL_kWh_Inproc/1  "VDID_TEBPSAL_kWh"
  VDID_TEBPSAL_kWh_Inproc/1 -> UnitConverter436/1
  UnitConverter436/1 -> VOUTP_TEBPSAL_kWh/1  "VOUTP_TEBPSAL_kWh"
  VDID_TGEOVCR_kWh/1 -> VDID_TGEOVCR_kWh_Inproc/1  "VDID_TGEOVCR_kWh"
  VDID_TGEOVCR_kWh_Inproc/1 -> UnitConverter437/1
  UnitConverter437/1 -> VOUTP_TGEOVCR_kWh/1  "VOUTP_TGEOVCR_kWh"
  VDID_TGEOVCL_kWh/1 -> VDID_TGEOVCL_kWh_Inproc/1  "VDID_TGEOVCL_kWh"
  VDID_TGEOVCL_kWh_Inproc/1 -> UnitConverter438/1
  UnitConverter438/1 -> VOUTP_TGEOVCL_kWh/1  "VOUTP_TGEOVCL_kWh"
  VDID_GECHGOVCDCR_kWh/1 -> VDID_GECHGOVCDCR_kWh_Inproc/1  "VDID_GECHGOVCDCR_kWh"
  VDID_GECHGOVCDCR_kWh_Inproc/1 -> UnitConverter439/1
  UnitConverter439/1 -> VOUTP_GECHGOVCDCR_kWh/1  "VOUTP_GECHGOVCDCR_kWh"
  VDID_GECHGOVCDCL_kWh/1 -> VDID_GECHGOVCDCL_kWh_Inproc/1  "VDID_GECHGOVCDCL_kWh"
  VDID_GECHGOVCDCL_kWh_Inproc/1 -> UnitConverter440/1
  UnitConverter440/1 -> VOUTP_GECHGOVCDCL_kWh/1  "VOUTP_GECHGOVCDCL_kWh"
  VDID_GECHGOVCACR_kWh/1 -> VDID_GECHGOVCACR_kWh_Inproc/1  "VDID_GECHGOVCACR_kWh"
  VDID_GECHGOVCACR_kWh_Inproc/1 -> UnitConverter441/1
  UnitConverter441/1 -> VOUTP_GECHGOVCACR_kWh/1  "VOUTP_GECHGOVCACR_kWh"
  VDID_GECHGOVCACL_kWh/1 -> VDID_GECHGOVCACL_kWh_Inproc/1  "VDID_GECHGOVCACL_kWh"
  VDID_GECHGOVCACL_kWh_Inproc/1 -> UnitConverter442/1
  UnitConverter442/1 -> VOUTP_GECHGOVCACL_kWh/1  "VOUTP_GECHGOVCACL_kWh"
  VDID_RESSV2XENNONPSAR_kWh/1 -> VDID_RESSV2XENNONPSAR_kWh_Inproc/1  "VDID_RESSV2XENNONPSAR_kWh"
  VDID_RESSV2XENNONPSAR_kWh_Inproc/1 -> UnitConverter443/1
  UnitConverter443/1 -> VOUTP_RESSV2XENNONPSAR_kWh/1  "VOUTP_RESSV2XENNONPSAR_kWh"
  VDID_RESSV2XENNONPSAL_kWh/1 -> VDID_RESSV2XENNONPSAL_kWh_Inproc/1  "VDID_RESSV2XENNONPSAL_kWh"
  VDID_RESSV2XENNONPSAL_kWh_Inproc/1 -> UnitConverter444/1
  UnitConverter444/1 -> VOUTP_RESSV2XENNONPSAL_kWh/1  "VOUTP_RESSV2XENNONPSAL_kWh"
  VDID_PKER_kphsqr/1 -> VDID_PKER_kphsqr_Inproc/1  "VDID_PKER_kphsqr"
  VDID_PKER_kphsqr_Inproc/1 -> UnitConverter445/1
  UnitConverter445/1 -> VOUTP_PKER_kphsqr/1  "VOUTP_PKER_kphsqr"
  VDID_PKEL_kphsqr/1 -> VDID_PKEL_kphsqr_Inproc/1  "VDID_PKEL_kphsqr"
  VDID_PKEL_kphsqr_Inproc/1 -> UnitConverter446/1
  UnitConverter446/1 -> VOUTP_PKEL_kphsqr/1  "VOUTP_PKEL_kphsqr"
  VDID_ResetCDEODTR_km/1 -> VDID_ResetCDEODTR_km_Inproc/1  "VDID_ResetCDEODTR_km"
  VDID_ResetCDEODTR_km_Inproc/1 -> UnitConverter447/1
  UnitConverter447/1 -> VOUTP_ResetCDEODTR_km/1  "VOUTP_ResetCDEODTR_km"
  VDID_CDEODTR_km/1 -> VDID_CDEODTR_km_Inproc/1  "VDID_CDEODTR_km"
  VDID_CDEODTR_km_Inproc/1 -> UnitConverter448/1
  UnitConverter448/1 -> VOUTP_CDEODTR_km/1  "VOUTP_CDEODTR_km"
  VDID_CDEODTL_km/1 -> VDID_CDEODTL_km_Inproc/1  "VDID_CDEODTL_km"
  VDID_CDEODTL_km_Inproc/1 -> UnitConverter449/1
  UnitConverter449/1 -> VOUTP_CDEODTL_km/1  "VOUTP_CDEODTL_km"
  VDID_AvgBattTempPSAR_C/1 -> VDID_AvgBattTempPSAR_C_Inproc/1  "VDID_AvgBattTempPSAR_C"
  VDID_AvgBattTempPSAR_C_Inproc/1 -> UnitConverter450/1
  UnitConverter450/1 -> VOUTP_AvgBattTempPSAR_C/1  "VOUTP_AvgBattTempPSAR_C"
  VDID_AvgBattTempPSAL_C/1 -> VDID_AvgBattTempPSAL_C_Inproc/1  "VDID_AvgBattTempPSAL_C"
  VDID_AvgBattTempPSAL_C_Inproc/1 -> UnitConverter451/1
  UnitConverter451/1 -> VOUTP_AvgBattTempPSAL_C/1  "VOUTP_AvgBattTempPSAL_C"
  VDID_AvgBattTempOVCR_C/1 -> VDID_AvgBattTempOVCR_C_Inproc/1  "VDID_AvgBattTempOVCR_C"
  VDID_AvgBattTempOVCR_C_Inproc/1 -> UnitConverter452/1
  UnitConverter452/1 -> VOUTP_AvgBattTempOVCR_C/1  "VOUTP_AvgBattTempOVCR_C"
  VDID_AvgBattTempOVCL_C/1 -> VDID_AvgBattTempOVCL_C_Inproc/1  "VDID_AvgBattTempOVCL_C"
  VDID_AvgBattTempOVCL_C_Inproc/1 -> UnitConverter453/1
  UnitConverter453/1 -> VOUTP_AvgBattTempOVCL_C/1  "VOUTP_AvgBattTempOVCL_C"
  VDID_AvgBattTempOFFR_C/1 -> VDID_AvgBattTempOFFR_C_Inproc/1  "VDID_AvgBattTempOFFR_C"
  VDID_AvgBattTempOFFR_C_Inproc/1 -> UnitConverter454/1
  UnitConverter454/1 -> VOUTP_AvgBattTempOFFR_C/1  "VOUTP_AvgBattTempOFFR_C"
  VDID_AvgBattTempOFFL_C/1 -> VDID_AvgBattTempOFFL_C_Inproc/1  "VDID_AvgBattTempOFFL_C"
  VDID_AvgBattTempOFFL_C_Inproc/1 -> UnitConverter455/1
  UnitConverter455/1 -> VOUTP_AvgBattTempOFFL_C/1  "VOUTP_AvgBattTempOFFL_C"
  VDID_QTYPSATRIPSR_cnt/1 -> VDID_QTYPSATRIPSR_cnt_Inproc/1  "VDID_QTYPSATRIPSR_cnt"
  VDID_QTYPSATRIPSR_cnt_Inproc/1 -> UnitConverter456/1
  UnitConverter456/1 -> VOUTP_QTYPSATRIPSR_cnt/1  "VOUTP_QTYPSATRIPSR_cnt"
  VDID_QTYPSATRIPSL_cnt/1 -> VDID_QTYPSATRIPSL_cnt_Inproc/1  "VDID_QTYPSATRIPSL_cnt"
  VDID_QTYPSATRIPSL_cnt_Inproc/1 -> UnitConverter457/1
  UnitConverter457/1 -> VOUTP_QTYPSATRIPSL_cnt/1  "VOUTP_QTYPSATRIPSL_cnt"
  VDID_RESSCNTDODRNGR_cnt/1 -> VDID_RESSCNTDODRNGR_cnt_Inproc/1  "VDID_RESSCNTDODRNGR_cnt"
  VDID_RESSCNTDODRNGR_cnt_Inproc/1 -> UnitConverter458/1
  UnitConverter458/1 -> VOUTP_RESSCNTDODRNGR_cnt/1  "VOUTP_RESSCNTDODRNGR_cnt"
  VDID_RESSCNTDODRNGL_cnt/1 -> VDID_RESSCNTDODRNGL_cnt_Inproc/1  "VDID_RESSCNTDODRNGL_cnt"
  VDID_RESSCNTDODRNGL_cnt_Inproc/1 -> UnitConverter459/1
  UnitConverter459/1 -> VOUTP_RESSCNTDODRNGL_cnt/1  "VOUTP_RESSCNTDODRNGL_cnt"
  VDID_ETMATOER_kWh/1 -> VDID_ETMATOER_kWh_Inproc/1  "VDID_ETMATOER_kWh"
  VDID_ETMATOER_kWh_Inproc/1 -> UnitConverter460/1
  UnitConverter460/1 -> VOUTP_ETMATOER_kWh/1  "VOUTP_ETMATOER_kWh"
  VDID_ETMATOEL_kWh/1 -> VDID_ETMATOEL_kWh_Inproc/1  "VDID_ETMATOEL_kWh"
  VDID_ETMATOEL_kWh_Inproc/1 -> UnitConverter461/1
  UnitConverter461/1 -> VOUTP_ETMATOEL_kWh/1  "VOUTP_ETMATOEL_kWh"
  VDID_ETMBTOER_kWh/1 -> VDID_ETMBTOER_kWh_Inproc/1  "VDID_ETMBTOER_kWh"
  VDID_ETMBTOER_kWh_Inproc/1 -> UnitConverter462/1
  UnitConverter462/1 -> VOUTP_ETMBTOER_kWh/1  "VOUTP_ETMBTOER_kWh"
  VDID_ETMBTOEL_kWh/1 -> VDID_ETMBTOEL_kWh_Inproc/1  "VDID_ETMBTOEL_kWh"
  VDID_ETMBTOEL_kWh_Inproc/1 -> UnitConverter463/1
  UnitConverter463/1 -> VOUTP_ETMBTOEL_kWh/1  "VOUTP_ETMBTOEL_kWh"
  VDID_RESSTIMESOCPSARNGR_s/1 -> VDID_RESSTIMESOCPSARNGR_s_Inproc/1  "VDID_RESSTIMESOCPSARNGR_s"
  VDID_RESSTIMESOCPSARNGR_s_Inproc/1 -> UnitConverter464/1
  UnitConverter464/1 -> VOUTP_RESSTIMESOCPSARNGR_s/1  "VOUTP_RESSTIMESOCPSARNGR_s"
  VDID_RESSTIMESOCPSARNGL_s/1 -> VDID_RESSTIMESOCPSARNGL_s_Inproc/1  "VDID_RESSTIMESOCPSARNGL_s"
  VDID_RESSTIMESOCPSARNGL_s_Inproc/1 -> UnitConverter465/1
  UnitConverter465/1 -> VOUTP_RESSTIMESOCPSARNGL_s/1  "VOUTP_RESSTIMESOCPSARNGL_s"
  VDID_RESSTIMESOCCHGRNGR_s/1 -> VDID_RESSTIMESOCCHGRNGR_s_Inproc/1  "VDID_RESSTIMESOCCHGRNGR_s"
  VDID_RESSTIMESOCCHGRNGR_s_Inproc/1 -> UnitConverter466/1
  UnitConverter466/1 -> VOUTP_RESSTIMESOCCHGRNGR_s/1  "VOUTP_RESSTIMESOCCHGRNGR_s"
  VDID_RESSTIMESOCCHGRNGL_s/1 -> VDID_RESSTIMESOCCHGRNGL_s_Inproc/1  "VDID_RESSTIMESOCCHGRNGL_s"
  VDID_RESSTIMESOCCHGRNGL_s_Inproc/1 -> UnitConverter467/1
  UnitConverter467/1 -> VOUTP_RESSTIMESOCCHGRNGL_s/1  "VOUTP_RESSTIMESOCCHGRNGL_s"
  VDID_RESSTIMESOCOFFRNGR_s/1 -> VDID_RESSTIMESOCOFFRNGR_s_Inproc/1  "VDID_RESSTIMESOCOFFRNGR_s"
  VDID_RESSTIMESOCOFFRNGR_s_Inproc/1 -> UnitConverter468/1
  UnitConverter468/1 -> VOUTP_RESSTIMESOCOFFRNGR_s/1  "VOUTP_RESSTIMESOCOFFRNGR_s"
  VDID_RESSTIMESOCOFFRNGL_s/1 -> VDID_RESSTIMESOCOFFRNGL_s_Inproc/1  "VDID_RESSTIMESOCOFFRNGL_s"
  VDID_RESSTIMESOCOFFRNGL_s_Inproc/1 -> UnitConverter469/1
  UnitConverter469/1 -> VOUTP_RESSTIMESOCOFFRNGL_s/1  "VOUTP_RESSTIMESOCOFFRNGL_s"
  VDID_MAXBATTEMPL_C/1 -> VDID_MAXBATTEMPL_C_Inproc/1  "VDID_MAXBATTEMPL_C"
  VDID_MAXBATTEMPL_C_Inproc/1 -> UnitConverter470/1
  UnitConverter470/1 -> VOUTP_MAXBATTEMPL_C/1  "VOUTP_MAXBATTEMPL_C"
  VDID_MINBATTEMPL_C/1 -> VDID_MINBATTEMPL_C_Inproc/1  "VDID_MINBATTEMPL_C"
  VDID_MINBATTEMPL_C_Inproc/1 -> UnitConverter471/1
  UnitConverter471/1 -> VOUTP_MINBATTEMPL_C/1  "VOUTP_MINBATTEMPL_C"
  VDID_AVGBATTEMPL_C/1 -> VDID_AVGBATTEMPL_C_Inproc/1  "VDID_AVGBATTEMPL_C"
  VDID_AVGBATTEMPL_C_Inproc/1 -> UnitConverter472/1
  UnitConverter472/1 -> VOUTP_AVGBATTEMPL_C/1  "VOUTP_AVGBATTEMPL_C"
  VDID_PROTOCOLID_enum/1 -> VDID_PROTOCOLID_enum_Inproc/1  "VDID_PROTOCOLID_enum"
  VDID_PROTOCOLID_enum_Inproc/1 -> UnitConverter473/1
  UnitConverter473/1 -> VOUTP_PROTOCOLID_enum/1  "VOUTP_PROTOCOLID_enum"
  VDID_RESSTTEMPRNGAXIS_enum/1 -> VDID_RESSTTEMPRNGAXIS_enum_Inproc/1  "VDID_RESSTTEMPRNGAXIS_enum"
  VDID_RESSTTEMPRNGAXIS_enum_Inproc/1 -> UnitConverter474/1
  UnitConverter474/1 -> VOUTP_RESSTTEMPRNGAXIS_enum/1  "VOUTP_RESSTTEMPRNGAXIS_enum"
  VDID_RESSTIMESOCRNGAXIS_enum/1 -> VDID_RESSTIMESOCRNGAXIS_enum_Inproc/1  "VDID_RESSTIMESOCRNGAXIS_enum"
  VDID_RESSTIMESOCRNGAXIS_enum_Inproc/1 -> UnitConverter475/1
  UnitConverter475/1 -> VOUTP_RESSTIMESOCRNGAXIS_enum/1  "VOUTP_RESSTIMESOCRNGAXIS_enum"
  VDID_RESSCNTSDODRNGAXIS_enum/1 -> VDID_RESSCNTSDODRNGAXIS_enum_Inproc/1  "VDID_RESSCNTSDODRNGAXIS_enum"
  VDID_RESSCNTSDODRNGAXIS_enum_Inproc/1 -> UnitConverter476/1
  UnitConverter476/1 -> VOUTP_RESSCNTSDODRNGAXIS_enum/1  "VOUTP_RESSCNTSDODRNGAXIS_enum"
  VDID_CALID_cnt/1 -> VDID_CALID_cnt_Inproc/1  "VDID_CALID_cnt"
  VDID_CALID_cnt_Inproc/1 -> UnitConverter477/1
  UnitConverter477/1 -> VOUTP_CALID_cnt/1  "VOUTP_CALID_cnt"
  VDID_ECUNAME_cnt/1 -> VDID_ECUNAME_cnt_Inproc/1  "VDID_ECUNAME_cnt"
  VDID_ECUNAME_cnt_Inproc/1 -> UnitConverter478/1
  UnitConverter478/1 -> VOUTP_ECUNAME_cnt/1  "VOUTP_ECUNAME_cnt"
  VDID_PKERNumerator_kphsqr/1 -> VDID_PKERNumerator_kphsqr_Inproc/1  "VDID_PKERNumerator_kphsqr"
  VDID_PKERNumerator_kphsqr_Inproc/1 -> UnitConverter479/1
  UnitConverter479/1 -> VOUTP_PKERNumerator_kphsqr/1  "VOUTP_PKERNumerator_kphsqr"
  VDID_PKELNumerator_kphsqr/1 -> VDID_PKELNumerator_kphsqr_Inproc/1  "VDID_PKELNumerator_kphsqr"
  VDID_PKELNumerator_kphsqr_Inproc/1 -> UnitConverter480/1
  UnitConverter480/1 -> VOUTP_PKELNumerator_kphsqr/1  "VOUTP_PKELNumerator_kphsqr"
  VDID_BattTempPSAR_sec/1 -> VDID_BattTempPSAR_sec_Inproc/1  "VDID_BattTempPSAR_sec"
  VDID_BattTempPSAR_sec_Inproc/1 -> UnitConverter481/1
  UnitConverter481/1 -> VOUTP_BattTempPSAR_sec/1  "VOUTP_BattTempPSAR_sec"
  VDID_BattTempPSAL_sec/1 -> VDID_BattTempPSAL_sec_Inproc/1  "VDID_BattTempPSAL_sec"
  VDID_BattTempPSAL_sec_Inproc/1 -> UnitConverter482/1
  UnitConverter482/1 -> VOUTP_BattTempPSAL_sec/1  "VOUTP_BattTempPSAL_sec"
  VDID_OVCR_sec/1 -> VDID_OVCR_sec_Inproc/1  "VDID_OVCR_sec"
  VDID_OVCR_sec_Inproc/1 -> UnitConverter483/1
  UnitConverter483/1 -> VOUTP_OVCR_sec/1  "VOUTP_OVCR_sec"
  VDID_OVCL_sec/1 -> VDID_OVCL_sec_Inproc/1  "VDID_OVCL_sec"
  VDID_OVCL_sec_Inproc/1 -> UnitConverter484/1
  UnitConverter484/1 -> VOUTP_OVCL_sec/1  "VOUTP_OVCL_sec"
  VDID_OFFR_sec/1 -> VDID_OFFR_sec_Inproc/1  "VDID_OFFR_sec"
  VDID_OFFR_sec_Inproc/1 -> UnitConverter485/1
  UnitConverter485/1 -> VOUTP_OFFR_sec/1  "VOUTP_OFFR_sec"
  VDID_OFFL_sec/1 -> VDID_OFFL_sec_Inproc/1  "VDID_OFFL_sec"
  VDID_OFFL_sec_Inproc/1 -> UnitConverter486/1
  UnitConverter486/1 -> VOUTP_OFFL_sec/1  "VOUTP_OFFL_sec"
  VDID_AVGBATTEMPL_sec/1 -> VDID_AVGBATTEMPL_sec_Inproc/1  "VDID_AVGBATTEMPL_sec"
  VDID_AVGBATTEMPL_sec_Inproc/1 -> UnitConverter487/1
  UnitConverter487/1 -> VOUTP_AVGBATTEMPL_sec/1  "VOUTP_AVGBATTEMPL_sec"
  VDID_VinCode_cnt/1 -> VDID_VinCode_cnt_Inproc/1  "VDID_VinCode_cnt"
  VDID_VinCode_cnt_Inproc/1 -> UnitConverter488/1
  UnitConverter488/1 -> VOUTP_VinCode_cnt/1  "VOUTP_VinCode_cnt"
  VDID_STASUP_enum/1 -> VDID_STASUP_enum_Inproc/1  "VDID_STASUP_enum"
  VDID_STASUP_enum_Inproc/1 -> UnitConverter489/1
  UnitConverter489/1 -> VOUTP_STASUP_enum/1  "VOUTP_STASUP_enum"
  VDID_HEVMODE_enum/1 -> VDID_HEVMODE_enum_Inproc/1  "VDID_HEVMODE_enum"
  VDID_HEVMODE_enum_Inproc/1 -> UnitConverter490/1
  UnitConverter490/1 -> VOUTP_HEVMODE_enum/1  "VOUTP_HEVMODE_enum"
  VDID_HVBATT_A/1 -> VDID_HVBATT_A_Inproc/1  "VDID_HVBATT_A"
  VDID_HVBATT_A_Inproc/1 -> UnitConverter491/1
  UnitConverter491/1 -> VOUTP_HVBATT_A/1  "VOUTP_HVBATT_A"
  VDID_DIDModelVersion_raw/1 -> VDID_DIDModelVersion_raw_Inproc/1  "VDID_DIDModelVersion_raw"
  VDID_DIDModelVersion_raw_Inproc/1 -> UnitConverter492/1
  UnitConverter492/1 -> VOUTP_DIDModelVersion_raw/1  "VOUTP_DIDModelVersion_raw"
  VDID_DIDModelVersionChksum_raw/1 -> VDID_DIDModelVersionChksum_raw_Inproc/1  "VDID_DIDModelVersionChksum_raw"
  VDID_DIDModelVersionChksum_raw_Inproc/1 -> UnitConverter493/1
  UnitConverter493/1 -> VOUTP_DIDModelVersionChksum_raw/1  "VOUTP_DIDModelVersionChksum_raw"
  VDKC_DKCTimeSN_cnt/1 -> VDKC_DKCTimeSN_cnt_Inproc/1  "VDKC_DKCTimeSN_cnt"
  VDKC_DKCTimeSN_cnt_Inproc/1 -> UnitConverter494/1
  UnitConverter494/1 -> VOUTP_DKCTimeSN_cnt/1  "VOUTP_DKCTimeSN_cnt"
  VDKC_DKCAuthSta_enum/1 -> VDKC_DKCAuthSta_enum_Inproc/1  "VDKC_DKCAuthSta_enum"
  VDKC_DKCAuthSta_enum_Inproc/1 -> UnitConverter495/1
  UnitConverter495/1 -> VOUTP_DKCAuthSta_enum/1  "VOUTP_DKCAuthSta_enum"
  VDKC_TimeSNDKCFbk_cnt/1 -> VDKC_TimeSNDKCFbk_cnt_Inproc/1  "VDKC_TimeSNDKCFbk_cnt"
  VDKC_TimeSNDKCFbk_cnt_Inproc/1 -> UnitConverter496/1
  UnitConverter496/1 -> VOUTP_TimeSNDKCFbk_cnt/1  "VOUTP_TimeSNDKCFbk_cnt"
  VDKC_KeyMissSta_flg/1 -> VDKC_KeyMissSta_flg_Inproc/1  "VDKC_KeyMissSta_flg"
  VDKC_KeyMissSta_flg_Inproc/1 -> UnitConverter497/1
  UnitConverter497/1 -> VOUTP_KeyMissSta_flg/1  "VOUTP_KeyMissSta_flg"
  VDKC_KeyModeSta_enum/1 -> VDKC_KeyModeSta_enum_Inproc/1  "VDKC_KeyModeSta_enum"
  VDKC_KeyModeSta_enum_Inproc/1 -> UnitConverter498/1
  UnitConverter498/1 -> VOUTP_KeyModeSta_enum/1  "VOUTP_KeyModeSta_enum"
  VDKC_DkeyShowIVISta_enum/1 -> VDKC_DkeyShowIVISta_enum_Inproc/1  "VDKC_DkeyShowIVISta_enum"
  VDKC_DkeyShowIVISta_enum_Inproc/1 -> UnitConverter499/1
  UnitConverter499/1 -> VOUTP_DkeyShowIVISta_enum/1  "VOUTP_DkeyShowIVISta_enum"
  VDKC_KeyAreaPS_enum/1 -> VDKC_KeyAreaPS_enum_Inproc/1  "VDKC_KeyAreaPS_enum"
  VDKC_KeyAreaPS_enum_Inproc/1 -> UnitConverter500/1
  UnitConverter500/1 -> VOUTP_KeyAreaPS_enum/1  "VOUTP_KeyAreaPS_enum"
  VDKC_KeyAreaLockUnlock_enum/1 -> VDKC_KeyAreaLockUnlock_enum_Inproc/1  "VDKC_KeyAreaLockUnlock_enum"
  VDKC_KeyAreaLockUnlock_enum_Inproc/1 -> UnitConverter501/1
  UnitConverter501/1 -> VOUTP_KeyAreaLockUnlock_enum/1  "VOUTP_KeyAreaLockUnlock_enum"
  VDKC_PCommandToBCM_enum/1 -> VDKC_PCommandToBCM_enum_Inproc/1  "VDKC_PCommandToBCM_enum"
  VDKC_PCommandToBCM_enum_Inproc/1 -> UnitConverter502/1
  UnitConverter502/1 -> VOUTP_PCommandToBCM_enum/1  "VOUTP_PCommandToBCM_enum"
  VDKC_DKeyWelcomeSta_enum/1 -> VDKC_DKeyWelcomeSta_enum_Inproc/1  "VDKC_DKeyWelcomeSta_enum"
  VDKC_DKeyWelcomeSta_enum_Inproc/1 -> UnitConverter503/1
  UnitConverter503/1 -> VOUTP_DKeyWelcomeSta_enum/1  "VOUTP_DKeyWelcomeSta_enum"
  VDKC_KeyAreaPTG_enum/1 -> VDKC_KeyAreaPTG_enum_Inproc/1  "VDKC_KeyAreaPTG_enum"
  VDKC_KeyAreaPTG_enum_Inproc/1 -> UnitConverter504/1
  UnitConverter504/1 -> VOUTP_KeyAreaPTG_enum/1  "VOUTP_KeyAreaPTG_enum"
  VDKC_KeyAreaSPTGSta_enum/1 -> VDKC_KeyAreaSPTGSta_enum_Inproc/1  "VDKC_KeyAreaSPTGSta_enum"
  VDKC_KeyAreaSPTGSta_enum_Inproc/1 -> UnitConverter505/1
  UnitConverter505/1 -> VOUTP_KeyAreaSPTGSta_enum/1  "VOUTP_KeyAreaSPTGSta_enum"
  VDKC_UIDLowPowerSta_enum/1 -> VDKC_UIDLowPowerSta_enum_Inproc/1  "VDKC_UIDLowPowerSta_enum"
  VDKC_UIDLowPowerSta_enum_Inproc/1 -> UnitConverter506/1
  UnitConverter506/1 -> VOUTP_UIDLowPowerSta_enum/1  "VOUTP_UIDLowPowerSta_enum"
  VDKC_DkeyAreaRAPSSta_enum/1 -> VDKC_DkeyAreaRAPSSta_enum_Inproc/1  "VDKC_DkeyAreaRAPSSta_enum"
  VDKC_DkeyAreaRAPSSta_enum_Inproc/1 -> UnitConverter507/1
  UnitConverter507/1 -> VOUTP_DkeyAreaRAPSSta_enum/1  "VOUTP_DkeyAreaRAPSSta_enum"
  VDKC_ParkingModeCmd_enum/1 -> VDKC_ParkingModeCmd_enum_Inproc/1  "VDKC_ParkingModeCmd_enum"
  VDKC_ParkingModeCmd_enum_Inproc/1 -> UnitConverter508/1
  UnitConverter508/1 -> VOUTP_ParkingModeCmd_enum/1  "VOUTP_ParkingModeCmd_enum"
  VDKC_KeyNumSta_enum/1 -> VDKC_KeyNumSta_enum_Inproc/1  "VDKC_KeyNumSta_enum"
  VDKC_KeyNumSta_enum_Inproc/1 -> UnitConverter509/1
  UnitConverter509/1 -> VOUTP_KeyNumSta_enum/1  "VOUTP_KeyNumSta_enum"
  VDKC_KeyTypeSta_enum/1 -> VDKC_KeyTypeSta_enum_Inproc/1  "VDKC_KeyTypeSta_enum"
  VDKC_KeyTypeSta_enum_Inproc/1 -> UnitConverter510/1
  UnitConverter510/1 -> VOUTP_KeyTypeSta_enum/1  "VOUTP_KeyTypeSta_enum"
  VDKC_FDCDKCAllowSleep_flg/1 -> VDKC_FDCDKCAllowSleep_flg_Inproc/1  "VDKC_FDCDKCAllowSleep_flg"
  VDKC_FDCDKCAllowSleep_flg_Inproc/1 -> UnitConverter511/1
  UnitConverter511/1 -> VOUTP_FDCDKCAllowSleep_flg/1  "VOUTP_FDCDKCAllowSleep_flg"
  VDKC_JudgeKeepUnlockZone_flg/1 -> VDKC_JudgeKeepUnlockZone_flg_Inproc/1  "VDKC_JudgeKeepUnlockZone_flg"
  VDKC_JudgeKeepUnlockZone_flg_Inproc/1 -> UnitConverter512/1
  UnitConverter512/1 -> VOUTP_JudgeKeepUnlockZone_flg/1  "VOUTP_JudgeKeepUnlockZone_flg"
  VDSC_DISCTurn_flg/1 -> VDSC_DISCTurn_flg_Inproc/1  "VDSC_DISCTurn_flg"
  VDSC_DISCTurn_flg_Inproc/1 -> UnitConverter513/1
  UnitConverter513/1 -> VOUTP_DISCTurn_flg/1  "VOUTP_DISCTurn_flg"
  VDSC_DISCTargetSpd_kph/1 -> VDSC_DISCTargetSpd_kph_Inproc/1  "VDSC_DISCTargetSpd_kph"
  VDSC_DISCTargetSpd_kph_Inproc/1 -> UnitConverter514/1
  UnitConverter514/1 -> VOUTP_DISCTargetSpd_kph/1  "VOUTP_DISCTargetSpd_kph"
  VDSC_DISCSta_enum/1 -> VDSC_DISCSta_enum_Inproc/1  "VDSC_DISCSta_enum"
  VDSC_DISCSta_enum_Inproc/1 -> UnitConverter515/1
  UnitConverter515/1 -> VOUTP_DISCSta_enum/1  "VOUTP_DISCSta_enum"
  VDSC_DISCButtSta_flg/1 -> VDSC_DISCButtSta_flg_Inproc/1  "VDSC_DISCButtSta_flg"
  VDSC_DISCButtSta_flg_Inproc/1 -> UnitConverter516/1
  UnitConverter516/1 -> VOUTP_DISCButtSta_flg/1  "VOUTP_DISCButtSta_flg"
  VNMM_AllCANTxReq_flg/1 -> VNMM_AllCANTxReq_flg_Inproc/1  "VNMM_AllCANTxReq_flg"
  VNMM_AllCANTxReq_flg_Inproc/1 -> UnitConverter517/1
  UnitConverter517/1 -> VOUTP_AllCANTxReq_flg/1  "VOUTP_AllCANTxReq_flg"
  VNMM_NMmTxReq_flg/1 -> VNMM_NMmTxReq_flg_Inproc/1  "VNMM_NMmTxReq_flg"
  VNMM_NMmTxReq_flg_Inproc/1 -> UnitConverter518/1
  UnitConverter518/1 -> VOUTP_NMmTxReq_flg/1  "VOUTP_NMmTxReq_flg"
  VNMM_Awake_enum/1 -> VNMM_Awake_enum_Inproc/1  "VNMM_Awake_enum"
  VNMM_Awake_enum_Inproc/1 -> UnitConverter519/1
  UnitConverter519/1 -> VOUTP_Awake_enum/1  "VOUTP_Awake_enum"
  VNMM_CSB_flg/1 -> VNMM_CSB_flg_Inproc/1  "VNMM_CSB_flg"
  VNMM_CSB_flg_Inproc/1 -> UnitConverter520/1
  UnitConverter520/1 -> VOUTP_CSB_flg/1  "VOUTP_CSB_flg"
  VNMM_ErrorState_enum/1 -> VNMM_ErrorState_enum_Inproc/1  "VNMM_ErrorState_enum"
  VNMM_ErrorState_enum_Inproc/1 -> UnitConverter521/1
  UnitConverter521/1 -> VOUTP_ErrorState_enum/1  "VOUTP_ErrorState_enum"
  VNMM_NodeID_enum/1 -> VNMM_NodeID_enum_Inproc/1  "VNMM_NodeID_enum"
  VNMM_NodeID_enum_Inproc/1 -> UnitConverter522/1
  UnitConverter522/1 -> VOUTP_NodeID_enum/1  "VOUTP_NodeID_enum"
  VNMM_PNI_flg/1 -> VNMM_PNI_flg_Inproc/1  "VNMM_PNI_flg"
  VNMM_PNI_flg_Inproc/1 -> UnitConverter523/1
  UnitConverter523/1 -> VOUTP_PNI_flg/1  "VOUTP_PNI_flg"
  VNMM_RptMsgReq_flg/1 -> VNMM_RptMsgReq_flg_Inproc/1  "VNMM_RptMsgReq_flg"
  VNMM_RptMsgReq_flg_Inproc/1 -> UnitConverter524/1
  UnitConverter524/1 -> VOUTP_RptMsgReq_flg/1  "VOUTP_RptMsgReq_flg"
  VNMM_WakeUp_enum/1 -> VNMM_WakeUp_enum_Inproc/1  "VNMM_WakeUp_enum"
  VNMM_WakeUp_enum_Inproc/1 -> UnitConverter525/1
  UnitConverter525/1 -> VOUTP_WakeUp_enum/1  "VOUTP_WakeUp_enum"
  VNMM_ActiveWU_flg/1 -> VNMM_ActiveWU_flg_Inproc/1  "VNMM_ActiveWU_flg"
  VNMM_ActiveWU_flg_Inproc/1 -> UnitConverter526/1
  UnitConverter526/1 -> VOUTP_ActiveWU_flg/1  "VOUTP_ActiveWU_flg"
  VNMM_SysNMmSta_enum/1 -> VNMM_SysNMmSta_enum_Inproc/1  "VNMM_SysNMmSta_enum"
  VNMM_SysNMmSta_enum_Inproc/1 -> UnitConverter527/1
  UnitConverter527/1 -> VOUTP_SysNMmSta_enum/1  "VOUTP_SysNMmSta_enum"
  VNMM_NetworkReq_flg/1 -> VNMM_NetworkReq_flg_Inproc/1  "VNMM_NetworkReq_flg"
  VNMM_NetworkReq_flg_Inproc/1 -> UnitConverter528/1
  UnitConverter528/1 -> VOUTP_NetworkReq_flg/1  "VOUTP_NetworkReq_flg"
  VPMM_SysPowerMode_enum/1 -> VPMM_SysPowerMode_enum_Inproc/1  "VPMM_SysPowerMode_enum"
  VPMM_SysPowerMode_enum_Inproc/1 -> UnitConverter529/1
  UnitConverter529/1 -> VOUTP_SysPowerMode_enum/1  "VOUTP_SysPowerMode_enum"
  VPMM_PowerUpState_enum/1 -> VPMM_PowerUpState_enum_Inproc/1  "VPMM_PowerUpState_enum"
  VPMM_PowerUpState_enum_Inproc/1 -> UnitConverter530/1
  UnitConverter530/1 -> VOUTP_PowerUpState_enum/1  "VOUTP_PowerUpState_enum"
  VPMM_PowerDownState_enum/1 -> VPMM_PowerDownState_enum_Inproc/1  "VPMM_PowerDownState_enum"
  VPMM_PowerDownState_enum_Inproc/1 -> UnitConverter531/1
  UnitConverter531/1 -> VOUTP_PowerDownState_enum/1  "VOUTP_PowerDownState_enum"
  VPMM_ChrgState_enum/1 -> VPMM_ChrgState_enum_Inproc/1  "VPMM_ChrgState_enum"
  VPMM_ChrgState_enum_Inproc/1 -> UnitConverter532/1
  UnitConverter532/1 -> VOUTP_ChrgState_enum/1  "VOUTP_ChrgState_enum"
  VPMM_PowerUpFault_enum/1 -> VPMM_PowerUpFault_enum_Inproc/1  "VPMM_PowerUpFault_enum"
  VPMM_PowerUpFault_enum_Inproc/1 -> UnitConverter533/1
  UnitConverter533/1 -> VOUTP_PowerUpFault_enum/1  "VOUTP_PowerUpFault_enum"
  VPMM_PowerDownFault_enum/1 -> VPMM_PowerDownFault_enum_Inproc/1  "VPMM_PowerDownFault_enum"
  VPMM_PowerDownFault_enum_Inproc/1 -> UnitConverter534/1
  UnitConverter534/1 -> VOUTP_PowerDownFault_enum/1  "VOUTP_PowerDownFault_enum"
  VPMM_ChrgFault_enum/1 -> VPMM_ChrgFault_enum_Inproc/1  "VPMM_ChrgFault_enum"
  VPMM_ChrgFault_enum_Inproc/1 -> UnitConverter535/1
  UnitConverter535/1 -> VOUTP_ChrgFault_enum/1  "VOUTP_ChrgFault_enum"
  VPMM_IRCRlyClose_flg/1 -> VPMM_IRCRlyClose_flg_Inproc/1  "VPMM_IRCRlyClose_flg"
  VPMM_IRCRlyClose_flg_Inproc/1 -> UnitConverter536/1
  UnitConverter536/1 -> VOUTP_IRCRlyClose_flg/1  "VOUTP_IRCRlyClose_flg"
  VPMM_IGNRlyClose_flg/1 -> VPMM_IGNRlyClose_flg_Inproc/1  "VPMM_IGNRlyClose_flg"
  VPMM_IGNRlyClose_flg_Inproc/1 -> UnitConverter537/1
  UnitConverter537/1 -> VOUTP_IGNRlyClose_flg/1  "VOUTP_IGNRlyClose_flg"
  VPMM_BattHVDem_enum/1 -> VPMM_BattHVDem_enum_Inproc/1  "VPMM_BattHVDem_enum"
  VPMM_BattHVDem_enum_Inproc/1 -> UnitConverter538/1
  UnitConverter538/1 -> VOUTP_BattHVDem_enum/1  "VOUTP_BattHVDem_enum"
  VPMM_DCDCRlyDem_enum/1 -> VPMM_DCDCRlyDem_enum_Inproc/1  "VPMM_DCDCRlyDem_enum"
  VPMM_DCDCRlyDem_enum_Inproc/1 -> UnitConverter539/1
  UnitConverter539/1 -> VOUTP_DCDCRlyDem_enum/1  "VOUTP_DCDCRlyDem_enum"
  VPMM_CACRlyDem_enum/1 -> VPMM_CACRlyDem_enum_Inproc/1  "VPMM_CACRlyDem_enum"
  VPMM_CACRlyDem_enum_Inproc/1 -> UnitConverter540/1
  UnitConverter540/1 -> VOUTP_CACRlyDem_enum/1  "VOUTP_CACRlyDem_enum"
  VPMM_MCUHVLoopDem_enum/1 -> VPMM_MCUHVLoopDem_enum_Inproc/1  "VPMM_MCUHVLoopDem_enum"
  VPMM_MCUHVLoopDem_enum_Inproc/1 -> UnitConverter541/1
  UnitConverter541/1 -> VOUTP_MCUHVLoopDem_enum/1  "VOUTP_MCUHVLoopDem_enum"
  VPMM_EHPSRlyDem_enum/1 -> VPMM_EHPSRlyDem_enum_Inproc/1  "VPMM_EHPSRlyDem_enum"
  VPMM_EHPSRlyDem_enum_Inproc/1 -> UnitConverter542/1
  UnitConverter542/1 -> VOUTP_EHPSRlyDem_enum/1  "VOUTP_EHPSRlyDem_enum"
  VPMM_ACHVLoopDem_enum/1 -> VPMM_ACHVLoopDem_enum_Inproc/1  "VPMM_ACHVLoopDem_enum"
  VPMM_ACHVLoopDem_enum_Inproc/1 -> UnitConverter543/1
  UnitConverter543/1 -> VOUTP_ACHVLoopDem_enum/1  "VOUTP_ACHVLoopDem_enum"
  VPMM_HVSysReady_enum/1 -> VPMM_HVSysReady_enum_Inproc/1  "VPMM_HVSysReady_enum"
  VPMM_HVSysReady_enum_Inproc/1 -> UnitConverter544/1
  UnitConverter544/1 -> VOUTP_HVSysReady_enum/1  "VOUTP_HVSysReady_enum"
  VPMM_DrivelineRelease_enum/1 -> VPMM_DrivelineRelease_enum_Inproc/1  "VPMM_DrivelineRelease_enum"
  VPMM_DrivelineRelease_enum_Inproc/1 -> UnitConverter545/1
  UnitConverter545/1 -> VOUTP_DrivelineRelease_enum/1  "VOUTP_DrivelineRelease_enum"
  VPMM_ActiveDischargeReq_enum/1 -> VPMM_ActiveDischargeReq_enum_Inproc/1  "VPMM_ActiveDischargeReq_enum"
  VPMM_ActiveDischargeReq_enum_Inproc/1 -> UnitConverter546/1
  UnitConverter546/1 -> VOUTP_ActiveDischargeReq_enum/1  "VOUTP_ActiveDischargeReq_enum"
  VPMM_VCUMCUEn_flg/1 -> VPMM_VCUMCUEn_flg_Inproc/1  "VPMM_VCUMCUEn_flg"
  VPMM_VCUMCUEn_flg_Inproc/1 -> UnitConverter547/1
  UnitConverter547/1 -> VOUTP_VCUMCUEn_flg/1  "VOUTP_VCUMCUEn_flg"
  VPMM_VCUMCUFailRst_flg/1 -> VPMM_VCUMCUFailRst_flg_Inproc/1  "VPMM_VCUMCUFailRst_flg"
  VPMM_VCUMCUFailRst_flg_Inproc/1 -> UnitConverter548/1
  UnitConverter548/1 -> VOUTP_VCUMCUFailRst_flg/1  "VOUTP_VCUMCUFailRst_flg"
  VPMM_HVILFail_flg/1 -> VPMM_HVILFail_flg_Inproc/1  "VPMM_HVILFail_flg"
  VPMM_HVILFail_flg_Inproc/1 -> UnitConverter549/1
  UnitConverter549/1 -> VOUTP_HVILFail_flg/1  "VOUTP_HVILFail_flg"
  VPMM_LostHVComActivePwrDown_flg/1 -> VPMM_LostHVComActivePwrDown_flg_Inproc/1  "VPMM_LostHVComActivePwrDown_flg"
  VPMM_LostHVComActivePwrDown_flg_Inproc/1 -> UnitConverter550/1
  UnitConverter550/1 -> VOUTP_LostHVComActivePwrDown_flg/1  "VOUTP_LostHVComActivePwrDown_flg"
  VPMM_LVBattLowInd_enum/1 -> VPMM_LVBattLowInd_enum_Inproc/1  "VPMM_LVBattLowInd_enum"
  VPMM_LVBattLowInd_enum_Inproc/1 -> UnitConverter551/1
  UnitConverter551/1 -> VOUTP_LVBattLowInd_enum/1  "VOUTP_LVBattLowInd_enum"
  VPMM_ChrgPowerUpFail_flg/1 -> VPMM_ChrgPowerUpFail_flg_Inproc/1  "VPMM_ChrgPowerUpFail_flg"
  VPMM_ChrgPowerUpFail_flg_Inproc/1 -> UnitConverter552/1
  UnitConverter552/1 -> VOUTP_ChrgPowerUpFail_flg/1  "VOUTP_ChrgPowerUpFail_flg"
  VPMM_ChrgBCUHVFail_flg/1 -> VPMM_ChrgBCUHVFail_flg_Inproc/1  "VPMM_ChrgBCUHVFail_flg"
  VPMM_ChrgBCUHVFail_flg_Inproc/1 -> UnitConverter553/1
  UnitConverter553/1 -> VOUTP_ChrgBCUHVFail_flg/1  "VOUTP_ChrgBCUHVFail_flg"
  VPMM_HVFailureChkPass_flg/1 -> VPMM_HVFailureChkPass_flg_Inproc/1  "VPMM_HVFailureChkPass_flg"
  VPMM_HVFailureChkPass_flg_Inproc/1 -> UnitConverter554/1
  UnitConverter554/1 -> VOUTP_HVFailureChkPass_flg/1  "VOUTP_HVFailureChkPass_flg"
  VPMM_HVILDetectFail_flg/1 -> VPMM_HVILDetectFail_flg_Inproc/1  "VPMM_HVILDetectFail_flg"
  VPMM_HVILDetectFail_flg_Inproc/1 -> UnitConverter555/1
  UnitConverter555/1 -> VOUTP_HVILDetectFail_flg/1  "VOUTP_HVILDetectFail_flg"
  VPMM_V2BLifeSig_cnt/1 -> VPMM_V2BLifeSig_cnt_Inproc/1  "VPMM_V2BLifeSig_cnt"
  VPMM_V2BLifeSig_cnt_Inproc/1 -> UnitConverter556/1
  UnitConverter556/1 -> VOUTP_V2BLifeSig_cnt/1  "VOUTP_V2BLifeSig_cnt"
  VPMM_V2BAux1OnOff_enum/1 -> VPMM_V2BAux1OnOff_enum_Inproc/1  "VPMM_V2BAux1OnOff_enum"
  VPMM_V2BAux1OnOff_enum_Inproc/1 -> UnitConverter557/1
  UnitConverter557/1 -> VOUTP_V2BAux1OnOff_enum/1  "VOUTP_V2BAux1OnOff_enum"
  VPMM_V2BAux2OnOff_enum/1 -> VPMM_V2BAux2OnOff_enum_Inproc/1  "VPMM_V2BAux2OnOff_enum"
  VPMM_V2BAux2OnOff_enum_Inproc/1 -> UnitConverter558/1
  UnitConverter558/1 -> VOUTP_V2BAux2OnOff_enum/1  "VOUTP_V2BAux2OnOff_enum"
  VPMM_V2BAux3OnOff_enum/1 -> VPMM_V2BAux3OnOff_enum_Inproc/1  "VPMM_V2BAux3OnOff_enum"
  VPMM_V2BAux3OnOff_enum_Inproc/1 -> UnitConverter559/1
  UnitConverter559/1 -> VOUTP_V2BAux3OnOff_enum/1  "VOUTP_V2BAux3OnOff_enum"
  VPMM_V2BMainPosRlySta_enum/1 -> VPMM_V2BMainPosRlySta_enum_Inproc/1  "VPMM_V2BMainPosRlySta_enum"
  VPMM_V2BMainPosRlySta_enum_Inproc/1 -> UnitConverter560/1
  UnitConverter560/1 -> VOUTP_V2BMainPosRlySta_enum/1  "VOUTP_V2BMainPosRlySta_enum"
  VPMM_V2BMainPosRlyFit_enum/1 -> VPMM_V2BMainPosRlyFit_enum_Inproc/1  "VPMM_V2BMainPosRlyFit_enum"
  VPMM_V2BMainPosRlyFit_enum_Inproc/1 -> UnitConverter561/1
  UnitConverter561/1 -> VOUTP_V2BMainPosRlyFit_enum/1  "VOUTP_V2BMainPosRlyFit_enum"
  VPMM_V2BACPosRlySta_enum/1 -> VPMM_V2BACPosRlySta_enum_Inproc/1  "VPMM_V2BACPosRlySta_enum"
  VPMM_V2BACPosRlySta_enum_Inproc/1 -> UnitConverter562/1
  UnitConverter562/1 -> VOUTP_V2BACPosRlySta_enum/1  "VOUTP_V2BACPosRlySta_enum"
  VPMM_V2BACPosRlyFit_enum/1 -> VPMM_V2BACPosRlyFit_enum_Inproc/1  "VPMM_V2BACPosRlyFit_enum"
  VPMM_V2BACPosRlyFit_enum_Inproc/1 -> UnitConverter563/1
  UnitConverter563/1 -> VOUTP_V2BACPosRlyFit_enum/1  "VOUTP_V2BACPosRlyFit_enum"
  VPMM_V2BAirPosRlySta_enum/1 -> VPMM_V2BAirPosRlySta_enum_Inproc/1  "VPMM_V2BAirPosRlySta_enum"
  VPMM_V2BAirPosRlySta_enum_Inproc/1 -> UnitConverter564/1
  UnitConverter564/1 -> VOUTP_V2BAirPosRlySta_enum/1  "VOUTP_V2BAirPosRlySta_enum"
  VPMM_V2BAirPosRlyFit_enum/1 -> VPMM_V2BAirPosRlyFit_enum_Inproc/1  "VPMM_V2BAirPosRlyFit_enum"
  VPMM_V2BAirPosRlyFit_enum_Inproc/1 -> UnitConverter565/1
  UnitConverter565/1 -> VOUTP_V2BAirPosRlyFit_enum/1  "VOUTP_V2BAirPosRlyFit_enum"
  VPMM_V2BOilPosRlySta_enum/1 -> VPMM_V2BOilPosRlySta_enum_Inproc/1  "VPMM_V2BOilPosRlySta_enum"
  VPMM_V2BOilPosRlySta_enum_Inproc/1 -> UnitConverter566/1
  UnitConverter566/1 -> VOUTP_V2BOilPosRlySta_enum/1  "VOUTP_V2BOilPosRlySta_enum"
  VPMM_V2BOilPosRlyFit_enum/1 -> VPMM_V2BOilPosRlyFit_enum_Inproc/1  "VPMM_V2BOilPosRlyFit_enum"
  VPMM_V2BOilPosRlyFit_enum_Inproc/1 -> UnitConverter567/1
  UnitConverter567/1 -> VOUTP_V2BOilPosRlyFit_enum/1  "VOUTP_V2BOilPosRlyFit_enum"
  VPMM_V2BDCDCPosRlySta_enum/1 -> VPMM_V2BDCDCPosRlySta_enum_Inproc/1  "VPMM_V2BDCDCPosRlySta_enum"
  VPMM_V2BDCDCPosRlySta_enum_Inproc/1 -> UnitConverter568/1
  UnitConverter568/1 -> VOUTP_V2BDCDCPosRlySta_enum/1  "VOUTP_V2BDCDCPosRlySta_enum"
  VPMM_V2BDCDCPosRlyFit_enum/1 -> VPMM_V2BDCDCPosRlyFit_enum_Inproc/1  "VPMM_V2BDCDCPosRlyFit_enum"
  VPMM_V2BDCDCPosRlyFit_enum_Inproc/1 -> UnitConverter569/1
  UnitConverter569/1 -> VOUTP_V2BDCDCPosRlyFit_enum/1  "VOUTP_V2BDCDCPosRlyFit_enum"
  VPMM_V2BAux1RlySta_enum/1 -> VPMM_V2BAux1RlySta_enum_Inproc/1  "VPMM_V2BAux1RlySta_enum"
  VPMM_V2BAux1RlySta_enum_Inproc/1 -> UnitConverter570/1
  UnitConverter570/1 -> VOUTP_V2BAux1RlySta_enum/1  "VOUTP_V2BAux1RlySta_enum"
  VPMM_V2BAux1RlyFit_enum/1 -> VPMM_V2BAux1RlyFit_enum_Inproc/1  "VPMM_V2BAux1RlyFit_enum"
  VPMM_V2BAux1RlyFit_enum_Inproc/1 -> UnitConverter571/1
  UnitConverter571/1 -> VOUTP_V2BAux1RlyFit_enum/1  "VOUTP_V2BAux1RlyFit_enum"
  VPMM_V2BAux2RlySta_enum/1 -> VPMM_V2BAux2RlySta_enum_Inproc/1  "VPMM_V2BAux2RlySta_enum"
  VPMM_V2BAux2RlySta_enum_Inproc/1 -> UnitConverter572/1
  UnitConverter572/1 -> VOUTP_V2BAux2RlySta_enum/1  "VOUTP_V2BAux2RlySta_enum"
  VPMM_V2BAux2RlyFit_enum/1 -> VPMM_V2BAux2RlyFit_enum_Inproc/1  "VPMM_V2BAux2RlyFit_enum"
  VPMM_V2BAux2RlyFit_enum_Inproc/1 -> UnitConverter573/1
  UnitConverter573/1 -> VOUTP_V2BAux2RlyFit_enum/1  "VOUTP_V2BAux2RlyFit_enum"
  VPMM_V2BAux3RlySta_enum/1 -> VPMM_V2BAux3RlySta_enum_Inproc/1  "VPMM_V2BAux3RlySta_enum"
  VPMM_V2BAux3RlySta_enum_Inproc/1 -> UnitConverter574/1
  UnitConverter574/1 -> VOUTP_V2BAux3RlySta_enum/1  "VOUTP_V2BAux3RlySta_enum"
  VPMM_V2BAux3RlyFit_enum/1 -> VPMM_V2BAux3RlyFit_enum_Inproc/1  "VPMM_V2BAux3RlyFit_enum"
  VPMM_V2BAux3RlyFit_enum_Inproc/1 -> UnitConverter575/1
  UnitConverter575/1 -> VOUTP_V2BAux3RlyFit_enum/1  "VOUTP_V2BAux3RlyFit_enum"
  VPMM_V2BAux4RlySta_enum/1 -> VPMM_V2BAux4RlySta_enum_Inproc/1  "VPMM_V2BAux4RlySta_enum"
  VPMM_V2BAux4RlySta_enum_Inproc/1 -> UnitConverter576/1
  UnitConverter576/1 -> VOUTP_V2BAux4RlySta_enum/1  "VOUTP_V2BAux4RlySta_enum"
  VPMM_V2BAux4RlyFit_enum/1 -> VPMM_V2BAux4RlyFit_enum_Inproc/1  "VPMM_V2BAux4RlyFit_enum"
  VPMM_V2BAux4RlyFit_enum_Inproc/1 -> UnitConverter577/1
  UnitConverter577/1 -> VOUTP_V2BAux4RlyFit_enum/1  "VOUTP_V2BAux4RlyFit_enum"
  VPMM_VCULife1_cnt/1 -> VPMM_VCULife1_cnt_Inproc/1  "VPMM_VCULife1_cnt"
  VPMM_VCULife1_cnt_Inproc/1 -> UnitConverter578/1
  UnitConverter578/1 -> VOUTP_VCULife1_cnt/1  "VOUTP_VCULife1_cnt"
  VPMM_VCULife2_cnt/1 -> VPMM_VCULife2_cnt_Inproc/1  "VPMM_VCULife2_cnt"
  VPMM_VCULife2_cnt_Inproc/1 -> UnitConverter579/1
  UnitConverter579/1 -> VOUTP_VCULife2_cnt/1  "VOUTP_VCULife2_cnt"
  VPMM_VSPFunc_enum/1 -> VPMM_VSPFunc_enum_Inproc/1  "VPMM_VSPFunc_enum"
  VPMM_VSPFunc_enum_Inproc/1 -> UnitConverter580/1
  UnitConverter580/1 -> VOUTP_VSPFunc_enum/1  "VOUTP_VSPFunc_enum"
  VPMM_VSPIGNKeySta_enum/1 -> VPMM_VSPIGNKeySta_enum_Inproc/1  "VPMM_VSPIGNKeySta_enum"
  VPMM_VSPIGNKeySta_enum_Inproc/1 -> UnitConverter581/1
  UnitConverter581/1 -> VOUTP_VSPIGNKeySta_enum/1  "VOUTP_VSPIGNKeySta_enum"
  VPMM_VSPReversed_flg/1 -> VPMM_VSPReversed_flg_Inproc/1  "VPMM_VSPReversed_flg"
  VPMM_VSPReversed_flg_Inproc/1 -> UnitConverter582/1
  UnitConverter582/1 -> VOUTP_VSPReversed_flg/1  "VOUTP_VSPReversed_flg"
  VPMM_VSPTurnRight_enum/1 -> VPMM_VSPTurnRight_enum_Inproc/1  "VPMM_VSPTurnRight_enum"
  VPMM_VSPTurnRight_enum_Inproc/1 -> UnitConverter583/1
  UnitConverter583/1 -> VOUTP_VSPTurnRight_enum/1  "VOUTP_VSPTurnRight_enum"
  VPMM_VSPTurnLeft_enum/1 -> VPMM_VSPTurnLeft_enum_Inproc/1  "VPMM_VSPTurnLeft_enum"
  VPMM_VSPTurnLeft_enum_Inproc/1 -> UnitConverter584/1
  UnitConverter584/1 -> VOUTP_VSPTurnLeft_enum/1  "VOUTP_VSPTurnLeft_enum"
  VPMM_FogTMSRlyCMD_enum/1 -> VPMM_FogTMSRlyCMD_enum_Inproc/1  "VPMM_FogTMSRlyCMD_enum"
  VPMM_FogTMSRlyCMD_enum_Inproc/1 -> UnitConverter585/1
  UnitConverter585/1 -> VOUTP_FogTMSRlyCMD_enum/1  "VOUTP_FogTMSRlyCMD_enum"
  VPMM_DCCurr_A/1 -> VPMM_DCCurr_A_Inproc/1  "VPMM_DCCurr_A"
  VPMM_DCCurr_A_Inproc/1 -> UnitConverter586/1
  UnitConverter586/1 -> VOUTP_DCCurr_A/1  "VOUTP_DCCurr_A"
  VPMM_DCVol_V/1 -> VPMM_DCVol_V_Inproc/1  "VPMM_DCVol_V"
  VPMM_DCVol_V_Inproc/1 -> UnitConverter587/1
  UnitConverter587/1 -> VOUTP_DCVol_V/1  "VOUTP_DCVol_V"
  VPSA_Keystatus_enum/1 -> VPSA_Keystatus_enum_Inproc/1  "VPSA_Keystatus_enum"
  VPSA_Keystatus_enum_Inproc/1 -> UnitConverter588/1
  UnitConverter588/1 -> VOUTP_Keystatus_enum/1  "VOUTP_Keystatus_enum"
  VPSA_EmergencyShutDown_flg/1 -> VPSA_EmergencyShutDown_flg_Inproc/1  "VPSA_EmergencyShutDown_flg"
  VPSA_EmergencyShutDown_flg_Inproc/1 -> UnitConverter589/1
  UnitConverter589/1 -> VOUTP_EmergencyShutDown_flg/1  "VOUTP_EmergencyShutDown_flg"
  VSCP_triggerBAM_flg/1 -> VSCP_triggerBAM_flg_Inproc/1  "VSCP_triggerBAM_flg"
  VSCP_triggerBAM_flg_Inproc/1 -> UnitConverter590/1
  UnitConverter590/1 -> VOUTP_triggerBAM_flg/1  "VOUTP_triggerBAM_flg"
  VSCP_CFGEM1Ctrl_raw/1 -> VSCP_CFGEM1Ctrl_raw_Inproc/1  "VSCP_CFGEM1Ctrl_raw"
  VSCP_CFGEM1Ctrl_raw_Inproc/1 -> UnitConverter591/1
  UnitConverter591/1 -> VOUTP_CFGEM1Ctrl_raw/1  "VOUTP_CFGEM1Ctrl_raw"
  VSCP_CFGEM1BAMTSize_raw/1 -> VSCP_CFGEM1BAMTSize_raw_Inproc/1  "VSCP_CFGEM1BAMTSize_raw"
  VSCP_CFGEM1BAMTSize_raw_Inproc/1 -> UnitConverter592/1
  UnitConverter592/1 -> VOUTP_CFGEM1BAMTSize_raw/1  "VOUTP_CFGEM1BAMTSize_raw"
  VSCP_CFGEM1BAMTNum_raw/1 -> VSCP_CFGEM1BAMTNum_raw_Inproc/1  "VSCP_CFGEM1BAMTNum_raw"
  VSCP_CFGEM1BAMTNum_raw_Inproc/1 -> UnitConverter593/1
  UnitConverter593/1 -> VOUTP_CFGEM1BAMTNum_raw/1  "VOUTP_CFGEM1BAMTNum_raw"
  VSCP_CFGEM1BAMRsv_raw/1 -> VSCP_CFGEM1BAMRsv_raw_Inproc/1  "VSCP_CFGEM1BAMRsv_raw"
  VSCP_CFGEM1BAMRsv_raw_Inproc/1 -> UnitConverter594/1
  UnitConverter594/1 -> VOUTP_CFGEM1BAMRsv_raw/1  "VOUTP_CFGEM1BAMRsv_raw"
  VSCP_CFGEM1BAMPGN_raw/1 -> VSCP_CFGEM1BAMPGN_raw_Inproc/1  "VSCP_CFGEM1BAMPGN_raw"
  VSCP_CFGEM1BAMPGN_raw_Inproc/1 -> UnitConverter595/1
  UnitConverter595/1 -> VOUTP_CFGEM1BAMPGN_raw/1  "VOUTP_CFGEM1BAMPGN_raw"
  VSCP_triggerDT_flg/1 -> VSCP_triggerDT_flg_Inproc/1  "VSCP_triggerDT_flg"
  VSCP_triggerDT_flg_Inproc/1 -> UnitConverter596/1
  UnitConverter596/1 -> VOUTP_triggerDT_flg/1  "VOUTP_triggerDT_flg"
  VSCP_DTbyte0_raw/1 -> VSCP_DTbyte0_raw_Inproc/1  "VSCP_DTbyte0_raw"
  VSCP_DTbyte0_raw_Inproc/1 -> UnitConverter597/1
  UnitConverter597/1 -> VOUTP_DTbyte0_raw/1  "VOUTP_DTbyte0_raw"
  VSCP_DTbyte1_raw/1 -> VSCP_DTbyte1_raw_Inproc/1  "VSCP_DTbyte1_raw"
  VSCP_DTbyte1_raw_Inproc/1 -> UnitConverter598/1
  UnitConverter598/1 -> VOUTP_DTbyte1_raw/1  "VOUTP_DTbyte1_raw"
  VSCP_DTbyte2_raw/1 -> VSCP_DTbyte2_raw_Inproc/1  "VSCP_DTbyte2_raw"
  VSCP_DTbyte2_raw_Inproc/1 -> UnitConverter599/1
  UnitConverter599/1 -> VOUTP_DTbyte2_raw/1  "VOUTP_DTbyte2_raw"
  VSCP_DTbyte3_raw/1 -> VSCP_DTbyte3_raw_Inproc/1  "VSCP_DTbyte3_raw"
  VSCP_DTbyte3_raw_Inproc/1 -> UnitConverter600/1
  UnitConverter600/1 -> VOUTP_DTbyte3_raw/1  "VOUTP_DTbyte3_raw"
  VSCP_DTbyte4_raw/1 -> VSCP_DTbyte4_raw_Inproc/1  "VSCP_DTbyte4_raw"
  VSCP_DTbyte4_raw_Inproc/1 -> UnitConverter601/1
  UnitConverter601/1 -> VOUTP_DTbyte4_raw/1  "VOUTP_DTbyte4_raw"
  VSCP_DTbyte5_raw/1 -> VSCP_DTbyte5_raw_Inproc/1  "VSCP_DTbyte5_raw"
  VSCP_DTbyte5_raw_Inproc/1 -> UnitConverter602/1
  UnitConverter602/1 -> VOUTP_DTbyte5_raw/1  "VOUTP_DTbyte5_raw"
  VSCP_DTbyte6_raw/1 -> VSCP_DTbyte6_raw_Inproc/1  "VSCP_DTbyte6_raw"
  VSCP_DTbyte6_raw_Inproc/1 -> UnitConverter603/1
  UnitConverter603/1 -> VOUTP_DTbyte6_raw/1  "VOUTP_DTbyte6_raw"
  VSCP_DTbyte7_raw/1 -> VSCP_DTbyte7_raw_Inproc/1  "VSCP_DTbyte7_raw"
  VSCP_DTbyte7_raw_Inproc/1 -> UnitConverter604/1
  UnitConverter604/1 -> VOUTP_DTbyte7_raw/1  "VOUTP_DTbyte7_raw"
  VSYS_HWVer1_cnt/1 -> VSYS_HWVer1_cnt_Inproc/1  "VSYS_HWVer1_cnt"
  VSYS_HWVer1_cnt_Inproc/1 -> UnitConverter605/1
  UnitConverter605/1 -> VOUTP_HWVer1_cnt/1  "VOUTP_HWVer1_cnt"
  VSYS_HWVer2_cnt/1 -> VSYS_HWVer2_cnt_Inproc/1  "VSYS_HWVer2_cnt"
  VSYS_HWVer2_cnt_Inproc/1 -> UnitConverter606/1
  UnitConverter606/1 -> VOUTP_HWVer2_cnt/1  "VOUTP_HWVer2_cnt"
  VSYS_HWVer3_cnt/1 -> VSYS_HWVer3_cnt_Inproc/1  "VSYS_HWVer3_cnt"
  VSYS_HWVer3_cnt_Inproc/1 -> UnitConverter607/1
  UnitConverter607/1 -> VOUTP_HWVer3_cnt/1  "VOUTP_HWVer3_cnt"
  VSYS_CarModel1_cnt/1 -> VSYS_CarModel1_cnt_Inproc/1  "VSYS_CarModel1_cnt"
  VSYS_CarModel1_cnt_Inproc/1 -> UnitConverter608/1
  UnitConverter608/1 -> VOUTP_CarModel1_cnt/1  "VOUTP_CarModel1_cnt"
  VSYS_CarModel2_cnt/1 -> VSYS_CarModel2_cnt_Inproc/1  "VSYS_CarModel2_cnt"
  VSYS_CarModel2_cnt_Inproc/1 -> UnitConverter609/1
  UnitConverter609/1 -> VOUTP_CarModel2_cnt/1  "VOUTP_CarModel2_cnt"
  VSYS_CarModel3_cnt/1 -> VSYS_CarModel3_cnt_Inproc/1  "VSYS_CarModel3_cnt"
  VSYS_CarModel3_cnt_Inproc/1 -> UnitConverter610/1
  UnitConverter610/1 -> VOUTP_CarModel3_cnt/1  "VOUTP_CarModel3_cnt"
  VSYS_ECU1_cnt/1 -> VSYS_ECU1_cnt_Inproc/1  "VSYS_ECU1_cnt"
  VSYS_ECU1_cnt_Inproc/1 -> UnitConverter611/1
  UnitConverter611/1 -> VOUTP_ECU1_cnt/1  "VOUTP_ECU1_cnt"
  VSYS_ECU2_cnt/1 -> VSYS_ECU2_cnt_Inproc/1  "VSYS_ECU2_cnt"
  VSYS_ECU2_cnt_Inproc/1 -> UnitConverter612/1
  UnitConverter612/1 -> VOUTP_ECU2_cnt/1  "VOUTP_ECU2_cnt"
  VSYS_Major1_cnt/1 -> VSYS_Major1_cnt_Inproc/1  "VSYS_Major1_cnt"
  VSYS_Major1_cnt_Inproc/1 -> UnitConverter613/1
  UnitConverter613/1 -> VOUTP_Major1_cnt/1  "VOUTP_Major1_cnt"
  VSYS_Major2_cnt/1 -> VSYS_Major2_cnt_Inproc/1  "VSYS_Major2_cnt"
  VSYS_Major2_cnt_Inproc/1 -> UnitConverter614/1
  UnitConverter614/1 -> VOUTP_Major2_cnt/1  "VOUTP_Major2_cnt"
  VSYS_Minor1_cnt/1 -> VSYS_Minor1_cnt_Inproc/1  "VSYS_Minor1_cnt"
  VSYS_Minor1_cnt_Inproc/1 -> UnitConverter615/1
  UnitConverter615/1 -> VOUTP_Minor1_cnt/1  "VOUTP_Minor1_cnt"
  VSYS_Minor2_cnt/1 -> VSYS_Minor2_cnt_Inproc/1  "VSYS_Minor2_cnt"
  VSYS_Minor2_cnt_Inproc/1 -> UnitConverter616/1
  UnitConverter616/1 -> VOUTP_Minor2_cnt/1  "VOUTP_Minor2_cnt"
  VSYS_Patch1_cnt/1 -> VSYS_Patch1_cnt_Inproc/1  "VSYS_Patch1_cnt"
  VSYS_Patch1_cnt_Inproc/1 -> UnitConverter617/1
  UnitConverter617/1 -> VOUTP_Patch1_cnt/1  "VOUTP_Patch1_cnt"
  VSYS_Patch2_cnt/1 -> VSYS_Patch2_cnt_Inproc/1  "VSYS_Patch2_cnt"
  VSYS_Patch2_cnt_Inproc/1 -> UnitConverter618/1
  UnitConverter618/1 -> VOUTP_Patch2_cnt/1  "VOUTP_Patch2_cnt"
  VSYS_Country1_cnt/1 -> VSYS_Country1_cnt_Inproc/1  "VSYS_Country1_cnt"
  VSYS_Country1_cnt_Inproc/1 -> UnitConverter619/1
  UnitConverter619/1 -> VOUTP_Country1_cnt/1  "VOUTP_Country1_cnt"
  VSYS_Country2_cnt/1 -> VSYS_Country2_cnt_Inproc/1  "VSYS_Country2_cnt"
  VSYS_Country2_cnt_Inproc/1 -> UnitConverter620/1
  UnitConverter620/1 -> VOUTP_Country2_cnt/1  "VOUTP_Country2_cnt"
  VSYS_Variation_cnt/1 -> VSYS_Variation_cnt_Inproc/1  "VSYS_Variation_cnt"
  VSYS_Variation_cnt_Inproc/1 -> UnitConverter621/1
  UnitConverter621/1 -> VOUTP_Variation_cnt/1  "VOUTP_Variation_cnt"
  VSYS_Dash1_cnt/1 -> VSYS_Dash1_cnt_Inproc/1  "VSYS_Dash1_cnt"
  VSYS_Dash1_cnt_Inproc/1 -> UnitConverter622/1
  UnitConverter622/1 -> VOUTP_Dash1_cnt/1  "VOUTP_Dash1_cnt"
  VSYS_Change1_cnt/1 -> VSYS_Change1_cnt_Inproc/1  "VSYS_Change1_cnt"
  VSYS_Change1_cnt_Inproc/1 -> UnitConverter623/1
  UnitConverter623/1 -> VOUTP_Change1_cnt/1  "VOUTP_Change1_cnt"
  VSYS_Change2_cnt/1 -> VSYS_Change2_cnt_Inproc/1  "VSYS_Change2_cnt"
  VSYS_Change2_cnt_Inproc/1 -> UnitConverter624/1
  UnitConverter624/1 -> VOUTP_Change2_cnt/1  "VOUTP_Change2_cnt"
  VSYS_Dash2_cnt/1 -> VSYS_Dash2_cnt_Inproc/1  "VSYS_Dash2_cnt"
  VSYS_Dash2_cnt_Inproc/1 -> UnitConverter625/1
  UnitConverter625/1 -> VOUTP_Dash2_cnt/1  "VOUTP_Dash2_cnt"
  VSYS_SHA1_cnt/1 -> VSYS_SHA1_cnt_Inproc/1  "VSYS_SHA1_cnt"
  VSYS_SHA1_cnt_Inproc/1 -> UnitConverter626/1
  UnitConverter626/1 -> VOUTP_SHA1_cnt/1  "VOUTP_SHA1_cnt"
  VSYS_SHA2_cnt/1 -> VSYS_SHA2_cnt_Inproc/1  "VSYS_SHA2_cnt"
  VSYS_SHA2_cnt_Inproc/1 -> UnitConverter627/1
  UnitConverter627/1 -> VOUTP_SHA2_cnt/1  "VOUTP_SHA2_cnt"
  VSYS_SHA3_cnt/1 -> VSYS_SHA3_cnt_Inproc/1  "VSYS_SHA3_cnt"
  VSYS_SHA3_cnt_Inproc/1 -> UnitConverter628/1
  UnitConverter628/1 -> VOUTP_SHA3_cnt/1  "VOUTP_SHA3_cnt"
  VSYS_SHA4_cnt/1 -> VSYS_SHA4_cnt_Inproc/1  "VSYS_SHA4_cnt"
  VSYS_SHA4_cnt_Inproc/1 -> UnitConverter629/1
  UnitConverter629/1 -> VOUTP_SHA4_cnt/1  "VOUTP_SHA4_cnt"
  VSYS_SHA5_cnt/1 -> VSYS_SHA5_cnt_Inproc/1  "VSYS_SHA5_cnt"
  VSYS_SHA5_cnt_Inproc/1 -> UnitConverter630/1
  UnitConverter630/1 -> VOUTP_SHA5_cnt/1  "VOUTP_SHA5_cnt"
  VSYS_SHA6_cnt/1 -> VSYS_SHA6_cnt_Inproc/1  "VSYS_SHA6_cnt"
  VSYS_SHA6_cnt_Inproc/1 -> UnitConverter631/1
  UnitConverter631/1 -> VOUTP_SHA6_cnt/1  "VOUTP_SHA6_cnt"
  VSYS_SHA7_cnt/1 -> VSYS_SHA7_cnt_Inproc/1  "VSYS_SHA7_cnt"
  VSYS_SHA7_cnt_Inproc/1 -> UnitConverter632/1
  UnitConverter632/1 -> VOUTP_SHA7_cnt/1  "VOUTP_SHA7_cnt"
  VSYS_SHA8_cnt/1 -> VSYS_SHA8_cnt_Inproc/1  "VSYS_SHA8_cnt"
  VSYS_SHA8_cnt_Inproc/1 -> UnitConverter633/1
  UnitConverter633/1 -> VOUTP_SHA8_cnt/1  "VOUTP_SHA8_cnt"
  VSYS_NvWriteReqRisingEdge_flg/1 -> VSYS_NvWriteReqRisingEdge_flg_Inproc/1  "VSYS_NvWriteReqRisingEdge_flg"
  VSYS_NvWriteReqRisingEdge_flg_Inproc/1 -> UnitConverter634/1
  UnitConverter634/1 -> VOUTP_NvWriteReqRisingEdge_flg/1  "VOUTP_NvWriteReqRisingEdge_flg"
  VSYS_FdcSlpReqRisingEdge_flg/1 -> VSYS_FdcSlpReqRisingEdge_flg_Inproc/1  "VSYS_FdcSlpReqRisingEdge_flg"
  VSYS_FdcSlpReqRisingEdge_flg_Inproc/1 -> UnitConverter635/1
  UnitConverter635/1 -> VOUTP_FdcSlpReqRisingEdge_flg/1  "VOUTP_FdcSlpReqRisingEdge_flg"
  VSYS_FdcSlpTime_sec/1 -> VSYS_FdcSlpTime_sec_Inproc/1  "VSYS_FdcSlpTime_sec"
  VSYS_FdcSlpTime_sec_Inproc/1 -> UnitConverter636/1
  UnitConverter636/1 -> VOUTP_FdcSlpTime_sec/1  "VOUTP_FdcSlpTime_sec"
  VSYS_PmicBootReason_enum/1 -> VSYS_PmicBootReason_enum_Inproc/1  "VSYS_PmicBootReason_enum"
  VSYS_PmicBootReason_enum_Inproc/1 -> UnitConverter637/1
  UnitConverter637/1 -> VOUTP_PmicBootReason_enum/1  "VOUTP_PmicBootReason_enum"
  VSYS_WisrBootReason_raw32/1 -> VSYS_WisrBootReason_raw32_Inproc/1  "VSYS_WisrBootReason_raw32"
  VSYS_WisrBootReason_raw32_Inproc/1 -> UnitConverter638/1
  UnitConverter638/1 -> VOUTP_WisrBootReason_raw32/1  "VOUTP_WisrBootReason_raw32"
  VSYS_AcoreRebootCmdACK_flg/1 -> VSYS_AcoreRebootCmdACK_flg_Inproc/1  "VSYS_AcoreRebootCmdACK_flg"
  VSYS_AcoreRebootCmdACK_flg_Inproc/1 -> UnitConverter639/1
  UnitConverter639/1 -> VOUTP_AcoreRebootCmdACK_flg/1  "VOUTP_AcoreRebootCmdACK_flg"
  VSYS_CurrentNmState_enum/1 -> VSYS_CurrentNmState_enum_Inproc/1  "VSYS_CurrentNmState_enum"
  VSYS_CurrentNmState_enum_Inproc/1 -> UnitConverter640/1
  UnitConverter640/1 -> VOUTP_CurrentNmState_enum/1  "VOUTP_CurrentNmState_enum"
  VSYS_ECUGen1_cnt/1 -> VSYS_ECUGen1_cnt_Inproc/1  "VSYS_ECUGen1_cnt"
  VSYS_ECUGen1_cnt_Inproc/1 -> UnitConverter641/1
  UnitConverter641/1 -> VOUTP_ECUGen1_cnt/1  "VOUTP_ECUGen1_cnt"
  VSYS_ECUGen2_cnt/1 -> VSYS_ECUGen2_cnt_Inproc/1  "VSYS_ECUGen2_cnt"
  VSYS_ECUGen2_cnt_Inproc/1 -> UnitConverter642/1
  UnitConverter642/1 -> VOUTP_ECUGen2_cnt/1  "VOUTP_ECUGen2_cnt"
  VSYS_PmicBootPath_raw32/1 -> VSYS_PmicBootPath_raw32_Inproc/1  "VSYS_PmicBootPath_raw32"
  VSYS_PmicBootPath_raw32_Inproc/1 -> UnitConverter643/1
  UnitConverter643/1 -> VOUTP_PmicBootPath_raw32/1  "VOUTP_PmicBootPath_raw32"
  VSYS_DrivingMode_cnt/1 -> VSYS_DrivingMode_cnt_Inproc/1  "VSYS_DrivingMode_cnt"
  VSYS_DrivingMode_cnt_Inproc/1 -> UnitConverter644/1
  UnitConverter644/1 -> VOUTP_DrivingMode_cnt/1  "VOUTP_DrivingMode_cnt"
  VSYS_ModelYear_cnt/1 -> VSYS_ModelYear_cnt_Inproc/1  "VSYS_ModelYear_cnt"
  VSYS_ModelYear_cnt_Inproc/1 -> UnitConverter645/1
  UnitConverter645/1 -> VOUTP_ModelYear_cnt/1  "VOUTP_ModelYear_cnt"
  VTHC_EWPPEReq_rpm/1 -> VTHC_EWPPEReq_rpm_Inproc/1  "VTHC_EWPPEReq_rpm"
  VTHC_EWPPEReq_rpm_Inproc/1 -> UnitConverter646/1
  UnitConverter646/1 -> VOUTP_EWPPEReq_rpm/1  "VOUTP_EWPPEReq_rpm"
  VTHC_CoolFanReq_pct/1 -> VTHC_CoolFanReq_pct_Inproc/1  "VTHC_CoolFanReq_pct"
  VTHC_CoolFanReq_pct_Inproc/1 -> UnitConverter647/1
  UnitConverter647/1 -> VOUTP_CoolFanReq_pct/1  "VOUTP_CoolFanReq_pct"
  VTHC_AfterrunningMode_flg/1 -> VTHC_AfterrunningMode_flg_Inproc/1  "VTHC_AfterrunningMode_flg"
  VTHC_AfterrunningMode_flg_Inproc/1 -> UnitConverter648/1
  UnitConverter648/1 -> VOUTP_AfterrunningMode_flg/1  "VOUTP_AfterrunningMode_flg"
  VTPM_LFBatWarn_flg/1 -> VTPM_LFBatWarn_flg_Inproc/1  "VTPM_LFBatWarn_flg"
  VTPM_LFBatWarn_flg_Inproc/1 -> UnitConverter649/1
  UnitConverter649/1 -> VOUTP_LFBatWarn_flg/1  "VOUTP_LFBatWarn_flg"
  VTPM_RFBatWarn_flg/1 -> VTPM_RFBatWarn_flg_Inproc/1  "VTPM_RFBatWarn_flg"
  VTPM_RFBatWarn_flg_Inproc/1 -> UnitConverter650/1
  UnitConverter650/1 -> VOUTP_RFBatWarn_flg/1  "VOUTP_RFBatWarn_flg"
  VTPM_LRBatWarn_flg/1 -> VTPM_LRBatWarn_flg_Inproc/1  "VTPM_LRBatWarn_flg"
  VTPM_LRBatWarn_flg_Inproc/1 -> UnitConverter651/1
  UnitConverter651/1 -> VOUTP_LRBatWarn_flg/1  "VOUTP_LRBatWarn_flg"
  VTPM_RRBatWarn_flg/1 -> VTPM_RRBatWarn_flg_Inproc/1  "VTPM_RRBatWarn_flg"
  VTPM_RRBatWarn_flg_Inproc/1 -> UnitConverter652/1
  UnitConverter652/1 -> VOUTP_RRBatWarn_flg/1  "VOUTP_RRBatWarn_flg"
  VTPM_LFWheelPress_raw8/1 -> VTPM_LFWheelPress_raw8_Inproc/1  "VTPM_LFWheelPress_raw8"
  VTPM_LFWheelPress_raw8_Inproc/1 -> UnitConverter653/1
  UnitConverter653/1 -> VOUTP_LFWheelPress_raw8/1  "VOUTP_LFWheelPress_raw8"
  VTPM_RFWheelPress_raw8/1 -> VTPM_RFWheelPress_raw8_Inproc/1  "VTPM_RFWheelPress_raw8"
  VTPM_RFWheelPress_raw8_Inproc/1 -> UnitConverter654/1
  UnitConverter654/1 -> VOUTP_RFWheelPress_raw8/1  "VOUTP_RFWheelPress_raw8"
  VTPM_LRWheelPress_raw8/1 -> VTPM_LRWheelPress_raw8_Inproc/1  "VTPM_LRWheelPress_raw8"
  VTPM_LRWheelPress_raw8_Inproc/1 -> UnitConverter655/1
  UnitConverter655/1 -> VOUTP_LRWheelPress_raw8/1  "VOUTP_LRWheelPress_raw8"
  VTPM_RRWheelPress_raw8/1 -> VTPM_RRWheelPress_raw8_Inproc/1  "VTPM_RRWheelPress_raw8"
  VTPM_RRWheelPress_raw8_Inproc/1 -> UnitConverter656/1
  UnitConverter656/1 -> VOUTP_RRWheelPress_raw8/1  "VOUTP_RRWheelPress_raw8"
  VTPM_LFWheelTemp_C/1 -> VTPM_LFWheelTemp_C_Inproc/1  "VTPM_LFWheelTemp_C"
  VTPM_LFWheelTemp_C_Inproc/1 -> UnitConverter657/1
  UnitConverter657/1 -> VOUTP_LFWheelTemp_C/1  "VOUTP_LFWheelTemp_C"
  VTPM_RFWheelTemp_C/1 -> VTPM_RFWheelTemp_C_Inproc/1  "VTPM_RFWheelTemp_C"
  VTPM_RFWheelTemp_C_Inproc/1 -> UnitConverter658/1
  UnitConverter658/1 -> VOUTP_RFWheelTemp_C/1  "VOUTP_RFWheelTemp_C"
  VTPM_LRWheelTemp_C/1 -> VTPM_LRWheelTemp_C_Inproc/1  "VTPM_LRWheelTemp_C"
  VTPM_LRWheelTemp_C_Inproc/1 -> UnitConverter659/1
  UnitConverter659/1 -> VOUTP_LRWheelTemp_C/1  "VOUTP_LRWheelTemp_C"
  VTPM_RRWheelTemp_C/1 -> VTPM_RRWheelTemp_C_Inproc/1  "VTPM_RRWheelTemp_C"
  VTPM_RRWheelTemp_C_Inproc/1 -> UnitConverter660/1
  UnitConverter660/1 -> VOUTP_RRWheelTemp_C/1  "VOUTP_RRWheelTemp_C"
  VTPM_LFSensorFail_flg/1 -> VTPM_LFSensorFail_flg_Inproc/1  "VTPM_LFSensorFail_flg"
  VTPM_LFSensorFail_flg_Inproc/1 -> UnitConverter661/1
  UnitConverter661/1 -> VOUTP_LFSensorFail_flg/1  "VOUTP_LFSensorFail_flg"
  VTPM_RFSensorFail_flg/1 -> VTPM_RFSensorFail_flg_Inproc/1  "VTPM_RFSensorFail_flg"
  VTPM_RFSensorFail_flg_Inproc/1 -> UnitConverter662/1
  UnitConverter662/1 -> VOUTP_RFSensorFail_flg/1  "VOUTP_RFSensorFail_flg"
  VTPM_LRSensorFail_flg/1 -> VTPM_LRSensorFail_flg_Inproc/1  "VTPM_LRSensorFail_flg"
  VTPM_LRSensorFail_flg_Inproc/1 -> UnitConverter663/1
  UnitConverter663/1 -> VOUTP_LRSensorFail_flg/1  "VOUTP_LRSensorFail_flg"
  VTPM_RRSensorFail_flg/1 -> VTPM_RRSensorFail_flg_Inproc/1  "VTPM_RRSensorFail_flg"
  VTPM_RRSensorFail_flg_Inproc/1 -> UnitConverter664/1
  UnitConverter664/1 -> VOUTP_RRSensorFail_flg/1  "VOUTP_RRSensorFail_flg"
  VTPM_LFWheelDebug_flg/1 -> VTPM_LFWheelDebug_flg_Inproc/1  "VTPM_LFWheelDebug_flg"
  VTPM_LFWheelDebug_flg_Inproc/1 -> UnitConverter665/1
  UnitConverter665/1 -> VOUTP_LFWheelDebug_flg/1  "VOUTP_LFWheelDebug_flg"
